simulink library "outp"  (R2021b)
(part 7 of 8)

  VOUTP_LFWheelDebug_flg : Outport  Port=593
  VOUTP_LRWheelDebug_flg : Outport  Port=594
  VOUTP_RFWheelDebug_flg : Outport  Port=595
  VOUTP_RRWheelDebug_flg : Outport  Port=596
  VOUTP_TPMSResButtAllow_flg : Outport  Port=597
  VOUTP_TPMSCaliButtAllow_flg : Outport  Port=598
  VOUTP_LFPressIndi_enum : Outport  Port=599
  VOUTP_RFPressIndi_enum : Outport  Port=600
  VOUTP_LRPressIndi_enum : Outport  Port=601
  VOUTP_RRPressIndi_enum : Outport  Port=602
  VOUTP_TPMSWarnIndi_enum : Outport  Port=603
  VOUTP_LFWheelTmpIndi_flg : Outport  Port=604
  VOUTP_RFWheelTmpIndi_flg : Outport  Port=605
  VOUTP_LRWheelTmpIndi_flg : Outport  Port=606
  VOUTP_RRWheelTmpIndi_flg : Outport  Port=607
  VOUTP_LFWheelPSW_raw8 : Outport  Port=608
  VOUTP_LRWheelPSW_raw8 : Outport  Port=609
  VOUTP_RFWheelPSW_raw8 : Outport  Port=610
  VOUTP_RRWheelPSW_raw8 : Outport  Port=611
  VOUTP_CWheelTips_enum : Outport  Port=612
  VOUTP_AutoLTips_enum : Outport  Port=613
  VOUTP_LFSensorMode_flg : Outport  Port=614
  VOUTP_RFSensorMode_flg : Outport  Port=615
  VOUTP_LRSensorMode_flg : Outport  Port=616
  VOUTP_RRSensorMode_flg : Outport  Port=617
  VOUTP_S1ID_raw32 : Outport  Port=618
  VOUTP_S2ID_raw32 : Outport  Port=619
  VOUTP_S3ID_raw32 : Outport  Port=620
  VOUTP_S4ID_raw32 : Outport  Port=621
  VOUTP_S1L_enum : Outport  Port=622
  VOUTP_S2L_enum : Outport  Port=623
  VOUTP_S3L_enum : Outport  Port=624
  VOUTP_S4L_enum : Outport  Port=625
  VOUTP_ALFin_flg : Outport  Port=626
  VOUTP_LFP20_raw8 : Outport  Port=627
  VOUTP_RFP20_raw8 : Outport  Port=628
  VOUTP_LRP20_raw8 : Outport  Port=629
  VOUTP_RRP20_raw8 : Outport  Port=630
  VOUTP_FAT_flg : Outport  Port=631
  VOUTP_IDin_raw32 : Outport  Port=632
  VOUTP_S1WheelDebugALTU_pct : Outport  Port=633
  VOUTP_S2WheelDebugALTU_pct : Outport  Port=634
  VOUTP_S3WheelDebugALTU_pct : Outport  Port=635
  VOUTP_S4WheelDebugALTU_pct : Outport  Port=636
  VOUTP_ID1messageALTU_raw8 : Outport  Port=637
  VOUTP_ID2messageALTU_raw8 : Outport  Port=638
  VOUTP_ID3messageALTU_raw8 : Outport  Port=639
  VOUTP_ID4messageALTU_raw8 : Outport  Port=640
  VOUTP_Chkfin_flg : Outport  Port=641
  VOUTP_SetIDLoc_flg : Outport  Port=642
  VOUTP_TPMSStorge_flg : Outport  Port=643
  VOUTP_ChkStorge_flg : Outport  Port=644
  VOUTP_TPMSResButt_flg : Outport  Port=645
  VOUTP_LFPindi_enum : Outport  Port=646
  VOUTP_RFPind_enum : Outport  Port=647
  VOUTP_LRPindi_enum : Outport  Port=648
  VOUTP_RRPindi_enum : Outport  Port=649
  VOUTP_WriteChkLFID_raw : Outport  Port=650
  VOUTP_WriteChkRFID_raw : Outport  Port=651
  VOUTP_WriteChkLRID_raw : Outport  Port=652
  VOUTP_WriteChkRRID_raw : Outport  Port=653
  VOUTP_WriteChkfinLFID_raw : Outport  Port=654
  VOUTP_WriteChkfinRFID_raw : Outport  Port=655
  VOUTP_WriteChkfinLRID_raw : Outport  Port=656
  VOUTP_WriteChkfinRRID_raw : Outport  Port=657
  VOUTP_Flashchkdatavalid_enum : Outport  Port=658
  VOUTP_Flashdatavalid_enum : Outport  Port=659
  VOUTP_unlearnSfali_flg : Outport  Port=660
  VOUTP_unlearnSfailvalid_enum : Outport  Port=661
  VOUTP_Prepresstempvalid_enum : Outport  Port=662
  VOUTP_FlashS1ID_raw : Outport  Port=663
  VOUTP_FlashS2ID_raw : Outport  Port=664
  VOUTP_FlashS3ID_raw : Outport  Port=665
  VOUTP_FlashS4ID_raw : Outport  Port=666
  VOUTP_FlashIDvalid_enum : Outport  Port=667
  VOUTP_WritingCnt_enum : Outport  Port=668
  VOUTP_TPMSTLCmd_flg : Outport  Port=669
  VOUTP_LProgress_enum : Outport  Port=670
  VOUTP_TPMSSensorIDRegStart_flg : Outport  Port=671
  VOUTP_ModelVersion_raw : Outport  Port=672
  VOUTP_ModelVersionChksum_raw : Outport  Port=673
  VOUTP_ParkRequest_flg : Outport  Port=674
  VOUTP_TqSourceFr_enum : Outport  Port=675
  VOUTP_TqSourceRr_enum : Outport  Port=676
  VOUTP_FrEDUAvailBrkRgnTq_Nm : Outport  Port=677
  VOUTP_RrEDUAvailBrkRgnTq_Nm : Outport  Port=678
  VOUTP_EVDriveMode_enum : Outport  Port=679
  VOUTP_ShiftGearPosn_enum : Outport  Port=680
  VOUTP_PButtonSta_enum : Outport  Port=681
  VOUTP_FrActvDmpDisabReq_flg : Outport  Port=682
  VOUTP_RrActvDmpDisabReq_flg : Outport  Port=683
  VOUTP_FrRgnDecrSta_flg : Outport  Port=684
  VOUTP_RrRgnDecrSta_flg : Outport  Port=685
  VOUTP_DriverWhlTqDemFr_Nm : Outport  Port=686
  VOUTP_DriverWhlTqDemRr_Nm : Outport  Port=687
  VOUTP_FrEDUActTq_Nm : Outport  Port=688
  VOUTP_RrEDUActTq_Nm : Outport  Port=689
  VOUTP_FrEDURolRgnTq_Nm : Outport  Port=690
  VOUTP_RrEDURolRgnTq_Nm : Outport  Port=691
  VOUTP_FrEDUSpd_rpm : Outport  Port=692
  VOUTP_RrEDUSpd_rpm : Outport  Port=693
  VOUTP_FrEDUSpdValid_flg : Outport  Port=694
  VOUTP_FrEDUAvailBrkRgnTqV_flg : Outport  Port=695
  VOUTP_RrEDUSpdValid_flg : Outport  Port=696
  VOUTP_RrEDUAvailBrkRgnTqV_flg : Outport  Port=697
  VOUTP_RgnAbnorSta_flg : Outport  Port=698
  VOUTP_PTCSPermSta_flg : Outport  Port=699
  VOUTP_FrRgnPermSta_flg : Outport  Port=700
  VOUTP_RrRgnPermSta_flg : Outport  Port=701
  VOUTP_FrIdcMin_A : Outport  Port=702
  VOUTP_FrIdcMax_A : Outport  Port=703
  VOUTP_FrUdcMin_V : Outport  Port=704
  VOUTP_FrUdcMax_V : Outport  Port=705
  VOUTP_RrIdcMin_A : Outport  Port=706
  VOUTP_RrIdcMax_A : Outport  Port=707
  VOUTP_RrUdcMin_V : Outport  Port=708
  VOUTP_RrUdcMax_V : Outport  Port=709
  VOUTP_ReBrakeLPReq_flg : Outport  Port=710
  VOUTP_CreepON_flg : Outport  Port=711
  VOUTP_EquivAccPedalSWSta_flg : Outport  Port=712
  VOUTP_DriveProtEn_flg : Outport  Port=713
  VOUTP_ActParkRequest_flg : Outport  Port=714
  VOUTP_IVIPwrLockSta_enum : Outport  Port=715
  VOUTP_OPDHoldLamp_flg : Outport  Port=716
  VOUTP_VehActSpd_kph : Outport  Port=717
  VOUTP_FrTMTqReq_Nm : Outport  Port=718
  VOUTP_RrTMTqReq_Nm : Outport  Port=719
  VOUTP_ReqOBCV2LEna_enum : Outport  Port=720
  VOUTP_ReqV2LIVIPopup_enum : Outport  Port=721
  VOUTP_ACCCtrlAvail_flg : Outport  Port=722
  VOUTP_ACCPedalOvrd_flg : Outport  Port=723
  VOUTP_CCCtrlSta_enum : Outport  Port=724
  VOUTP_CCMSASpdWar_flg : Outport  Port=725
  VOUTP_MSACtrlSta_enum : Outport  Port=726
  VOUTP_APSCtrlAvail_flg : Outport  Port=727
  VOUTP_APSActive_flg : Outport  Port=728
  VOUTP_APSStaSys_enum : Outport  Port=729
  VOUTP_APSDecReqA_flg : Outport  Port=730
  VOUTP_APSDecReq_mps2 : Outport  Port=731
  VOUTP_APSReq_enum : Outport  Port=732
  VOUTP_IMUEnaCmd_flg : Outport  Port=733
  VOUTP_CAASCtrlAvail_flg : Outport  Port=734
  VOUTP_CAASActive_flg : Outport  Port=735
  VOUTP_ExtraMSACtrlSta_enum : Outport  Port=736
  wires:
  VACC_HVTHCMSysAvail_enum/1 -> VACC_HVTHCMSysAvail_enum_Inproc/1  "VACC_HVTHCMSysAvail_enum"
  VACC_HVTHCMSysAvail_enum_Inproc/1 -> UnitConverter1/1
  UnitConverter1/1 -> VOUTP_HVTHCMSysAvail_enum/1  "VOUTP_HVTHCMSysAvail_enum"
  VACC_LVBattVoltSta_enum/1 -> VACC_LVBattVoltSta_enum_Inproc/1  "VACC_LVBattVoltSta_enum"
  VACC_LVBattVoltSta_enum_Inproc/1 -> UnitConverter2/1
  UnitConverter2/1 -> VOUTP_LVBattVoltSta_enum/1  "VOUTP_LVBattVoltSta_enum"
  VACC_VehHVPwrAvail4THCM_W/1 -> VACC_VehHVPwrAvail4THCM_W_Inproc/1  "VACC_VehHVPwrAvail4THCM_W"
  VACC_VehHVPwrAvail4THCM_W_Inproc/1 -> UnitConverter3/1
  UnitConverter3/1 -> VOUTP_VehHVPwrAvail4THCM_W/1  "VOUTP_VehHVPwrAvail4THCM_W"
  VAPM_VehSpeed_kph/1 -> VAPM_VehSpeed_kph_Inproc/1  "VAPM_VehSpeed_kph"
  VAPM_VehSpeed_kph_Inproc/1 -> UnitConverter4/1
  UnitConverter4/1 -> VOUTP_VehSpeed_kph/1  "VOUTP_VehSpeed_kph"
  VAPM_VehSpeedTimeOut_flg/1 -> VAPM_VehSpeedTimeOut_flg_Inproc/1  "VAPM_VehSpeedTimeOut_flg"
  VAPM_VehSpeedTimeOut_flg_Inproc/1 -> UnitConverter5/1
  UnitConverter5/1 -> VOUTP_VehSpeedTimeOut_flg/1  "VOUTP_VehSpeedTimeOut_flg"
  VAPM_FSOffSw_enum/1 -> VAPM_FSOffSw_enum_Inproc/1  "VAPM_FSOffSw_enum"
  VAPM_FSOffSw_enum_Inproc/1 -> UnitConverter6/1
  UnitConverter6/1 -> VOUTP_FSOffSw_enum/1  "VOUTP_FSOffSw_enum"
  VAPM_FSOffSwTimeOut_flg/1 -> VAPM_FSOffSwTimeOut_flg_Inproc/1  "VAPM_FSOffSwTimeOut_flg"
  VAPM_FSOffSwTimeOut_flg_Inproc/1 -> UnitConverter7/1
  UnitConverter7/1 -> VOUTP_FSOffSwTimeOut_flg/1  "VOUTP_FSOffSwTimeOut_flg"
  VAPM_ChrgPlugSta_enum/1 -> VAPM_ChrgPlugSta_enum_Inproc/1  "VAPM_ChrgPlugSta_enum"
  VAPM_ChrgPlugSta_enum_Inproc/1 -> UnitConverter8/1
  UnitConverter8/1 -> VOUTP_ChrgPlugSta_enum/1  "VOUTP_ChrgPlugSta_enum"
  VAPM_PASDRMR_cm/1 -> VAPM_PASDRMR_cm_Inproc/1  "VAPM_PASDRMR_cm"
  VAPM_PASDRMR_cm_Inproc/1 -> UnitConverter9/1
  UnitConverter9/1 -> VOUTP_PASDRMR_cm/1  "VOUTP_PASDRMR_cm"
  VAPM_PASDRML_cm/1 -> VAPM_PASDRML_cm_Inproc/1  "VAPM_PASDRML_cm"
  VAPM_PASDRML_cm_Inproc/1 -> UnitConverter10/1
  UnitConverter10/1 -> VOUTP_PASDRML_cm/1  "VOUTP_PASDRML_cm"
  VAPM_PASDRCR_cm/1 -> VAPM_PASDRCR_cm_Inproc/1  "VAPM_PASDRCR_cm"
  VAPM_PASDRCR_cm_Inproc/1 -> UnitConverter11/1
  UnitConverter11/1 -> VOUTP_PASDRCR_cm/1  "VOUTP_PASDRCR_cm"
  VAPM_PASDRCL_cm/1 -> VAPM_PASDRCL_cm_Inproc/1  "VAPM_PASDRCL_cm"
  VAPM_PASDRCL_cm_Inproc/1 -> UnitConverter12/1
  UnitConverter12/1 -> VOUTP_PASDRCL_cm/1  "VOUTP_PASDRCL_cm"
  VAPM_PASDFMR_cm/1 -> VAPM_PASDFMR_cm_Inproc/1  "VAPM_PASDFMR_cm"
  VAPM_PASDFMR_cm_Inproc/1 -> UnitConverter13/1
  UnitConverter13/1 -> VOUTP_PASDFMR_cm/1  "VOUTP_PASDFMR_cm"
  VAPM_PASDFML_cm/1 -> VAPM_PASDFML_cm_Inproc/1  "VAPM_PASDFML_cm"
  VAPM_PASDFML_cm_Inproc/1 -> UnitConverter14/1
  UnitConverter14/1 -> VOUTP_PASDFML_cm/1  "VOUTP_PASDFML_cm"
  VAPM_PASDFCR_cm/1 -> VAPM_PASDFCR_cm_Inproc/1  "VAPM_PASDFCR_cm"
  VAPM_PASDFCR_cm_Inproc/1 -> UnitConverter15/1
  UnitConverter15/1 -> VOUTP_PASDFCR_cm/1  "VOUTP_PASDFCR_cm"
  VAPM_PASDFCL_cm/1 -> VAPM_PASDFCL_cm_Inproc/1  "VAPM_PASDFCL_cm"
  VAPM_PASDFCL_cm_Inproc/1 -> UnitConverter16/1
  UnitConverter16/1 -> VOUTP_PASDFCL_cm/1  "VOUTP_PASDFCL_cm"
  VAPM_APSDRLR_cm/1 -> VAPM_APSDRLR_cm_Inproc/1  "VAPM_APSDRLR_cm"
  VAPM_APSDRLR_cm_Inproc/1 -> UnitConverter17/1
  UnitConverter17/1 -> VOUTP_APSDRLR_cm/1  "VOUTP_APSDRLR_cm"
  VAPM_APSDRLL_cm/1 -> VAPM_APSDRLL_cm_Inproc/1  "VAPM_APSDRLL_cm"
  VAPM_APSDRLL_cm_Inproc/1 -> UnitConverter18/1
  UnitConverter18/1 -> VOUTP_APSDRLL_cm/1  "VOUTP_APSDRLL_cm"
  VAPM_APSDFLR_cm/1 -> VAPM_APSDFLR_cm_Inproc/1  "VAPM_APSDFLR_cm"
  VAPM_APSDFLR_cm_Inproc/1 -> UnitConverter19/1
  UnitConverter19/1 -> VOUTP_APSDFLR_cm/1  "VOUTP_APSDFLR_cm"
  VAPM_APSDFLL_cm/1 -> VAPM_APSDFLL_cm_Inproc/1  "VAPM_APSDFLL_cm"
  VAPM_APSDFLL_cm_Inproc/1 -> UnitConverter20/1
  UnitConverter20/1 -> VOUTP_APSDFLL_cm/1  "VOUTP_APSDFLL_cm"
  VAPM_PASAFCL_enum/1 -> VAPM_PASAFCL_enum_Inproc/1  "VAPM_PASAFCL_enum"
  VAPM_PASAFCL_enum_Inproc/1 -> UnitConverter21/1
  UnitConverter21/1 -> VOUTP_PASAFCL_enum/1  "VOUTP_PASAFCL_enum"
  VAPM_PASARMR_enum/1 -> VAPM_PASARMR_enum_Inproc/1  "VAPM_PASARMR_enum"
  VAPM_PASARMR_enum_Inproc/1 -> UnitConverter22/1
  UnitConverter22/1 -> VOUTP_PASARMR_enum/1  "VOUTP_PASARMR_enum"
  VAPM_PASARML_enum/1 -> VAPM_PASARML_enum_Inproc/1  "VAPM_PASARML_enum"
  VAPM_PASARML_enum_Inproc/1 -> UnitConverter23/1
  UnitConverter23/1 -> VOUTP_PASARML_enum/1  "VOUTP_PASARML_enum"
  VAPM_PASARCR_enum/1 -> VAPM_PASARCR_enum_Inproc/1  "VAPM_PASARCR_enum"
  VAPM_PASARCR_enum_Inproc/1 -> UnitConverter24/1
  UnitConverter24/1 -> VOUTP_PASARCR_enum/1  "VOUTP_PASARCR_enum"
  VAPM_PASARCL_enum/1 -> VAPM_PASARCL_enum_Inproc/1  "VAPM_PASARCL_enum"
  VAPM_PASARCL_enum_Inproc/1 -> UnitConverter25/1
  UnitConverter25/1 -> VOUTP_PASARCL_enum/1  "VOUTP_PASARCL_enum"
  VAPM_PASAFMR_enum/1 -> VAPM_PASAFMR_enum_Inproc/1  "VAPM_PASAFMR_enum"
  VAPM_PASAFMR_enum_Inproc/1 -> UnitConverter26/1
  UnitConverter26/1 -> VOUTP_PASAFMR_enum/1  "VOUTP_PASAFMR_enum"
  VAPM_PASAFML_enum/1 -> VAPM_PASAFML_enum_Inproc/1  "VAPM_PASAFML_enum"
  VAPM_PASAFML_enum_Inproc/1 -> UnitConverter27/1
  UnitConverter27/1 -> VOUTP_PASAFML_enum/1  "VOUTP_PASAFML_enum"
  VAPM_PASAFCR_enum/1 -> VAPM_PASAFCR_enum_Inproc/1  "VAPM_PASAFCR_enum"
  VAPM_PASAFCR_enum_Inproc/1 -> UnitConverter28/1
  UnitConverter28/1 -> VOUTP_PASAFCR_enum/1  "VOUTP_PASAFCR_enum"
  VAPM_USSStaRMR_flg/1 -> VAPM_USSStaRMR_flg_Inproc/1  "VAPM_USSStaRMR_flg"
  VAPM_USSStaRMR_flg_Inproc/1 -> UnitConverter29/1
  UnitConverter29/1 -> VOUTP_USSStaRMR_flg/1  "VOUTP_USSStaRMR_flg"
  VAPM_USSStaRML_flg/1 -> VAPM_USSStaRML_flg_Inproc/1  "VAPM_USSStaRML_flg"
  VAPM_USSStaRML_flg_Inproc/1 -> UnitConverter30/1
  UnitConverter30/1 -> VOUTP_USSStaRML_flg/1  "VOUTP_USSStaRML_flg"
  VAPM_USSStaRLR_flg/1 -> VAPM_USSStaRLR_flg_Inproc/1  "VAPM_USSStaRLR_flg"
  VAPM_USSStaRLR_flg_Inproc/1 -> UnitConverter31/1
  UnitConverter31/1 -> VOUTP_USSStaRLR_flg/1  "VOUTP_USSStaRLR_flg"
  VAPM_USSStaRLL_flg/1 -> VAPM_USSStaRLL_flg_Inproc/1  "VAPM_USSStaRLL_flg"
  VAPM_USSStaRLL_flg_Inproc/1 -> UnitConverter32/1
  UnitConverter32/1 -> VOUTP_USSStaRLL_flg/1  "VOUTP_USSStaRLL_flg"
  VAPM_USSStaRCR_flg/1 -> VAPM_USSStaRCR_flg_Inproc/1  "VAPM_USSStaRCR_flg"
  VAPM_USSStaRCR_flg_Inproc/1 -> UnitConverter33/1
  UnitConverter33/1 -> VOUTP_USSStaRCR_flg/1  "VOUTP_USSStaRCR_flg"
  VAPM_USSStaRCL_flg/1 -> VAPM_USSStaRCL_flg_Inproc/1  "VAPM_USSStaRCL_flg"
  VAPM_USSStaRCL_flg_Inproc/1 -> UnitConverter34/1
  UnitConverter34/1 -> VOUTP_USSStaRCL_flg/1  "VOUTP_USSStaRCL_flg"
  VAPM_USSStaFMR_flg/1 -> VAPM_USSStaFMR_flg_Inproc/1  "VAPM_USSStaFMR_flg"
  VAPM_USSStaFMR_flg_Inproc/1 -> UnitConverter35/1
  UnitConverter35/1 -> VOUTP_USSStaFMR_flg/1  "VOUTP_USSStaFMR_flg"
  VAPM_USSStaFML_flg/1 -> VAPM_USSStaFML_flg_Inproc/1  "VAPM_USSStaFML_flg"
  VAPM_USSStaFML_flg_Inproc/1 -> UnitConverter36/1
  UnitConverter36/1 -> VOUTP_USSStaFML_flg/1  "VOUTP_USSStaFML_flg"
  VAPM_USSStaFLR_flg/1 -> VAPM_USSStaFLR_flg_Inproc/1  "VAPM_USSStaFLR_flg"
  VAPM_USSStaFLR_flg_Inproc/1 -> UnitConverter37/1
  UnitConverter37/1 -> VOUTP_USSStaFLR_flg/1  "VOUTP_USSStaFLR_flg"
  VAPM_USSStaFLL_flg/1 -> VAPM_USSStaFLL_flg_Inproc/1  "VAPM_USSStaFLL_flg"
  VAPM_USSStaFLL_flg_Inproc/1 -> UnitConverter38/1
  UnitConverter38/1 -> VOUTP_USSStaFLL_flg/1  "VOUTP_USSStaFLL_flg"
  VAPM_USSStaFCR_flg/1 -> VAPM_USSStaFCR_flg_Inproc/1  "VAPM_USSStaFCR_flg"
  VAPM_USSStaFCR_flg_Inproc/1 -> UnitConverter39/1
  UnitConverter39/1 -> VOUTP_USSStaFCR_flg/1  "VOUTP_USSStaFCR_flg"
  VAPM_USSStaFCL_flg/1 -> VAPM_USSStaFCL_flg_Inproc/1  "VAPM_USSStaFCL_flg"
  VAPM_USSStaFCL_flg_Inproc/1 -> UnitConverter40/1
  UnitConverter40/1 -> VOUTP_USSStaFCL_flg/1  "VOUTP_USSStaFCL_flg"
  VAPM_Chime_enum/1 -> VAPM_Chime_enum_Inproc/1  "VAPM_Chime_enum"
  VAPM_Chime_enum_Inproc/1 -> UnitConverter41/1
  UnitConverter41/1 -> VOUTP_Chime_enum/1  "VOUTP_Chime_enum"
  VAPM_SNSRLayout_enum/1 -> VAPM_SNSRLayout_enum_Inproc/1  "VAPM_SNSRLayout_enum"
  VAPM_SNSRLayout_enum_Inproc/1 -> UnitConverter42/1
  UnitConverter42/1 -> VOUTP_SNSRLayout_enum/1  "VOUTP_SNSRLayout_enum"
  VAPM_StaFSya_flg/1 -> VAPM_StaFSya_flg_Inproc/1  "VAPM_StaFSya_flg"
  VAPM_StaFSya_flg_Inproc/1 -> UnitConverter43/1
  UnitConverter43/1 -> VOUTP_StaFSya_flg/1  "VOUTP_StaFSya_flg"
  VAPM_ModOperation_enum/1 -> VAPM_ModOperation_enum_Inproc/1  "VAPM_ModOperation_enum"
  VAPM_ModOperation_enum_Inproc/1 -> UnitConverter44/1
  UnitConverter44/1 -> VOUTP_ModOperation_enum/1  "VOUTP_ModOperation_enum"
  VAPM_BrkPedalPos_pct/1 -> VAPM_BrkPedalPos_pct_Inproc/1  "VAPM_BrkPedalPos_pct"
  VAPM_BrkPedalPos_pct_Inproc/1 -> UnitConverter45/1
  UnitConverter45/1 -> VOUTP_BrkPedalPos_pct/1  "VOUTP_BrkPedalPos_pct"
  VAPM_BrkPedalPosTimeOut_flg/1 -> VAPM_BrkPedalPosTimeOut_flg_Inproc/1  "VAPM_BrkPedalPosTimeOut_flg"
  VAPM_BrkPedalPosTimeOut_flg_Inproc/1 -> UnitConverter46/1
  UnitConverter46/1 -> VOUTP_BrkPedalPosTimeOut_flg/1  "VOUTP_BrkPedalPosTimeOut_flg"
  VAPM_LFRawWhlSpeed_kph/1 -> VAPM_LFRawWhlSpeed_kph_Inproc/1  "VAPM_LFRawWhlSpeed_kph"
  VAPM_LFRawWhlSpeed_kph_Inproc/1 -> UnitConverter47/1
  UnitConverter47/1 -> VOUTP_LFRawWhlSpeed_kph/1  "VOUTP_LFRawWhlSpeed_kph"
  VAPM_LFRawWhlSpeedTimeOut_flg/1 -> VAPM_LFRawWhlSpeedTimeOut_flg_Inproc/1  "VAPM_LFRawWhlSpeedTimeOut_flg"
  VAPM_LFRawWhlSpeedTimeOut_flg_Inproc/1 -> UnitConverter48/1
  UnitConverter48/1 -> VOUTP_LFRawWhlSpeedTimeOut_flg/1  "VOUTP_LFRawWhlSpeedTimeOut_flg"
  VAPM_RFRawWhlSpeed_kph/1 -> VAPM_RFRawWhlSpeed_kph_Inproc/1  "VAPM_RFRawWhlSpeed_kph"
  VAPM_RFRawWhlSpeed_kph_Inproc/1 -> UnitConverter49/1
  UnitConverter49/1 -> VOUTP_RFRawWhlSpeed_kph/1  "VOUTP_RFRawWhlSpeed_kph"
  VAPM_RFRawWhlSpeedTimeOut_flg/1 -> VAPM_RFRawWhlSpeedTimeOut_flg_Inproc/1  "VAPM_RFRawWhlSpeedTimeOut_flg"
  VAPM_RFRawWhlSpeedTimeOut_flg_Inproc/1 -> UnitConverter50/1
  UnitConverter50/1 -> VOUTP_RFRawWhlSpeedTimeOut_flg/1  "VOUTP_RFRawWhlSpeedTimeOut_flg"
  VAPM_LRRawWhlSpeed_kph/1 -> VAPM_LRRawWhlSpeed_kph_Inproc/1  "VAPM_LRRawWhlSpeed_kph"
  VAPM_LRRawWhlSpeed_kph_Inproc/1 -> UnitConverter51/1
  UnitConverter51/1 -> VOUTP_LRRawWhlSpeed_kph/1  "VOUTP_LRRawWhlSpeed_kph"
  VAPM_LRRawWhlSpeedTimeOut_flg/1 -> VAPM_LRRawWhlSpeedTimeOut_flg_Inproc/1  "VAPM_LRRawWhlSpeedTimeOut_flg"
  VAPM_LRRawWhlSpeedTimeOut_flg_Inproc/1 -> UnitConverter52/1
  UnitConverter52/1 -> VOUTP_LRRawWhlSpeedTimeOut_flg/1  "VOUTP_LRRawWhlSpeedTimeOut_flg"
  VAPM_RRRawWhlSpeed_kph/1 -> VAPM_RRRawWhlSpeed_kph_Inproc/1  "VAPM_RRRawWhlSpeed_kph"
  VAPM_RRRawWhlSpeed_kph_Inproc/1 -> UnitConverter53/1
  UnitConverter53/1 -> VOUTP_RRRawWhlSpeed_kph/1  "VOUTP_RRRawWhlSpeed_kph"
  VAPM_RRRawWhlSpeedTimeOut_flg/1 -> VAPM_RRRawWhlSpeedTimeOut_flg_Inproc/1  "VAPM_RRRawWhlSpeedTimeOut_flg"
  VAPM_RRRawWhlSpeedTimeOut_flg_Inproc/1 -> UnitConverter54/1
  UnitConverter54/1 -> VOUTP_RRRawWhlSpeedTimeOut_flg/1  "VOUTP_RRRawWhlSpeedTimeOut_flg"
  VAPM_LFRawWhlSpeedV_flg/1 -> VAPM_LFRawWhlSpeedV_flg_Inproc/1  "VAPM_LFRawWhlSpeedV_flg"
  VAPM_LFRawWhlSpeedV_flg_Inproc/1 -> UnitConverter55/1
  UnitConverter55/1 -> VOUTP_LFRawWhlSpeedV_flg/1  "VOUTP_LFRawWhlSpeedV_flg"
  VAPM_LFRawWhlSpeedVTimeOut_flg/1 -> VAPM_LFRawWhlSpeedVTimeOut_flg_Inproc/1  "VAPM_LFRawWhlSpeedVTimeOut_flg"
  VAPM_LFRawWhlSpeedVTimeOut_flg_Inproc/1 -> UnitConverter56/1
  UnitConverter56/1 -> VOUTP_LFRawWhlSpeedVTimeOut_flg/1  "VOUTP_LFRawWhlSpeedVTimeOut_flg"
  VAPM_RFRawWhlSpeedV_flg/1 -> VAPM_RFRawWhlSpeedV_flg_Inproc/1  "VAPM_RFRawWhlSpeedV_flg"
  VAPM_RFRawWhlSpeedV_flg_Inproc/1 -> UnitConverter57/1
  UnitConverter57/1 -> VOUTP_RFRawWhlSpeedV_flg/1  "VOUTP_RFRawWhlSpeedV_flg"
  VAPM_RFRawWhlSpeedVTimeOut_flg/1 -> VAPM_RFRawWhlSpeedVTimeOut_flg_Inproc/1  "VAPM_RFRawWhlSpeedVTimeOut_flg"
  VAPM_RFRawWhlSpeedVTimeOut_flg_Inproc/1 -> UnitConverter58/1
  UnitConverter58/1 -> VOUTP_RFRawWhlSpeedVTimeOut_flg/1  "VOUTP_RFRawWhlSpeedVTimeOut_flg"
  VAPM_LRRawWhlSpeedV_flg/1 -> VAPM_LRRawWhlSpeedV_flg_Inproc/1  "VAPM_LRRawWhlSpeedV_flg"
  VAPM_LRRawWhlSpeedV_flg_Inproc/1 -> UnitConverter59/1
  UnitConverter59/1 -> VOUTP_LRRawWhlSpeedV_flg/1  "VOUTP_LRRawWhlSpeedV_flg"
  VAPM_LRRawWhlSpeedVTimeOut_flg/1 -> VAPM_LRRawWhlSpeedVTimeOut_flg_Inproc/1  "VAPM_LRRawWhlSpeedVTimeOut_flg"
  VAPM_LRRawWhlSpeedVTimeOut_flg_Inproc/1 -> UnitConverter60/1
  UnitConverter60/1 -> VOUTP_LRRawWhlSpeedVTimeOut_flg/1  "VOUTP_LRRawWhlSpeedVTimeOut_flg"
  VAPM_RRRawWhlSpeedV_flg/1 -> VAPM_RRRawWhlSpeedV_flg_Inproc/1  "VAPM_RRRawWhlSpeedV_flg"
  VAPM_RRRawWhlSpeedV_flg_Inproc/1 -> UnitConverter61/1
  UnitConverter61/1 -> VOUTP_RRRawWhlSpeedV_flg/1  "VOUTP_RRRawWhlSpeedV_flg"
  VAPM_RRRawWhlSpeedVTimeOut_flg/1 -> VAPM_RRRawWhlSpeedVTimeOut_flg_Inproc/1  "VAPM_RRRawWhlSpeedVTimeOut_flg"
  VAPM_RRRawWhlSpeedVTimeOut_flg_Inproc/1 -> UnitConverter62/1
  UnitConverter62/1 -> VOUTP_RRRawWhlSpeedVTimeOut_flg/1  "VOUTP_RRRawWhlSpeedVTimeOut_flg"
  VAPM_LFWhlRotDir_enum/1 -> VAPM_LFWhlRotDir_enum_Inproc/1  "VAPM_LFWhlRotDir_enum"
  VAPM_LFWhlRotDir_enum_Inproc/1 -> UnitConverter63/1
  UnitConverter63/1 -> VOUTP_LFWhlRotDir_enum/1  "VOUTP_LFWhlRotDir_enum"
  VAPM_LFWhlRotDirTimeOut_flg/1 -> VAPM_LFWhlRotDirTimeOut_flg_Inproc/1  "VAPM_LFWhlRotDirTimeOut_flg"
  VAPM_LFWhlRotDirTimeOut_flg_Inproc/1 -> UnitConverter64/1
  UnitConverter64/1 -> VOUTP_LFWhlRotDirTimeOut_flg/1  "VOUTP_LFWhlRotDirTimeOut_flg"
  VAPM_RFWhlRotDir_enum/1 -> VAPM_RFWhlRotDir_enum_Inproc/1  "VAPM_RFWhlRotDir_enum"
  VAPM_RFWhlRotDir_enum_Inproc/1 -> UnitConverter65/1
  UnitConverter65/1 -> VOUTP_RFWhlRotDir_enum/1  "VOUTP_RFWhlRotDir_enum"
  VAPM_RFWhlRotDirTimeOut_flg/1 -> VAPM_RFWhlRotDirTimeOut_flg_Inproc/1  "VAPM_RFWhlRotDirTimeOut_flg"
  VAPM_RFWhlRotDirTimeOut_flg_Inproc/1 -> UnitConverter66/1
  UnitConverter66/1 -> VOUTP_RFWhlRotDirTimeOut_flg/1  "VOUTP_RFWhlRotDirTimeOut_flg"
  VAPM_LRWhlRotDir_enum/1 -> VAPM_LRWhlRotDir_enum_Inproc/1  "VAPM_LRWhlRotDir_enum"
  VAPM_LRWhlRotDir_enum_Inproc/1 -> UnitConverter67/1
  UnitConverter67/1 -> VOUTP_LRWhlRotDir_enum/1  "VOUTP_LRWhlRotDir_enum"
  VAPM_LRWhlRotDirTimeOut_flg/1 -> VAPM_LRWhlRotDirTimeOut_flg_Inproc/1  "VAPM_LRWhlRotDirTimeOut_flg"
  VAPM_LRWhlRotDirTimeOut_flg_Inproc/1 -> UnitConverter68/1
  UnitConverter68/1 -> VOUTP_LRWhlRotDirTimeOut_flg/1  "VOUTP_LRWhlRotDirTimeOut_flg"
  VAPM_RRWhlRotDir_enum/1 -> VAPM_RRWhlRotDir_enum_Inproc/1  "VAPM_RRWhlRotDir_enum"
  VAPM_RRWhlRotDir_enum_Inproc/1 -> UnitConverter69/1
  UnitConverter69/1 -> VOUTP_RRWhlRotDir_enum/1  "VOUTP_RRWhlRotDir_enum"
  VAPM_RRWhlRotDirTimeOut_flg/1 -> VAPM_RRWhlRotDirTimeOut_flg_Inproc/1  "VAPM_RRWhlRotDirTimeOut_flg"
  VAPM_RRWhlRotDirTimeOut_flg_Inproc/1 -> UnitConverter70/1
  UnitConverter70/1 -> VOUTP_RRWhlRotDirTimeOut_flg/1  "VOUTP_RRWhlRotDirTimeOut_flg"
  VAPM_LFPulseCountV_flg/1 -> VAPM_LFPulseCountV_flg_Inproc/1  "VAPM_LFPulseCountV_flg"
  VAPM_LFPulseCountV_flg_Inproc/1 -> UnitConverter71/1
  UnitConverter71/1 -> VOUTP_LFPulseCountV_flg/1  "VOUTP_LFPulseCountV_flg"
  VAPM_LFPulseCountVTimeOut_flg/1 -> VAPM_LFPulseCountVTimeOut_flg_Inproc/1  "VAPM_LFPulseCountVTimeOut_flg"
  VAPM_LFPulseCountVTimeOut_flg_Inproc/1 -> UnitConverter72/1
  UnitConverter72/1 -> VOUTP_LFPulseCountVTimeOut_flg/1  "VOUTP_LFPulseCountVTimeOut_flg"
  VAPM_RFPulseCountV_flg/1 -> VAPM_RFPulseCountV_flg_Inproc/1  "VAPM_RFPulseCountV_flg"
  VAPM_RFPulseCountV_flg_Inproc/1 -> UnitConverter73/1
  UnitConverter73/1 -> VOUTP_RFPulseCountV_flg/1  "VOUTP_RFPulseCountV_flg"
  VAPM_RFPulseCountVTimeOut_flg/1 -> VAPM_RFPulseCountVTimeOut_flg_Inproc/1  "VAPM_RFPulseCountVTimeOut_flg"
  VAPM_RFPulseCountVTimeOut_flg_Inproc/1 -> UnitConverter74/1
  UnitConverter74/1 -> VOUTP_RFPulseCountVTimeOut_flg/1  "VOUTP_RFPulseCountVTimeOut_flg"
  VAPM_LRPulseCountV_flg/1 -> VAPM_LRPulseCountV_flg_Inproc/1  "VAPM_LRPulseCountV_flg"
  VAPM_LRPulseCountV_flg_Inproc/1 -> UnitConverter75/1
  UnitConverter75/1 -> VOUTP_LRPulseCountV_flg/1  "VOUTP_LRPulseCountV_flg"
  VAPM_LRPulseCountVTimeOut_flg/1 -> VAPM_LRPulseCountVTimeOut_flg_Inproc/1  "VAPM_LRPulseCountVTimeOut_flg"
  VAPM_LRPulseCountVTimeOut_flg_Inproc/1 -> UnitConverter76/1
  UnitConverter76/1 -> VOUTP_LRPulseCountVTimeOut_flg/1  "VOUTP_LRPulseCountVTimeOut_flg"
  VAPM_RRPulseCountV_flg/1 -> VAPM_RRPulseCountV_flg_Inproc/1  "VAPM_RRPulseCountV_flg"
  VAPM_RRPulseCountV_flg_Inproc/1 -> UnitConverter77/1
  UnitConverter77/1 -> VOUTP_RRPulseCountV_flg/1  "VOUTP_RRPulseCountV_flg"
  VAPM_RRPulseCountVTimeOut_flg/1 -> VAPM_RRPulseCountVTimeOut_flg_Inproc/1  "VAPM_RRPulseCountVTimeOut_flg"
  VAPM_RRPulseCountVTimeOut_flg_Inproc/1 -> UnitConverter78/1
  UnitConverter78/1 -> VOUTP_RRPulseCountVTimeOut_flg/1  "VOUTP_RRPulseCountVTimeOut_flg"
  VAPM_LFPulseCount_enum/1 -> VAPM_LFPulseCount_enum_Inproc/1  "VAPM_LFPulseCount_enum"
  VAPM_LFPulseCount_enum_Inproc/1 -> UnitConverter79/1
  UnitConverter79/1 -> VOUTP_LFPulseCount_enum/1  "VOUTP_LFPulseCount_enum"
  VAPM_LFPulseCountTimeOut_flg/1 -> VAPM_LFPulseCountTimeOut_flg_Inproc/1  "VAPM_LFPulseCountTimeOut_flg"
  VAPM_LFPulseCountTimeOut_flg_Inproc/1 -> UnitConverter80/1
  UnitConverter80/1 -> VOUTP_LFPulseCountTimeOut_flg/1  "VOUTP_LFPulseCountTimeOut_flg"
  VAPM_RFPulseCount_enum/1 -> VAPM_RFPulseCount_enum_Inproc/1  "VAPM_RFPulseCount_enum"
  VAPM_RFPulseCount_enum_Inproc/1 -> UnitConverter81/1
  UnitConverter81/1 -> VOUTP_RFPulseCount_enum/1  "VOUTP_RFPulseCount_enum"
  VAPM_RFPulseCountTimeOut_flg/1 -> VAPM_RFPulseCountTimeOut_flg_Inproc/1  "VAPM_RFPulseCountTimeOut_flg"
  VAPM_RFPulseCountTimeOut_flg_Inproc/1 -> UnitConverter82/1
  UnitConverter82/1 -> VOUTP_RFPulseCountTimeOut_flg/1  "VOUTP_RFPulseCountTimeOut_flg"
  VAPM_LRPulseCount_enum/1 -> VAPM_LRPulseCount_enum_Inproc/1  "VAPM_LRPulseCount_enum"
  VAPM_LRPulseCount_enum_Inproc/1 -> UnitConverter83/1
  UnitConverter83/1 -> VOUTP_LRPulseCount_enum/1  "VOUTP_LRPulseCount_enum"
  VAPM_LRPulseCountTimeOut_flg/1 -> VAPM_LRPulseCountTimeOut_flg_Inproc/1  "VAPM_LRPulseCountTimeOut_flg"
  VAPM_LRPulseCountTimeOut_flg_Inproc/1 -> UnitConverter84/1
  UnitConverter84/1 -> VOUTP_LRPulseCountTimeOut_flg/1  "VOUTP_LRPulseCountTimeOut_flg"
  VAPM_RRPulseCount_enum/1 -> VAPM_RRPulseCount_enum_Inproc/1  "VAPM_RRPulseCount_enum"
  VAPM_RRPulseCount_enum_Inproc/1 -> UnitConverter85/1
  UnitConverter85/1 -> VOUTP_RRPulseCount_enum/1  "VOUTP_RRPulseCount_enum"
  VAPM_RRPulseCountTimeOut_flg/1 -> VAPM_RRPulseCountTimeOut_flg_Inproc/1  "VAPM_RRPulseCountTimeOut_flg"
  VAPM_RRPulseCountTimeOut_flg_Inproc/1 -> UnitConverter86/1
  UnitConverter86/1 -> VOUTP_RRPulseCountTimeOut_flg/1  "VOUTP_RRPulseCountTimeOut_flg"
  VAPM_ShifterHandleCmd_enum/1 -> VAPM_ShifterHandleCmd_enum_Inproc/1  "VAPM_ShifterHandleCmd_enum"
  VAPM_ShifterHandleCmd_enum_Inproc/1 -> UnitConverter87/1
  UnitConverter87/1 -> VOUTP_ShifterHandleCmd_enum/1  "VOUTP_ShifterHandleCmd_enum"
  VAPM_ShifterHandleCmdTimeOut_flg/1 -> VAPM_ShifterHandleCmdTimeOut_flg_Inproc/1  "VAPM_ShifterHandleCmdTimeOut_flg"
  VAPM_ShifterHandleCmdTimeOut_flg_Inproc/1 -> UnitConverter88/1
  UnitConverter88/1 -> VOUTP_ShifterHandleCmdTimeOut_flg/1  "VOUTP_ShifterHandleCmdTimeOut_flg"
  VAPM_DriIntend_enum/1 -> VAPM_DriIntend_enum_Inproc/1  "VAPM_DriIntend_enum"
  VAPM_DriIntend_enum_Inproc/1 -> UnitConverter89/1
  UnitConverter89/1 -> VOUTP_DriIntend_enum/1  "VOUTP_DriIntend_enum"
  VAPM_DriIntendTimeOut_flg/1 -> VAPM_DriIntendTimeOut_flg_Inproc/1  "VAPM_DriIntendTimeOut_flg"
  VAPM_DriIntendTimeOut_flg_Inproc/1 -> UnitConverter90/1
  UnitConverter90/1 -> VOUTP_DriIntendTimeOut_flg/1  "VOUTP_DriIntendTimeOut_flg"
  VAPM_EPSAOIControl_enum/1 -> VAPM_EPSAOIControl_enum_Inproc/1  "VAPM_EPSAOIControl_enum"
  VAPM_EPSAOIControl_enum_Inproc/1 -> UnitConverter91/1
  UnitConverter91/1 -> VOUTP_EPSAOIControl_enum/1  "VOUTP_EPSAOIControl_enum"
  VAPM_EPSAOIControlTimeOut_flg/1 -> VAPM_EPSAOIControlTimeOut_flg_Inproc/1  "VAPM_EPSAOIControlTimeOut_flg"
  VAPM_EPSAOIControlTimeOut_flg_Inproc/1 -> UnitConverter92/1
  UnitConverter92/1 -> VOUTP_EPSAOIControlTimeOut_flg/1  "VOUTP_EPSAOIControlTimeOut_flg"
  VAPM_SASAngle_Deg/1 -> VAPM_SASAngle_Deg_Inproc/1  "VAPM_SASAngle_Deg"
  VAPM_SASAngle_Deg_Inproc/1 -> UnitConverter93/1
  UnitConverter93/1 -> VOUTP_SASAngle_Deg/1  "VOUTP_SASAngle_Deg"
  VAPM_SASAngleTimeOut_flg/1 -> VAPM_SASAngleTimeOut_flg_Inproc/1  "VAPM_SASAngleTimeOut_flg"
  VAPM_SASAngleTimeOut_flg_Inproc/1 -> UnitConverter94/1
  UnitConverter94/1 -> VOUTP_SASAngleTimeOut_flg/1  "VOUTP_SASAngleTimeOut_flg"
  VAPM_SASSpeed_degps/1 -> VAPM_SASSpeed_degps_Inproc/1  "VAPM_SASSpeed_degps"
  VAPM_SASSpeed_degps_Inproc/1 -> UnitConverter95/1
  UnitConverter95/1 -> VOUTP_SASSpeed_degps/1  "VOUTP_SASSpeed_degps"
  VAPM_SASSpeedTimeOut_flg/1 -> VAPM_SASSpeedTimeOut_flg_Inproc/1  "VAPM_SASSpeedTimeOut_flg"
  VAPM_SASSpeedTimeOut_flg_Inproc/1 -> UnitConverter96/1
  UnitConverter96/1 -> VOUTP_SASSpeedTimeOut_flg/1  "VOUTP_SASSpeedTimeOut_flg"
  VAPM_SASSpeedValid_flg/1 -> VAPM_SASSpeedValid_flg_Inproc/1  "VAPM_SASSpeedValid_flg"
  VAPM_SASSpeedValid_flg_Inproc/1 -> UnitConverter97/1
  UnitConverter97/1 -> VOUTP_SASSpeedValid_flg/1  "VOUTP_SASSpeedValid_flg"
  VAPM_SASSpeedValidTimeOut_flg/1 -> VAPM_SASSpeedValidTimeOut_flg_Inproc/1  "VAPM_SASSpeedValidTimeOut_flg"
  VAPM_SASSpeedValidTimeOut_flg_Inproc/1 -> UnitConverter98/1
  UnitConverter98/1 -> VOUTP_SASSpeedValidTimeOut_flg/1  "VOUTP_SASSpeedValidTimeOut_flg"
  VAPM_SASCAL_flg/1 -> VAPM_SASCAL_flg_Inproc/1  "VAPM_SASCAL_flg"
  VAPM_SASCAL_flg_Inproc/1 -> UnitConverter99/1
  UnitConverter99/1 -> VOUTP_SASCAL_flg/1  "VOUTP_SASCAL_flg"
  VAPM_SASCALTimeOut_flg/1 -> VAPM_SASCALTimeOut_flg_Inproc/1  "VAPM_SASCALTimeOut_flg"
  VAPM_SASCALTimeOut_flg_Inproc/1 -> UnitConverter100/1
  UnitConverter100/1 -> VOUTP_SASCALTimeOut_flg/1  "VOUTP_SASCALTimeOut_flg"
  VAPM_SASV_flg/1 -> VAPM_SASV_flg_Inproc/1  "VAPM_SASV_flg"
  VAPM_SASV_flg_Inproc/1 -> UnitConverter101/1
  UnitConverter101/1 -> VOUTP_SASV_flg/1  "VOUTP_SASV_flg"
  VAPM_SASVTimeOut_flg/1 -> VAPM_SASVTimeOut_flg_Inproc/1  "VAPM_SASVTimeOut_flg"
  VAPM_SASVTimeOut_flg_Inproc/1 -> UnitConverter102/1
  UnitConverter102/1 -> VOUTP_SASVTimeOut_flg/1  "VOUTP_SASVTimeOut_flg"
  VAPM_GRADE_Deg/1 -> VAPM_GRADE_Deg_Inproc/1  "VAPM_GRADE_Deg"
  VAPM_GRADE_Deg_Inproc/1 -> UnitConverter103/1
  UnitConverter103/1 -> VOUTP_GRADE_Deg/1  "VOUTP_GRADE_Deg"
  VAPM_GRADETimeOut_flg/1 -> VAPM_GRADETimeOut_flg_Inproc/1  "VAPM_GRADETimeOut_flg"
  VAPM_GRADETimeOut_flg_Inproc/1 -> UnitConverter104/1
  UnitConverter104/1 -> VOUTP_GRADETimeOut_flg/1  "VOUTP_GRADETimeOut_flg"
  VAPM_YawRate_degps/1 -> VAPM_YawRate_degps_Inproc/1  "VAPM_YawRate_degps"
  VAPM_YawRate_degps_Inproc/1 -> UnitConverter105/1
  UnitConverter105/1 -> VOUTP_YawRate_degps/1  "VOUTP_YawRate_degps"
  VAPM_YawRateTimeOut_flg/1 -> VAPM_YawRateTimeOut_flg_Inproc/1  "VAPM_YawRateTimeOut_flg"
  VAPM_YawRateTimeOut_flg_Inproc/1 -> UnitConverter106/1
  UnitConverter106/1 -> VOUTP_YawRateTimeOut_flg/1  "VOUTP_YawRateTimeOut_flg"
  VAPM_LatAccel_Gps/1 -> VAPM_LatAccel_Gps_Inproc/1  "VAPM_LatAccel_Gps"
  VAPM_LatAccel_Gps_Inproc/1 -> UnitConverter107/1
  UnitConverter107/1 -> VOUTP_LatAccel_Gps/1  "VOUTP_LatAccel_Gps"
  VAPM_LatAccelTimeOut_flg/1 -> VAPM_LatAccelTimeOut_flg_Inproc/1  "VAPM_LatAccelTimeOut_flg"
  VAPM_LatAccelTimeOut_flg_Inproc/1 -> UnitConverter108/1
  UnitConverter108/1 -> VOUTP_LatAccelTimeOut_flg/1  "VOUTP_LatAccelTimeOut_flg"
  VAPM_LongAccel_Gps/1 -> VAPM_LongAccel_Gps_Inproc/1  "VAPM_LongAccel_Gps"
  VAPM_LongAccel_Gps_Inproc/1 -> UnitConverter109/1
  UnitConverter109/1 -> VOUTP_LongAccel_Gps/1  "VOUTP_LongAccel_Gps"
  VAPM_LongAccelTimeOut_flg/1 -> VAPM_LongAccelTimeOut_flg_Inproc/1  "VAPM_LongAccelTimeOut_flg"
  VAPM_LongAccelTimeOut_flg_Inproc/1 -> UnitConverter110/1
  UnitConverter110/1 -> VOUTP_LongAccelTimeOut_flg/1  "VOUTP_LongAccelTimeOut_flg"
  VAPM_MCPressure_bar/1 -> VAPM_MCPressure_bar_Inproc/1  "VAPM_MCPressure_bar"
  VAPM_MCPressure_bar_Inproc/1 -> UnitConverter111/1
  UnitConverter111/1 -> VOUTP_MCPressure_bar/1  "VOUTP_MCPressure_bar"
  VAPM_MCPressureTimeOut_flg/1 -> VAPM_MCPressureTimeOut_flg_Inproc/1  "VAPM_MCPressureTimeOut_flg"
  VAPM_MCPressureTimeOut_flg_Inproc/1 -> UnitConverter112/1
  UnitConverter112/1 -> VOUTP_MCPressureTimeOut_flg/1  "VOUTP_MCPressureTimeOut_flg"
  VAPM_YawRateV_flg/1 -> VAPM_YawRateV_flg_Inproc/1  "VAPM_YawRateV_flg"
  VAPM_YawRateV_flg_Inproc/1 -> UnitConverter113/1
  UnitConverter113/1 -> VOUTP_YawRateV_flg/1  "VOUTP_YawRateV_flg"
  VAPM_YawRateVTimeOut_flg/1 -> VAPM_YawRateVTimeOut_flg_Inproc/1  "VAPM_YawRateVTimeOut_flg"
  VAPM_YawRateVTimeOut_flg_Inproc/1 -> UnitConverter114/1
  UnitConverter114/1 -> VOUTP_YawRateVTimeOut_flg/1  "VOUTP_YawRateVTimeOut_flg"
  VAPM_LatAccelV_flg/1 -> VAPM_LatAccelV_flg_Inproc/1  "VAPM_LatAccelV_flg"
  VAPM_LatAccelV_flg_Inproc/1 -> UnitConverter115/1
  UnitConverter115/1 -> VOUTP_LatAccelV_flg/1  "VOUTP_LatAccelV_flg"
  VAPM_LatAccelVTimeOut_flg/1 -> VAPM_LatAccelVTimeOut_flg_Inproc/1  "VAPM_LatAccelVTimeOut_flg"
  VAPM_LatAccelVTimeOut_flg_Inproc/1 -> UnitConverter116/1
  UnitConverter116/1 -> VOUTP_LatAccelVTimeOut_flg/1  "VOUTP_LatAccelVTimeOut_flg"
  VAPM_LongAccelV_flg/1 -> VAPM_LongAccelV_flg_Inproc/1  "VAPM_LongAccelV_flg"
  VAPM_LongAccelV_flg_Inproc/1 -> UnitConverter117/1
  UnitConverter117/1 -> VOUTP_LongAccelV_flg/1  "VOUTP_LongAccelV_flg"
  VAPM_LongAccelVTimeOut_flg/1 -> VAPM_LongAccelVTimeOut_flg_Inproc/1  "VAPM_LongAccelVTimeOut_flg"
  VAPM_LongAccelVTimeOut_flg_Inproc/1 -> UnitConverter118/1
  UnitConverter118/1 -> VOUTP_LongAccelVTimeOut_flg/1  "VOUTP_LongAccelVTimeOut_flg"
  VAPM_MCPressureV_bar/1 -> VAPM_MCPressureV_bar_Inproc/1  "VAPM_MCPressureV_bar"
  VAPM_MCPressureV_bar_Inproc/1 -> UnitConverter119/1
  UnitConverter119/1 -> VOUTP_MCPressureV_bar/1  "VOUTP_MCPressureV_bar"
  VAPM_MCPressureVTimeOut_flg/1 -> VAPM_MCPressureVTimeOut_flg_Inproc/1  "VAPM_MCPressureVTimeOut_flg"
  VAPM_MCPressureVTimeOut_flg_Inproc/1 -> UnitConverter120/1
  UnitConverter120/1 -> VOUTP_MCPressureVTimeOut_flg/1  "VOUTP_MCPressureVTimeOut_flg"
  VAPM_BrkSwSta_flg/1 -> VAPM_BrkSwSta_flg_Inproc/1  "VAPM_BrkSwSta_flg"
  VAPM_BrkSwSta_flg_Inproc/1 -> UnitConverter121/1
  UnitConverter121/1 -> VOUTP_BrkSwSta_flg/1  "VOUTP_BrkSwSta_flg"
  VAPM_BrkSwStaTimeOut_flg/1 -> VAPM_BrkSwStaTimeOut_flg_Inproc/1  "VAPM_BrkSwStaTimeOut_flg"
  VAPM_BrkSwStaTimeOut_flg_Inproc/1 -> UnitConverter122/1
  UnitConverter122/1 -> VOUTP_BrkSwStaTimeOut_flg/1  "VOUTP_BrkSwStaTimeOut_flg"
  VAPM_BrkSwV_flg/1 -> VAPM_BrkSwV_flg_Inproc/1  "VAPM_BrkSwV_flg"
  VAPM_BrkSwV_flg_Inproc/1 -> UnitConverter123/1
  UnitConverter123/1 -> VOUTP_BrkSwV_flg/1  "VOUTP_BrkSwV_flg"
  VAPM_BrkSwVTimeOut_flg/1 -> VAPM_BrkSwVTimeOut_flg_Inproc/1  "VAPM_BrkSwVTimeOut_flg"
  VAPM_BrkSwVTimeOut_flg_Inproc/1 -> UnitConverter124/1
  UnitConverter124/1 -> VOUTP_BrkSwVTimeOut_flg/1  "VOUTP_BrkSwVTimeOut_flg"
  VAPM_ESCStandstill_flg/1 -> VAPM_ESCStandstill_flg_Inproc/1  "VAPM_ESCStandstill_flg"
  VAPM_ESCStandstill_flg_Inproc/1 -> UnitConverter125/1
  UnitConverter125/1 -> VOUTP_ESCStandstill_flg/1  "VOUTP_ESCStandstill_flg"
  VAPM_ESCStandstillTimeOut_flg/1 -> VAPM_ESCStandstillTimeOut_flg_Inproc/1  "VAPM_ESCStandstillTimeOut_flg"
  VAPM_ESCStandstillTimeOut_flg_Inproc/1 -> UnitConverter126/1
  UnitConverter126/1 -> VOUTP_ESCStandstillTimeOut_flg/1  "VOUTP_ESCStandstillTimeOut_flg"
  VAPM_ESCAPSSta_enum/1 -> VAPM_ESCAPSSta_enum_Inproc/1  "VAPM_ESCAPSSta_enum"
  VAPM_ESCAPSSta_enum_Inproc/1 -> UnitConverter127/1
  UnitConverter127/1 -> VOUTP_ESCAPSSta_enum/1  "VOUTP_ESCAPSSta_enum"
  VAPM_ESCAPSStaTimeOut_flg/1 -> VAPM_ESCAPSStaTimeOut_flg_Inproc/1  "VAPM_ESCAPSStaTimeOut_flg"
  VAPM_ESCAPSStaTimeOut_flg_Inproc/1 -> UnitConverter128/1
  UnitConverter128/1 -> VOUTP_ESCAPSStaTimeOut_flg/1  "VOUTP_ESCAPSStaTimeOut_flg"
  VAPM_EPBExtReleaseAvail_flg/1 -> VAPM_EPBExtReleaseAvail_flg_Inproc/1  "VAPM_EPBExtReleaseAvail_flg"
  VAPM_EPBExtReleaseAvail_flg_Inproc/1 -> UnitConverter129/1
  UnitConverter129/1 -> VOUTP_EPBExtReleaseAvail_flg/1  "VOUTP_EPBExtReleaseAvail_flg"
  VAPM_EPBExtReleaseAvailTimeOut_flg/1 -> VAPM_EPBExtReleaseAvailTimeOut_flg_Inproc/1  "VAPM_EPBExtReleaseAvailTimeOut_flg"
  VAPM_EPBExtReleaseAvailTimeOut_flg_Inproc/1 -> UnitConverter130/1
  UnitConverter130/1 -> VOUTP_EPBExtReleaseAvailTimeOut_flg/1  "VOUTP_EPBExtReleaseAvailTimeOut_flg"
  VAPM_EPBExtApplyAvail_flg/1 -> VAPM_EPBExtApplyAvail_flg_Inproc/1  "VAPM_EPBExtApplyAvail_flg"
  VAPM_EPBExtApplyAvail_flg_Inproc/1 -> UnitConverter131/1
  UnitConverter131/1 -> VOUTP_EPBExtApplyAvail_flg/1  "VOUTP_EPBExtApplyAvail_flg"
  VAPM_EPBExtApplyAvailTimeOut_flg/1 -> VAPM_EPBExtApplyAvailTimeOut_flg_Inproc/1  "VAPM_EPBExtApplyAvailTimeOut_flg"
  VAPM_EPBExtApplyAvailTimeOut_flg_Inproc/1 -> UnitConverter132/1
  UnitConverter132/1 -> VOUTP_EPBExtApplyAvailTimeOut_flg/1  "VOUTP_EPBExtApplyAvailTimeOut_flg"
  VAPM_EPBErrSta_enum/1 -> VAPM_EPBErrSta_enum_Inproc/1  "VAPM_EPBErrSta_enum"
  VAPM_EPBErrSta_enum_Inproc/1 -> UnitConverter133/1
  UnitConverter133/1 -> VOUTP_EPBErrSta_enum/1  "VOUTP_EPBErrSta_enum"
  VAPM_EPBErrStaTimeOut_flg/1 -> VAPM_EPBErrStaTimeOut_flg_Inproc/1  "VAPM_EPBErrStaTimeOut_flg"
  VAPM_EPBErrStaTimeOut_flg_Inproc/1 -> UnitConverter134/1
  UnitConverter134/1 -> VOUTP_EPBErrStaTimeOut_flg/1  "VOUTP_EPBErrStaTimeOut_flg"
  VAPM_EPBSta_enum/1 -> VAPM_EPBSta_enum_Inproc/1  "VAPM_EPBSta_enum"
  VAPM_EPBSta_enum_Inproc/1 -> UnitConverter135/1
  UnitConverter135/1 -> VOUTP_EPBSta_enum/1  "VOUTP_EPBSta_enum"
  VAPM_EPBStaTimeOut_flg/1 -> VAPM_EPBStaTimeOut_flg_Inproc/1  "VAPM_EPBStaTimeOut_flg"
  VAPM_EPBStaTimeOut_flg_Inproc/1 -> UnitConverter136/1
  UnitConverter136/1 -> VOUTP_EPBStaTimeOut_flg/1  "VOUTP_EPBStaTimeOut_flg"
  VAPM_AVMparkingcancel_enum/1 -> VAPM_AVMparkingcancel_enum_Inproc/1  "VAPM_AVMparkingcancel_enum"
  VAPM_AVMparkingcancel_enum_Inproc/1 -> UnitConverter137/1
  UnitConverter137/1 -> VOUTP_AVMparkingcancel_enum/1  "VOUTP_AVMparkingcancel_enum"
  VAPM_AVMparkingcancelTimeOut_flg/1 -> VAPM_AVMparkingcancelTimeOut_flg_Inproc/1  "VAPM_AVMparkingcancelTimeOut_flg"
  VAPM_AVMparkingcancelTimeOut_flg_Inproc/1 -> UnitConverter138/1
  UnitConverter138/1 -> VOUTP_AVMparkingcancelTimeOut_flg/1  "VOUTP_AVMparkingcancelTimeOut_flg"
  VAPM_AVMparkingexcute_enum/1 -> VAPM_AVMparkingexcute_enum_Inproc/1  "VAPM_AVMparkingexcute_enum"
  VAPM_AVMparkingexcute_enum_Inproc/1 -> UnitConverter139/1
  UnitConverter139/1 -> VOUTP_AVMparkingexcute_enum/1  "VOUTP_AVMparkingexcute_enum"
  VAPM_AVMparkingexcuteTimeOut_flg/1 -> VAPM_AVMparkingexcuteTimeOut_flg_Inproc/1  "VAPM_AVMparkingexcuteTimeOut_flg"
  VAPM_AVMparkingexcuteTimeOut_flg_Inproc/1 -> UnitConverter140/1
  UnitConverter140/1 -> VOUTP_AVMparkingexcuteTimeOut_flg/1  "VOUTP_AVMparkingexcuteTimeOut_flg"
  VAPM_AVMParkingmode_enum/1 -> VAPM_AVMParkingmode_enum_Inproc/1  "VAPM_AVMParkingmode_enum"
  VAPM_AVMParkingmode_enum_Inproc/1 -> UnitConverter141/1
  UnitConverter141/1 -> VOUTP_AVMParkingmode_enum/1  "VOUTP_AVMParkingmode_enum"
  VAPM_AVMParkingmodeTimeOut_flg/1 -> VAPM_AVMParkingmodeTimeOut_flg_Inproc/1  "VAPM_AVMParkingmodeTimeOut_flg"
  VAPM_AVMParkingmodeTimeOut_flg_Inproc/1 -> UnitConverter142/1
  UnitConverter142/1 -> VOUTP_AVMParkingmodeTimeOut_flg/1  "VOUTP_AVMParkingmodeTimeOut_flg"
  VAPM_AVMErrSTA_flg/1 -> VAPM_AVMErrSTA_flg_Inproc/1  "VAPM_AVMErrSTA_flg"
  VAPM_AVMErrSTA_flg_Inproc/1 -> UnitConverter143/1
  UnitConverter143/1 -> VOUTP_AVMErrSTA_flg/1  "VOUTP_AVMErrSTA_flg"
  VAPM_AVMErrSTATimeOut_flg/1 -> VAPM_AVMErrSTATimeOut_flg_Inproc/1  "VAPM_AVMErrSTATimeOut_flg"
  VAPM_AVMErrSTATimeOut_flg_Inproc/1 -> UnitConverter144/1
  UnitConverter144/1 -> VOUTP_AVMErrSTATimeOut_flg/1  "VOUTP_AVMErrSTATimeOut_flg"
  VAPM_IVIStatus_flg/1 -> VAPM_IVIStatus_flg_Inproc/1  "VAPM_IVIStatus_flg"
  VAPM_IVIStatus_flg_Inproc/1 -> UnitConverter145/1
  UnitConverter145/1 -> VOUTP_IVIStatus_flg/1  "VOUTP_IVIStatus_flg"
  VAPM_IVIStatusTimeOut_flg/1 -> VAPM_IVIStatusTimeOut_flg_Inproc/1  "VAPM_IVIStatusTimeOut_flg"
  VAPM_IVIStatusTimeOut_flg_Inproc/1 -> UnitConverter146/1
  UnitConverter146/1 -> VOUTP_IVIStatusTimeOut_flg/1  "VOUTP_IVIStatusTimeOut_flg"
  VAPM_CAASSw_enum/1 -> VAPM_CAASSw_enum_Inproc/1  "VAPM_CAASSw_enum"
  VAPM_CAASSw_enum_Inproc/1 -> UnitConverter147/1
  UnitConverter147/1 -> VOUTP_CAASSw_enum/1  "VOUTP_CAASSw_enum"
  VAPM_CAASSwTimeOut_flg/1 -> VAPM_CAASSwTimeOut_flg_Inproc/1  "VAPM_CAASSwTimeOut_flg"
  VAPM_CAASSwTimeOut_flg_Inproc/1 -> UnitConverter148/1
  UnitConverter148/1 -> VOUTP_CAASSwTimeOut_flg/1  "VOUTP_CAASSwTimeOut_flg"
  VAPM_IVIScreen_enum/1 -> VAPM_IVIScreen_enum_Inproc/1  "VAPM_IVIScreen_enum"
  VAPM_IVIScreen_enum_Inproc/1 -> UnitConverter149/1
  UnitConverter149/1 -> VOUTP_IVIScreen_enum/1  "VOUTP_IVIScreen_enum"
  VAPM_IVIScreenTimeOut_flg/1 -> VAPM_IVIScreenTimeOut_flg_Inproc/1  "VAPM_IVIScreenTimeOut_flg"
  VAPM_IVIScreenTimeOut_flg_Inproc/1 -> UnitConverter150/1
  UnitConverter150/1 -> VOUTP_IVIScreenTimeOut_flg/1  "VOUTP_IVIScreenTimeOut_flg"
  VAPM_ABSActive_flg/1 -> VAPM_ABSActive_flg_Inproc/1  "VAPM_ABSActive_flg"
  VAPM_ABSActive_flg_Inproc/1 -> UnitConverter151/1
  UnitConverter151/1 -> VOUTP_ABSActive_flg/1  "VOUTP_ABSActive_flg"
  VAPM_ABSActiveTimeOut_flg/1 -> VAPM_ABSActiveTimeOut_flg_Inproc/1  "VAPM_ABSActiveTimeOut_flg"
  VAPM_ABSActiveTimeOut_flg_Inproc/1 -> UnitConverter152/1
  UnitConverter152/1 -> VOUTP_ABSActiveTimeOut_flg/1  "VOUTP_ABSActiveTimeOut_flg"
  VAPM_TCSActive_flg/1 -> VAPM_TCSActive_flg_Inproc/1  "VAPM_TCSActive_flg"
  VAPM_TCSActive_flg_Inproc/1 -> UnitConverter153/1
  UnitConverter153/1 -> VOUTP_TCSActive_flg/1  "VOUTP_TCSActive_flg"
  VAPM_TCSActiveTimeOut_flg/1 -> VAPM_TCSActiveTimeOut_flg_Inproc/1  "VAPM_TCSActiveTimeOut_flg"
  VAPM_TCSActiveTimeOut_flg_Inproc/1 -> UnitConverter154/1
  UnitConverter154/1 -> VOUTP_TCSActiveTimeOut_flg/1  "VOUTP_TCSActiveTimeOut_flg"
  VAPM_DriverSeatBeltCmd_flg/1 -> VAPM_DriverSeatBeltCmd_flg_Inproc/1  "VAPM_DriverSeatBeltCmd_flg"
  VAPM_DriverSeatBeltCmd_flg_Inproc/1 -> UnitConverter155/1
  UnitConverter155/1 -> VOUTP_DriverSeatBeltCmd_flg/1  "VOUTP_DriverSeatBeltCmd_flg"
  VAPM_DriverSeatBeltCmdTimeOut_flg/1 -> VAPM_DriverSeatBeltCmdTimeOut_flg_Inproc/1  "VAPM_DriverSeatBeltCmdTimeOut_flg"
  VAPM_DriverSeatBeltCmdTimeOut_flg_Inproc/1 -> UnitConverter156/1
  UnitConverter156/1 -> VOUTP_DriverSeatBeltCmdTimeOut_flg/1  "VOUTP_DriverSeatBeltCmdTimeOut_flg"
  VAPM_APSProgressPCT_pct/1 -> VAPM_APSProgressPCT_pct_Inproc/1  "VAPM_APSProgressPCT_pct"
  VAPM_APSProgressPCT_pct_Inproc/1 -> UnitConverter157/1
  UnitConverter157/1 -> VOUTP_APSProgressPCT_pct/1  "VOUTP_APSProgressPCT_pct"
  VAPM_APSRQDisplay_enum/1 -> VAPM_APSRQDisplay_enum_Inproc/1  "VAPM_APSRQDisplay_enum"
  VAPM_APSRQDisplay_enum_Inproc/1 -> UnitConverter158/1
  UnitConverter158/1 -> VOUTP_APSRQDisplay_enum/1  "VOUTP_APSRQDisplay_enum"
  VAPM_APSSWVer_enum/1 -> VAPM_APSSWVer_enum_Inproc/1  "VAPM_APSSWVer_enum"
  VAPM_APSSWVer_enum_Inproc/1 -> UnitConverter159/1
  UnitConverter159/1 -> VOUTP_APSSWVer_enum/1  "VOUTP_APSSWVer_enum"
  VAPM_APSHWVer_enum/1 -> VAPM_APSHWVer_enum_Inproc/1  "VAPM_APSHWVer_enum"
  VAPM_APSHWVer_enum_Inproc/1 -> UnitConverter160/1
  UnitConverter160/1 -> VOUTP_APSHWVer_enum/1  "VOUTP_APSHWVer_enum"
  VAPM_APSExitCondition_enum/1 -> VAPM_APSExitCondition_enum_Inproc/1  "VAPM_APSExitCondition_enum"
  VAPM_APSExitCondition_enum_Inproc/1 -> UnitConverter161/1
  UnitConverter161/1 -> VOUTP_APSExitCondition_enum/1  "VOUTP_APSExitCondition_enum"
  VAPM_APSAngleTarget_Deg/1 -> VAPM_APSAngleTarget_Deg_Inproc/1  "VAPM_APSAngleTarget_Deg"
  VAPM_APSAngleTarget_Deg_Inproc/1 -> UnitConverter162/1
  UnitConverter162/1 -> VOUTP_APSAngleTarget_Deg/1  "VOUTP_APSAngleTarget_Deg"
  VAPM_APSVRqEPASCtrl_flg/1 -> VAPM_APSVRqEPASCtrl_flg_Inproc/1  "VAPM_APSVRqEPASCtrl_flg"
  VAPM_APSVRqEPASCtrl_flg_Inproc/1 -> UnitConverter163/1
  UnitConverter163/1 -> VOUTP_APSVRqEPASCtrl_flg/1  "VOUTP_APSVRqEPASCtrl_flg"
  VAPM_APSRqEPASCtrl_flg/1 -> VAPM_APSRqEPASCtrl_flg_Inproc/1  "VAPM_APSRqEPASCtrl_flg"
  VAPM_APSRqEPASCtrl_flg_Inproc/1 -> UnitConverter164/1
  UnitConverter164/1 -> VOUTP_APSRqEPASCtrl_flg/1  "VOUTP_APSRqEPASCtrl_flg"
  VAPM_CAASSta_enum/1 -> VAPM_CAASSta_enum_Inproc/1  "VAPM_CAASSta_enum"
  VAPM_CAASSta_enum_Inproc/1 -> UnitConverter165/1
  UnitConverter165/1 -> VOUTP_CAASSta_enum/1  "VOUTP_CAASSta_enum"
  VBCM_AntitheftSta_enum/1 -> VBCM_AntitheftSta_enum_Inproc/1  "VBCM_AntitheftSta_enum"
  VBCM_AntitheftSta_enum_Inproc/1 -> UnitConverter166/1
  UnitConverter166/1 -> VOUTP_AntitheftSta_enum/1  "VOUTP_AntitheftSta_enum"
  VBCM_TailgateRemote_enum/1 -> VBCM_TailgateRemote_enum_Inproc/1  "VBCM_TailgateRemote_enum"
  VBCM_TailgateRemote_enum_Inproc/1 -> UnitConverter167/1
  UnitConverter167/1 -> VOUTP_TailgateRemote_enum/1  "VOUTP_TailgateRemote_enum"
  VBCM_HornCtrl_flg/1 -> VBCM_HornCtrl_flg_Inproc/1  "VBCM_HornCtrl_flg"
  VBCM_HornCtrl_flg_Inproc/1 -> UnitConverter168/1
  UnitConverter168/1 -> VOUTP_HornCtrl_flg/1  "VOUTP_HornCtrl_flg"
  VBCM_AllDoorSW_flg/1 -> VBCM_AllDoorSW_flg_Inproc/1  "VBCM_AllDoorSW_flg"
  VBCM_AllDoorSW_flg_Inproc/1 -> UnitConverter169/1
  UnitConverter169/1 -> VOUTP_AllDoorSW_flg/1  "VOUTP_AllDoorSW_flg"
  VBCM_BCMDoorLockSta_flg/1 -> VBCM_BCMDoorLockSta_flg_Inproc/1  "VBCM_BCMDoorLockSta_flg"
  VBCM_BCMDoorLockSta_flg_Inproc/1 -> UnitConverter170/1
  UnitConverter170/1 -> VOUTP_BCMDoorLockSta_flg/1  "VOUTP_BCMDoorLockSta_flg"
  VBCM_AntitheftSeatFlod_flg/1 -> VBCM_AntitheftSeatFlod_flg_Inproc/1  "VBCM_AntitheftSeatFlod_flg"
  VBCM_AntitheftSeatFlod_flg_Inproc/1 -> UnitConverter171/1
  UnitConverter171/1 -> VOUTP_AntitheftSeatFlod_flg/1  "VOUTP_AntitheftSeatFlod_flg"
  VBCM_HoodSW_flg/1 -> VBCM_HoodSW_flg_Inproc/1  "VBCM_HoodSW_flg"
  VBCM_HoodSW_flg_Inproc/1 -> UnitConverter172/1
  UnitConverter172/1 -> VOUTP_HoodSW_flg/1  "VOUTP_HoodSW_flg"
  VBCM_TailgateSW_flg/1 -> VBCM_TailgateSW_flg_Inproc/1  "VBCM_TailgateSW_flg"
  VBCM_TailgateSW_flg_Inproc/1 -> UnitConverter173/1
  UnitConverter173/1 -> VOUTP_TailgateSW_flg/1  "VOUTP_TailgateSW_flg"
  VBCM_DrDoorSW_flg/1 -> VBCM_DrDoorSW_flg_Inproc/1  "VBCM_DrDoorSW_flg"
  VBCM_DrDoorSW_flg_Inproc/1 -> UnitConverter174/1
  UnitConverter174/1 -> VOUTP_DrDoorSW_flg/1  "VOUTP_DrDoorSW_flg"
  VBCM_PsDoorSW_flg/1 -> VBCM_PsDoorSW_flg_Inproc/1  "VBCM_PsDoorSW_flg"
  VBCM_PsDoorSW_flg_Inproc/1 -> UnitConverter175/1
  UnitConverter175/1 -> VOUTP_PsDoorSW_flg/1  "VOUTP_PsDoorSW_flg"
  VBCM_RLDoorSW_flg/1 -> VBCM_RLDoorSW_flg_Inproc/1  "VBCM_RLDoorSW_flg"
  VBCM_RLDoorSW_flg_Inproc/1 -> UnitConverter176/1
  UnitConverter176/1 -> VOUTP_RLDoorSW_flg/1  "VOUTP_RLDoorSW_flg"
  VBCM_RRDoorSW_flg/1 -> VBCM_RRDoorSW_flg_Inproc/1  "VBCM_RRDoorSW_flg"
  VBCM_RRDoorSW_flg_Inproc/1 -> UnitConverter177/1
  UnitConverter177/1 -> VOUTP_RRDoorSW_flg/1  "VOUTP_RRDoorSW_flg"
  VBCM_LockSetting_flg/1 -> VBCM_LockSetting_flg_Inproc/1  "VBCM_LockSetting_flg"
  VBCM_LockSetting_flg_Inproc/1 -> UnitConverter178/1
  UnitConverter178/1 -> VOUTP_LockSetting_flg/1  "VOUTP_LockSetting_flg"
  VBCM_FrChargingDoorCtrl_enum/1 -> VBCM_FrChargingDoorCtrl_enum_Inproc/1  "VBCM_FrChargingDoorCtrl_enum"
  VBCM_FrChargingDoorCtrl_enum_Inproc/1 -> UnitConverter179/1
  UnitConverter179/1 -> VOUTP_FrChargingDoorCtrl_enum/1  "VOUTP_FrChargingDoorCtrl_enum"
  VBCM_RrChargingDoorCtrl_enum/1 -> VBCM_RrChargingDoorCtrl_enum_Inproc/1  "VBCM_RrChargingDoorCtrl_enum"
  VBCM_RrChargingDoorCtrl_enum_Inproc/1 -> UnitConverter180/1
  UnitConverter180/1 -> VOUTP_RrChargingDoorCtrl_enum/1  "VOUTP_RrChargingDoorCtrl_enum"
  VBCM_CrashDetd_flg/1 -> VBCM_CrashDetd_flg_Inproc/1  "VBCM_CrashDetd_flg"
  VBCM_CrashDetd_flg_Inproc/1 -> UnitConverter181/1
  UnitConverter181/1 -> VOUTP_CrashDetd_flg/1  "VOUTP_CrashDetd_flg"
  VBCM_CTDCtrl_enum/1 -> VBCM_CTDCtrl_enum_Inproc/1  "VBCM_CTDCtrl_enum"
  VBCM_CTDCtrl_enum_Inproc/1 -> UnitConverter182/1
  UnitConverter182/1 -> VOUTP_CTDCtrl_enum/1  "VOUTP_CTDCtrl_enum"
  VBCM_DoorLockIND_flg/1 -> VBCM_DoorLockIND_flg_Inproc/1  "VBCM_DoorLockIND_flg"
  VBCM_DoorLockIND_flg_Inproc/1 -> UnitConverter183/1
  UnitConverter183/1 -> VOUTP_DoorLockIND_flg/1  "VOUTP_DoorLockIND_flg"
  VBCM_CTDLockSW_flg/1 -> VBCM_CTDLockSW_flg_Inproc/1  "VBCM_CTDLockSW_flg"
  VBCM_CTDLockSW_flg_Inproc/1 -> UnitConverter184/1
  UnitConverter184/1 -> VOUTP_CTDLockSW_flg/1  "VOUTP_CTDLockSW_flg"
  VBCM_Dimmer_pct/1 -> VBCM_Dimmer_pct_Inproc/1  "VBCM_Dimmer_pct"
  VBCM_Dimmer_pct_Inproc/1 -> UnitConverter185/1
  UnitConverter185/1 -> VOUTP_Dimmer_pct/1  "VOUTP_Dimmer_pct"
  VBCM_DimmerEN_flg/1 -> VBCM_DimmerEN_flg_Inproc/1  "VBCM_DimmerEN_flg"
  VBCM_DimmerEN_flg_Inproc/1 -> UnitConverter186/1
  UnitConverter186/1 -> VOUTP_DimmerEN_flg/1  "VOUTP_DimmerEN_flg"
  VBCM_PosLamp_flg/1 -> VBCM_PosLamp_flg_Inproc/1  "VBCM_PosLamp_flg"
  VBCM_PosLamp_flg_Inproc/1 -> UnitConverter187/1
  UnitConverter187/1 -> VOUTP_PosLamp_flg/1  "VOUTP_PosLamp_flg"
  VBCM_LBeam_flg/1 -> VBCM_LBeam_flg_Inproc/1  "VBCM_LBeam_flg"
  VBCM_LBeam_flg_Inproc/1 -> UnitConverter188/1
  UnitConverter188/1 -> VOUTP_LBeam_flg/1  "VOUTP_LBeam_flg"
  VBCM_HBeam_flg/1 -> VBCM_HBeam_flg_Inproc/1  "VBCM_HBeam_flg"
  VBCM_HBeam_flg_Inproc/1 -> UnitConverter189/1
  UnitConverter189/1 -> VOUTP_HBeam_flg/1  "VOUTP_HBeam_flg"
  VBCM_RrFogLamp_flg/1 -> VBCM_RrFogLamp_flg_Inproc/1  "VBCM_RrFogLamp_flg"
  VBCM_RrFogLamp_flg_Inproc/1 -> UnitConverter190/1
  UnitConverter190/1 -> VOUTP_RrFogLamp_flg/1  "VOUTP_RrFogLamp_flg"
  VBCM_BrakeLamp_flg/1 -> VBCM_BrakeLamp_flg_Inproc/1  "VBCM_BrakeLamp_flg"
  VBCM_BrakeLamp_flg_Inproc/1 -> UnitConverter191/1
  UnitConverter191/1 -> VOUTP_BrakeLamp_flg/1  "VOUTP_BrakeLamp_flg"
  VBCM_ReverseLamp_flg/1 -> VBCM_ReverseLamp_flg_Inproc/1  "VBCM_ReverseLamp_flg"
  VBCM_ReverseLamp_flg_Inproc/1 -> UnitConverter192/1
  UnitConverter192/1 -> VOUTP_ReverseLamp_flg/1  "VOUTP_ReverseLamp_flg"
  VBCM_LDRL_flg/1 -> VBCM_LDRL_flg_Inproc/1  "VBCM_LDRL_flg"
  VBCM_LDRL_flg_Inproc/1 -> UnitConverter193/1
  UnitConverter193/1 -> VOUTP_LDRL_flg/1  "VOUTP_LDRL_flg"
  VBCM_RDRL_flg/1 -> VBCM_RDRL_flg_Inproc/1  "VBCM_RDRL_flg"
  VBCM_RDRL_flg_Inproc/1 -> UnitConverter194/1
  UnitConverter194/1 -> VOUTP_RDRL_flg/1  "VOUTP_RDRL_flg"
  VBCM_LBSD_flg/1 -> VBCM_LBSD_flg_Inproc/1  "VBCM_LBSD_flg"
  VBCM_LBSD_flg_Inproc/1 -> UnitConverter195/1
  UnitConverter195/1 -> VOUTP_LBSD_flg/1  "VOUTP_LBSD_flg"
  VBCM_RBSD_flg/1 -> VBCM_RBSD_flg_Inproc/1  "VBCM_RBSD_flg"
  VBCM_RBSD_flg_Inproc/1 -> UnitConverter196/1
  UnitConverter196/1 -> VOUTP_RBSD_flg/1  "VOUTP_RBSD_flg"
  VBCM_HazardSW_flg/1 -> VBCM_HazardSW_flg_Inproc/1  "VBCM_HazardSW_flg"
  VBCM_HazardSW_flg_Inproc/1 -> UnitConverter197/1
  UnitConverter197/1 -> VOUTP_HazardSW_flg/1  "VOUTP_HazardSW_flg"
  VBCM_LTurnLP_flg/1 -> VBCM_LTurnLP_flg_Inproc/1  "VBCM_LTurnLP_flg"
  VBCM_LTurnLP_flg_Inproc/1 -> UnitConverter198/1
  UnitConverter198/1 -> VOUTP_LTurnLP_flg/1  "VOUTP_LTurnLP_flg"
  VBCM_RTurnLP_flg/1 -> VBCM_RTurnLP_flg_Inproc/1  "VBCM_RTurnLP_flg"
  VBCM_RTurnLP_flg_Inproc/1 -> UnitConverter199/1
  UnitConverter199/1 -> VOUTP_RTurnLP_flg/1  "VOUTP_RTurnLP_flg"
  VBCM_BCMBuzzerReq_flg/1 -> VBCM_BCMBuzzerReq_flg_Inproc/1  "VBCM_BCMBuzzerReq_flg"
  VBCM_BCMBuzzerReq_flg_Inproc/1 -> UnitConverter200/1
  UnitConverter200/1 -> VOUTP_BCMBuzzerReq_flg/1  "VOUTP_BCMBuzzerReq_flg"
  VBCM_MirrorCtrl_enum/1 -> VBCM_MirrorCtrl_enum_Inproc/1  "VBCM_MirrorCtrl_enum"
  VBCM_MirrorCtrl_enum_Inproc/1 -> UnitConverter201/1
  UnitConverter201/1 -> VOUTP_MirrorCtrl_enum/1  "VOUTP_MirrorCtrl_enum"
  VBCM_MirrorDefog_flg/1 -> VBCM_MirrorDefog_flg_Inproc/1  "VBCM_MirrorDefog_flg"
  VBCM_MirrorDefog_flg_Inproc/1 -> UnitConverter202/1
  UnitConverter202/1 -> VOUTP_MirrorDefog_flg/1  "VOUTP_MirrorDefog_flg"
  VBCM_RrDefog_flg/1 -> VBCM_RrDefog_flg_Inproc/1  "VBCM_RrDefog_flg"
  VBCM_RrDefog_flg_Inproc/1 -> UnitConverter203/1
  UnitConverter203/1 -> VOUTP_RrDefog_flg/1  "VOUTP_RrDefog_flg"
  VBCM_RoomLampH_flg/1 -> VBCM_RoomLampH_flg_Inproc/1  "VBCM_RoomLampH_flg"
  VBCM_RoomLampH_flg_Inproc/1 -> UnitConverter204/1
  UnitConverter204/1 -> VOUTP_RoomLampH_flg/1  "VOUTP_RoomLampH_flg"
  VBCM_RoomLampL_flg/1 -> VBCM_RoomLampL_flg_Inproc/1  "VBCM_RoomLampL_flg"
  VBCM_RoomLampL_flg_Inproc/1 -> UnitConverter205/1
  UnitConverter205/1 -> VOUTP_RoomLampL_flg/1  "VOUTP_RoomLampL_flg"
  VBCM_TrunkRel_flg/1 -> VBCM_TrunkRel_flg_Inproc/1  "VBCM_TrunkRel_flg"
  VBCM_TrunkRel_flg_Inproc/1 -> UnitConverter206/1
  UnitConverter206/1 -> VOUTP_TrunkRel_flg/1  "VOUTP_TrunkRel_flg"
  VBCM_TailgateHDSW_flg/1 -> VBCM_TailgateHDSW_flg_Inproc/1  "VBCM_TailgateHDSW_flg"
  VBCM_TailgateHDSW_flg_Inproc/1 -> UnitConverter207/1
  UnitConverter207/1 -> VOUTP_TailgateHDSW_flg/1  "VOUTP_TailgateHDSW_flg"
  VBCM_FrWiperL_flg/1 -> VBCM_FrWiperL_flg_Inproc/1  "VBCM_FrWiperL_flg"
  VBCM_FrWiperL_flg_Inproc/1 -> UnitConverter208/1
  UnitConverter208/1 -> VOUTP_FrWiperL_flg/1  "VOUTP_FrWiperL_flg"
  VBCM_FrWiperH_flg/1 -> VBCM_FrWiperH_flg_Inproc/1  "VBCM_FrWiperH_flg"
  VBCM_FrWiperH_flg_Inproc/1 -> UnitConverter209/1
  UnitConverter209/1 -> VOUTP_FrWiperH_flg/1  "VOUTP_FrWiperH_flg"
  VBCM_RrWiper_flg/1 -> VBCM_RrWiper_flg_Inproc/1  "VBCM_RrWiper_flg"
  VBCM_RrWiper_flg_Inproc/1 -> UnitConverter210/1
  UnitConverter210/1 -> VOUTP_RrWiper_flg/1  "VOUTP_RrWiper_flg"
  VBCM_WasherCtrl_enum/1 -> VBCM_WasherCtrl_enum_Inproc/1  "VBCM_WasherCtrl_enum"
  VBCM_WasherCtrl_enum_Inproc/1 -> UnitConverter211/1
  UnitConverter211/1 -> VOUTP_WasherCtrl_enum/1  "VOUTP_WasherCtrl_enum"
  VBCM_WiperFixMode_flg/1 -> VBCM_WiperFixMode_flg_Inproc/1  "VBCM_WiperFixMode_flg"
  VBCM_WiperFixMode_flg_Inproc/1 -> UnitConverter212/1
  UnitConverter212/1 -> VOUTP_WiperFixMode_flg/1  "VOUTP_WiperFixMode_flg"
  VBCM_User1DrAmbLightBrightness_enum/1 -> VBCM_User1DrAmbLightBrightness_enum_Inproc/1  "VBCM_User1DrAmbLightBrightness_enum"
  VBCM_User1DrAmbLightBrightness_enum_Inproc/1 -> UnitConverter213/1
  UnitConverter213/1 -> VOUTP_User1DrAmbLightBrightness_enum/1  "VOUTP_User1DrAmbLightBrightness_enum"
  VBCM_User1IPAmbLightBrightness_enum/1 -> VBCM_User1IPAmbLightBrightness_enum_Inproc/1  "VBCM_User1IPAmbLightBrightness_enum"
  VBCM_User1IPAmbLightBrightness_enum_Inproc/1 -> UnitConverter214/1
  UnitConverter214/1 -> VOUTP_User1IPAmbLightBrightness_enum/1  "VOUTP_User1IPAmbLightBrightness_enum"
  VBCM_User2DrAmbLightBrightness_enum/1 -> VBCM_User2DrAmbLightBrightness_enum_Inproc/1  "VBCM_User2DrAmbLightBrightness_enum"
  VBCM_User2DrAmbLightBrightness_enum_Inproc/1 -> UnitConverter215/1
  UnitConverter215/1 -> VOUTP_User2DrAmbLightBrightness_enum/1  "VOUTP_User2DrAmbLightBrightness_enum"
  VBCM_User2IPAmbLightBrightness_enum/1 -> VBCM_User2IPAmbLightBrightness_enum_Inproc/1  "VBCM_User2IPAmbLightBrightness_enum"
  VBCM_User2IPAmbLightBrightness_enum_Inproc/1 -> UnitConverter216/1
  UnitConverter216/1 -> VOUTP_User2IPAmbLightBrightness_enum/1  "VOUTP_User2IPAmbLightBrightness_enum"
  VBCM_User3DrAmbLightBrightness_enum/1 -> VBCM_User3DrAmbLightBrightness_enum_Inproc/1  "VBCM_User3DrAmbLightBrightness_enum"
  VBCM_User3DrAmbLightBrightness_enum_Inproc/1 -> UnitConverter217/1
  UnitConverter217/1 -> VOUTP_User3DrAmbLightBrightness_enum/1  "VOUTP_User3DrAmbLightBrightness_enum"
  VBCM_User3IPAmbLightBrightness_enum/1 -> VBCM_User3IPAmbLightBrightness_enum_Inproc/1  "VBCM_User3IPAmbLightBrightness_enum"
  VBCM_User3IPAmbLightBrightness_enum_Inproc/1 -> UnitConverter218/1
  UnitConverter218/1 -> VOUTP_User3IPAmbLightBrightness_enum/1  "VOUTP_User3IPAmbLightBrightness_enum"
  VBCM_User4DrAmbLightBrightness_enum/1 -> VBCM_User4DrAmbLightBrightness_enum_Inproc/1  "VBCM_User4DrAmbLightBrightness_enum"
  VBCM_User4DrAmbLightBrightness_enum_Inproc/1 -> UnitConverter219/1
  UnitConverter219/1 -> VOUTP_User4DrAmbLightBrightness_enum/1  "VOUTP_User4DrAmbLightBrightness_enum"
  VBCM_User4IPAmbLightBrightness_enum/1 -> VBCM_User4IPAmbLightBrightness_enum_Inproc/1  "VBCM_User4IPAmbLightBrightness_enum"
  VBCM_User4IPAmbLightBrightness_enum_Inproc/1 -> UnitConverter220/1
  UnitConverter220/1 -> VOUTP_User4IPAmbLightBrightness_enum/1  "VOUTP_User4IPAmbLightBrightness_enum"
  VBCM_User5DrAmbLightBrightness_enum/1 -> VBCM_User5DrAmbLightBrightness_enum_Inproc/1  "VBCM_User5DrAmbLightBrightness_enum"
  VBCM_User5DrAmbLightBrightness_enum_Inproc/1 -> UnitConverter221/1
  UnitConverter221/1 -> VOUTP_User5DrAmbLightBrightness_enum/1  "VOUTP_User5DrAmbLightBrightness_enum"
  VBCM_User5IPAmbLightBrightness_enum/1 -> VBCM_User5IPAmbLightBrightness_enum_Inproc/1  "VBCM_User5IPAmbLightBrightness_enum"
  VBCM_User5IPAmbLightBrightness_enum_Inproc/1 -> UnitConverter222/1
  UnitConverter222/1 -> VOUTP_User5IPAmbLightBrightness_enum/1  "VOUTP_User5IPAmbLightBrightness_enum"
  VBCM_User6DrAmbLightBrightness_enum/1 -> VBCM_User6DrAmbLightBrightness_enum_Inproc/1  "VBCM_User6DrAmbLightBrightness_enum"
  VBCM_User6DrAmbLightBrightness_enum_Inproc/1 -> UnitConverter223/1
  UnitConverter223/1 -> VOUTP_User6DrAmbLightBrightness_enum/1  "VOUTP_User6DrAmbLightBrightness_enum"
  VBCM_User6IPAmbLightBrightness_enum/1 -> VBCM_User6IPAmbLightBrightness_enum_Inproc/1  "VBCM_User6IPAmbLightBrightness_enum"
  VBCM_User6IPAmbLightBrightness_enum_Inproc/1 -> UnitConverter224/1
  UnitConverter224/1 -> VOUTP_User6IPAmbLightBrightness_enum/1  "VOUTP_User6IPAmbLightBrightness_enum"
  VBCM_User1AmbLightColor_enum/1 -> VBCM_User1AmbLightColor_enum_Inproc/1  "VBCM_User1AmbLightColor_enum"
  VBCM_User1AmbLightColor_enum_Inproc/1 -> UnitConverter225/1
  UnitConverter225/1 -> VOUTP_User1AmbLightColor_enum/1  "VOUTP_User1AmbLightColor_enum"
  VBCM_User2AmbLightColor_enum/1 -> VBCM_User2AmbLightColor_enum_Inproc/1  "VBCM_User2AmbLightColor_enum"
  VBCM_User2AmbLightColor_enum_Inproc/1 -> UnitConverter226/1
  UnitConverter226/1 -> VOUTP_User2AmbLightColor_enum/1  "VOUTP_User2AmbLightColor_enum"
  VBCM_User3AmbLightColor_enum/1 -> VBCM_User3AmbLightColor_enum_Inproc/1  "VBCM_User3AmbLightColor_enum"
  VBCM_User3AmbLightColor_enum_Inproc/1 -> UnitConverter227/1
  UnitConverter227/1 -> VOUTP_User3AmbLightColor_enum/1  "VOUTP_User3AmbLightColor_enum"
  VBCM_User4AmbLightColor_enum/1 -> VBCM_User4AmbLightColor_enum_Inproc/1  "VBCM_User4AmbLightColor_enum"
  VBCM_User4AmbLightColor_enum_Inproc/1 -> UnitConverter228/1
  UnitConverter228/1 -> VOUTP_User4AmbLightColor_enum/1  "VOUTP_User4AmbLightColor_enum"
  VBCM_User5AmbLightColor_enum/1 -> VBCM_User5AmbLightColor_enum_Inproc/1  "VBCM_User5AmbLightColor_enum"
  VBCM_User5AmbLightColor_enum_Inproc/1 -> UnitConverter229/1
  UnitConverter229/1 -> VOUTP_User5AmbLightColor_enum/1  "VOUTP_User5AmbLightColor_enum"
  VBCM_User6AmbLightColor_enum/1 -> VBCM_User6AmbLightColor_enum_Inproc/1  "VBCM_User6AmbLightColor_enum"
  VBCM_User6AmbLightColor_enum_Inproc/1 -> UnitConverter230/1
  UnitConverter230/1 -> VOUTP_User6AmbLightColor_enum/1  "VOUTP_User6AmbLightColor_enum"
  VBCM_AmbLightBreath1_flg/1 -> VBCM_AmbLightBreath1_flg_Inproc/1  "VBCM_AmbLightBreath1_flg"
  VBCM_AmbLightBreath1_flg_Inproc/1 -> UnitConverter231/1
  UnitConverter231/1 -> VOUTP_AmbLightBreath1_flg/1  "VOUTP_AmbLightBreath1_flg"
  VBCM_AmbLightBreath2_flg/1 -> VBCM_AmbLightBreath2_flg_Inproc/1  "VBCM_AmbLightBreath2_flg"
  VBCM_AmbLightBreath2_flg_Inproc/1 -> UnitConverter232/1
  UnitConverter232/1 -> VOUTP_AmbLightBreath2_flg/1  "VOUTP_AmbLightBreath2_flg"
  VBCM_AmbLightBreath3_flg/1 -> VBCM_AmbLightBreath3_flg_Inproc/1  "VBCM_AmbLightBreath3_flg"
  VBCM_AmbLightBreath3_flg_Inproc/1 -> UnitConverter233/1
  UnitConverter233/1 -> VOUTP_AmbLightBreath3_flg/1  "VOUTP_AmbLightBreath3_flg"
  VBCM_AmbLightBrightness1_enum/1 -> VBCM_AmbLightBrightness1_enum_Inproc/1  "VBCM_AmbLightBrightness1_enum"
  VBCM_AmbLightBrightness1_enum_Inproc/1 -> UnitConverter234/1
  UnitConverter234/1 -> VOUTP_AmbLightBrightness1_enum/1  "VOUTP_AmbLightBrightness1_enum"
  VBCM_AmbLightBrightness2_enum/1 -> VBCM_AmbLightBrightness2_enum_Inproc/1  "VBCM_AmbLightBrightness2_enum"
  VBCM_AmbLightBrightness2_enum_Inproc/1 -> UnitConverter235/1
  UnitConverter235/1 -> VOUTP_AmbLightBrightness2_enum/1  "VOUTP_AmbLightBrightness2_enum"
  VBCM_AmbLightBrightness3_enum/1 -> VBCM_AmbLightBrightness3_enum_Inproc/1  "VBCM_AmbLightBrightness3_enum"
  VBCM_AmbLightBrightness3_enum_Inproc/1 -> UnitConverter236/1
  UnitConverter236/1 -> VOUTP_AmbLightBrightness3_enum/1  "VOUTP_AmbLightBrightness3_enum"
  VBCM_AmbLightColor1_enum/1 -> VBCM_AmbLightColor1_enum_Inproc/1  "VBCM_AmbLightColor1_enum"
  VBCM_AmbLightColor1_enum_Inproc/1 -> UnitConverter237/1
  UnitConverter237/1 -> VOUTP_AmbLightColor1_enum/1  "VOUTP_AmbLightColor1_enum"
  VBCM_AmbLightColor2_enum/1 -> VBCM_AmbLightColor2_enum_Inproc/1  "VBCM_AmbLightColor2_enum"
  VBCM_AmbLightColor2_enum_Inproc/1 -> UnitConverter238/1
  UnitConverter238/1 -> VOUTP_AmbLightColor2_enum/1  "VOUTP_AmbLightColor2_enum"
  VBCM_AmbLightColor3_enum/1 -> VBCM_AmbLightColor3_enum_Inproc/1  "VBCM_AmbLightColor3_enum"
  VBCM_AmbLightColor3_enum_Inproc/1 -> UnitConverter239/1
  UnitConverter239/1 -> VOUTP_AmbLightColor3_enum/1  "VOUTP_AmbLightColor3_enum"
  VBCM_LampPwr_flg/1 -> VBCM_LampPwr_flg_Inproc/1  "VBCM_LampPwr_flg"
  VBCM_LampPwr_flg_Inproc/1 -> UnitConverter240/1
  UnitConverter240/1 -> VOUTP_LampPwr_flg/1  "VOUTP_LampPwr_flg"
  VBCM_SPTGDet_flg/1 -> VBCM_SPTGDet_flg_Inproc/1  "VBCM_SPTGDet_flg"
  VBCM_SPTGDet_flg_Inproc/1 -> UnitConverter241/1
  UnitConverter241/1 -> VOUTP_SPTGDet_flg/1  "VOUTP_SPTGDet_flg"
  VBCM_APSOpenPTG_flg/1 -> VBCM_APSOpenPTG_flg_Inproc/1  "VBCM_APSOpenPTG_flg"
  VBCM_APSOpenPTG_flg_Inproc/1 -> UnitConverter242/1
  UnitConverter242/1 -> VOUTP_APSOpenPTG_flg/1  "VOUTP_APSOpenPTG_flg"
  VBCM_FollowMe_flg/1 -> VBCM_FollowMe_flg_Inproc/1  "VBCM_FollowMe_flg"
  VBCM_FollowMe_flg_Inproc/1 -> UnitConverter243/1
  UnitConverter243/1 -> VOUTP_FollowMe_flg/1  "VOUTP_FollowMe_flg"
  VBCM_IVIRST_flg/1 -> VBCM_IVIRST_flg_Inproc/1  "VBCM_IVIRST_flg"
  VBCM_IVIRST_flg_Inproc/1 -> UnitConverter244/1
  UnitConverter244/1 -> VOUTP_IVIRST_flg/1  "VOUTP_IVIRST_flg"
  VBCM_CountAlarm_enum/1 -> VBCM_CountAlarm_enum_Inproc/1  "VBCM_CountAlarm_enum"
  VBCM_CountAlarm_enum_Inproc/1 -> UnitConverter245/1
  UnitConverter245/1 -> VOUTP_CountAlarm_enum/1  "VOUTP_CountAlarm_enum"
  VBCM_MFSWTri_flg/1 -> VBCM_MFSWTri_flg_Inproc/1  "VBCM_MFSWTri_flg"
  VBCM_MFSWTri_flg_Inproc/1 -> UnitConverter246/1
  UnitConverter246/1 -> VOUTP_MFSWTri_flg/1  "VOUTP_MFSWTri_flg"
  VBCM_MirrorFlodPos_flg/1 -> VBCM_MirrorFlodPos_flg_Inproc/1  "VBCM_MirrorFlodPos_flg"
  VBCM_MirrorFlodPos_flg_Inproc/1 -> UnitConverter247/1
  UnitConverter247/1 -> VOUTP_MirrorFlodPos_flg/1  "VOUTP_MirrorFlodPos_flg"
  VBCM_FuelDoorPos_flg/1 -> VBCM_FuelDoorPos_flg_Inproc/1  "VBCM_FuelDoorPos_flg"
  VBCM_FuelDoorPos_flg_Inproc/1 -> UnitConverter248/1
  UnitConverter248/1 -> VOUTP_FuelDoorPos_flg/1  "VOUTP_FuelDoorPos_flg"
  VBCM_MFRDNBrightReq_pct/1 -> VBCM_MFRDNBrightReq_pct_Inproc/1  "VBCM_MFRDNBrightReq_pct"
  VBCM_MFRDNBrightReq_pct_Inproc/1 -> UnitConverter249/1
  UnitConverter249/1 -> VOUTP_MFRDNBrightReq_pct/1  "VOUTP_MFRDNBrightReq_pct"
  VBCM_RoomLampMode_flg/1 -> VBCM_RoomLampMode_flg_Inproc/1  "VBCM_RoomLampMode_flg"
  VBCM_RoomLampMode_flg_Inproc/1 -> UnitConverter250/1
  UnitConverter250/1 -> VOUTP_RoomLampMode_flg/1  "VOUTP_RoomLampMode_flg"
  VBCM_IVIPTGUSStaSW_flg/1 -> VBCM_IVIPTGUSStaSW_flg_Inproc/1  "VBCM_IVIPTGUSStaSW_flg"
  VBCM_IVIPTGUSStaSW_flg_Inproc/1 -> UnitConverter251/1
  UnitConverter251/1 -> VOUTP_IVIPTGUSStaSW_flg/1  "VOUTP_IVIPTGUSStaSW_flg"
  VBCM_PTGInnerSW2_enum/1 -> VBCM_PTGInnerSW2_enum_Inproc/1  "VBCM_PTGInnerSW2_enum"
  VBCM_PTGInnerSW2_enum_Inproc/1 -> UnitConverter252/1
  UnitConverter252/1 -> VOUTP_PTGInnerSW2_enum/1  "VOUTP_PTGInnerSW2_enum"
  VBCM_LDrvCtrlCmd_pct/1 -> VBCM_LDrvCtrlCmd_pct_Inproc/1  "VBCM_LDrvCtrlCmd_pct"
  VBCM_LDrvCtrlCmd_pct_Inproc/1 -> UnitConverter253/1
  UnitConverter253/1 -> VOUTP_LDrvCtrlCmd_pct/1  "VOUTP_LDrvCtrlCmd_pct"
  VBCM_LPasCtrlCmd_pct/1 -> VBCM_LPasCtrlCmd_pct_Inproc/1  "VBCM_LPasCtrlCmd_pct"
  VBCM_LPasCtrlCmd_pct_Inproc/1 -> UnitConverter254/1
  UnitConverter254/1 -> VOUTP_LPasCtrlCmd_pct/1  "VOUTP_LPasCtrlCmd_pct"
  VBCM_LRLDCtrlCmd_pct/1 -> VBCM_LRLDCtrlCmd_pct_Inproc/1  "VBCM_LRLDCtrlCmd_pct"
  VBCM_LRLDCtrlCmd_pct_Inproc/1 -> UnitConverter255/1
  UnitConverter255/1 -> VOUTP_LRLDCtrlCmd_pct/1  "VOUTP_LRLDCtrlCmd_pct"
  VBCM_LRRDCtrlCmd_pct/1 -> VBCM_LRRDCtrlCmd_pct_Inproc/1  "VBCM_LRRDCtrlCmd_pct"
  VBCM_LRRDCtrlCmd_pct_Inproc/1 -> UnitConverter256/1
  UnitConverter256/1 -> VOUTP_LRRDCtrlCmd_pct/1  "VOUTP_LRRDCtrlCmd_pct"
  VBCM_APMDoorControlSta_flg/1 -> VBCM_APMDoorControlSta_flg_Inproc/1  "VBCM_APMDoorControlSta_flg"
  VBCM_APMDoorControlSta_flg_Inproc/1 -> UnitConverter257/1
  UnitConverter257/1 -> VOUTP_APMDoorControlSta_flg/1  "VOUTP_APMDoorControlSta_flg"
  VBCM_LockAlarm_enum/1 -> VBCM_LockAlarm_enum_Inproc/1  "VBCM_LockAlarm_enum"
  VBCM_LockAlarm_enum_Inproc/1 -> UnitConverter258/1
  UnitConverter258/1 -> VOUTP_LockAlarm_enum/1  "VOUTP_LockAlarm_enum"
  VBCM_ATCtrl_enum/1 -> VBCM_ATCtrl_enum_Inproc/1  "VBCM_ATCtrl_enum"
  VBCM_ATCtrl_enum_Inproc/1 -> UnitConverter259/1
  UnitConverter259/1 -> VOUTP_ATCtrl_enum/1  "VOUTP_ATCtrl_enum"
  VBCM_fUnlockSingle_flg/1 -> VBCM_fUnlockSingle_flg_Inproc/1  "VBCM_fUnlockSingle_flg"
  VBCM_fUnlockSingle_flg_Inproc/1 -> UnitConverter260/1
  UnitConverter260/1 -> VOUTP_fUnlockSingle_flg/1  "VOUTP_fUnlockSingle_flg"
  VBCM_OutMode_enum/1 -> VBCM_OutMode_enum_Inproc/1  "VBCM_OutMode_enum"
  VBCM_OutMode_enum_Inproc/1 -> UnitConverter261/1
  UnitConverter261/1 -> VOUTP_OutMode_enum/1  "VOUTP_OutMode_enum"
  VDDM_C3BMS6RCDTC_raw32/1 -> VDDM_C3BMS6RCDTC_raw32_Inproc/1  "VDDM_C3BMS6RCDTC_raw32"
  VDDM_C3BMS6RCDTC_raw32_Inproc/1 -> UnitConverter262/1
  UnitConverter262/1 -> VOUTP_C3BMS6RCDTC_raw32/1  "VOUTP_C3BMS6RCDTC_raw32"
  VDDM_C3BMS6CSDTC_raw32/1 -> VDDM_C3BMS6CSDTC_raw32_Inproc/1  "VDDM_C3BMS6CSDTC_raw32"
  VDDM_C3BMS6CSDTC_raw32_Inproc/1 -> UnitConverter263/1
  UnitConverter263/1 -> VOUTP_C3BMS6CSDTC_raw32/1  "VOUTP_C3BMS6CSDTC_raw32"
  VDDM_C3BMS6LCDTC_raw32/1 -> VDDM_C3BMS6LCDTC_raw32_Inproc/1  "VDDM_C3BMS6LCDTC_raw32"
  VDDM_C3BMS6LCDTC_raw32_Inproc/1 -> UnitConverter264/1
  UnitConverter264/1 -> VOUTP_C3BMS6LCDTC_raw32/1  "VOUTP_C3BMS6LCDTC_raw32"
  VDDM_C3BMS1RCDTC_raw32/1 -> VDDM_C3BMS1RCDTC_raw32_Inproc/1  "VDDM_C3BMS1RCDTC_raw32"
  VDDM_C3BMS1RCDTC_raw32_Inproc/1 -> UnitConverter265/1
  UnitConverter265/1 -> VOUTP_C3BMS1RCDTC_raw32/1  "VOUTP_C3BMS1RCDTC_raw32"
  VDDM_C3BMS1CSDTC_raw32/1 -> VDDM_C3BMS1CSDTC_raw32_Inproc/1  "VDDM_C3BMS1CSDTC_raw32"
  VDDM_C3BMS1CSDTC_raw32_Inproc/1 -> UnitConverter266/1
  UnitConverter266/1 -> VOUTP_C3BMS1CSDTC_raw32/1  "VOUTP_C3BMS1CSDTC_raw32"
  VDDM_C3BMS1LCDTC_raw32/1 -> VDDM_C3BMS1LCDTC_raw32_Inproc/1  "VDDM_C3BMS1LCDTC_raw32"
  VDDM_C3BMS1LCDTC_raw32_Inproc/1 -> UnitConverter267/1
  UnitConverter267/1 -> VOUTP_C3BMS1LCDTC_raw32/1  "VOUTP_C3BMS1LCDTC_raw32"
  VDDM_C3CCU1RCDTC_raw32/1 -> VDDM_C3CCU1RCDTC_raw32_Inproc/1  "VDDM_C3CCU1RCDTC_raw32"
  VDDM_C3CCU1RCDTC_raw32_Inproc/1 -> UnitConverter268/1
  UnitConverter268/1 -> VOUTP_C3CCU1RCDTC_raw32/1  "VOUTP_C3CCU1RCDTC_raw32"
  VDDM_C3CCU1CSDTC_raw32/1 -> VDDM_C3CCU1CSDTC_raw32_Inproc/1  "VDDM_C3CCU1CSDTC_raw32"
  VDDM_C3CCU1CSDTC_raw32_Inproc/1 -> UnitConverter269/1
  UnitConverter269/1 -> VOUTP_C3CCU1CSDTC_raw32/1  "VOUTP_C3CCU1CSDTC_raw32"
  VDDM_C3CCU1LCDTC_raw32/1 -> VDDM_C3CCU1LCDTC_raw32_Inproc/1  "VDDM_C3CCU1LCDTC_raw32"
  VDDM_C3CCU1LCDTC_raw32_Inproc/1 -> UnitConverter270/1
  UnitConverter270/1 -> VOUTP_C3CCU1LCDTC_raw32/1  "VOUTP_C3CCU1LCDTC_raw32"
  VDDM_C3CCU2RCDTC_raw32/1 -> VDDM_C3CCU2RCDTC_raw32_Inproc/1  "VDDM_C3CCU2RCDTC_raw32"
  VDDM_C3CCU2RCDTC_raw32_Inproc/1 -> UnitConverter271/1
  UnitConverter271/1 -> VOUTP_C3CCU2RCDTC_raw32/1  "VOUTP_C3CCU2RCDTC_raw32"
  VDDM_C3CCU2CSDTC_raw32/1 -> VDDM_C3CCU2CSDTC_raw32_Inproc/1  "VDDM_C3CCU2CSDTC_raw32"
  VDDM_C3CCU2CSDTC_raw32_Inproc/1 -> UnitConverter272/1
  UnitConverter272/1 -> VOUTP_C3CCU2CSDTC_raw32/1  "VOUTP_C3CCU2CSDTC_raw32"
  VDDM_C3CCU2LCDTC_raw32/1 -> VDDM_C3CCU2LCDTC_raw32_Inproc/1  "VDDM_C3CCU2LCDTC_raw32"
  VDDM_C3CCU2LCDTC_raw32_Inproc/1 -> UnitConverter273/1
  UnitConverter273/1 -> VOUTP_C3CCU2LCDTC_raw32/1  "VOUTP_C3CCU2LCDTC_raw32"
  VDDM_C1ABM1RCDTC_raw32/1 -> VDDM_C1ABM1RCDTC_raw32_Inproc/1  "VDDM_C1ABM1RCDTC_raw32"
  VDDM_C1ABM1RCDTC_raw32_Inproc/1 -> UnitConverter274/1
  UnitConverter274/1 -> VOUTP_C1ABM1RCDTC_raw32/1  "VOUTP_C1ABM1RCDTC_raw32"
  VDDM_C1ABM1CSDTC_raw32/1 -> VDDM_C1ABM1CSDTC_raw32_Inproc/1  "VDDM_C1ABM1CSDTC_raw32"
  VDDM_C1ABM1CSDTC_raw32_Inproc/1 -> UnitConverter275/1
  UnitConverter275/1 -> VOUTP_C1ABM1CSDTC_raw32/1  "VOUTP_C1ABM1CSDTC_raw32"
  VDDM_C1ABM1LCDTC_raw32/1 -> VDDM_C1ABM1LCDTC_raw32_Inproc/1  "VDDM_C1ABM1LCDTC_raw32"
  VDDM_C1ABM1LCDTC_raw32_Inproc/1 -> UnitConverter276/1
  UnitConverter276/1 -> VOUTP_C1ABM1LCDTC_raw32/1  "VOUTP_C1ABM1LCDTC_raw32"
  VDDM_Lv1ErrDTC_raw32/1 -> VDDM_Lv1ErrDTC_raw32_Inproc/1  "VDDM_Lv1ErrDTC_raw32"
  VDDM_Lv1ErrDTC_raw32_Inproc/1 -> UnitConverter277/1
  UnitConverter277/1 -> VOUTP_Lv1ErrDTC_raw32/1  "VOUTP_Lv1ErrDTC_raw32"
  VDDM_Lv2ErrDTC_raw32/1 -> VDDM_Lv2ErrDTC_raw32_Inproc/1  "VDDM_Lv2ErrDTC_raw32"
  VDDM_Lv2ErrDTC_raw32_Inproc/1 -> UnitConverter278/1
  UnitConverter278/1 -> VOUTP_Lv2ErrDTC_raw32/1  "VOUTP_Lv2ErrDTC_raw32"
  VDDM_Lv3ErrDTC_raw32/1 -> VDDM_Lv3ErrDTC_raw32_Inproc/1  "VDDM_Lv3ErrDTC_raw32"
  VDDM_Lv3ErrDTC_raw32_Inproc/1 -> UnitConverter279/1
  UnitConverter279/1 -> VOUTP_Lv3ErrDTC_raw32/1  "VOUTP_Lv3ErrDTC_raw32"
  VDDM_Lv4ErrDTC_raw32/1 -> VDDM_Lv4ErrDTC_raw32_Inproc/1  "VDDM_Lv4ErrDTC_raw32"
  VDDM_Lv4ErrDTC_raw32_Inproc/1 -> UnitConverter280/1
  UnitConverter280/1 -> VOUTP_Lv4ErrDTC_raw32/1  "VOUTP_Lv4ErrDTC_raw32"
  VDDM_BrkSWErrDTC_raw32/1 -> VDDM_BrkSWErrDTC_raw32_Inproc/1  "VDDM_BrkSWErrDTC_raw32"
  VDDM_BrkSWErrDTC_raw32_Inproc/1 -> UnitConverter281/1
  UnitConverter281/1 -> VOUTP_BrkSWErrDTC_raw32/1  "VOUTP_BrkSWErrDTC_raw32"
  VDDM_BrkSWNoBacDTC_raw32/1 -> VDDM_BrkSWNoBacDTC_raw32_Inproc/1  "VDDM_BrkSWNoBacDTC_raw32"
  VDDM_BrkSWNoBacDTC_raw32_Inproc/1 -> UnitConverter282/1
  UnitConverter282/1 -> VOUTP_BrkSWNoBacDTC_raw32/1  "VOUTP_BrkSWNoBacDTC_raw32"
  VDDM_KeyAuthDTC_raw32/1 -> VDDM_KeyAuthDTC_raw32_Inproc/1  "VDDM_KeyAuthDTC_raw32"
  VDDM_KeyAuthDTC_raw32_Inproc/1 -> UnitConverter283/1
  UnitConverter283/1 -> VOUTP_KeyAuthDTC_raw32/1  "VOUTP_KeyAuthDTC_raw32"
  VDDM_ONtoRdyDTC_raw32/1 -> VDDM_ONtoRdyDTC_raw32_Inproc/1  "VDDM_ONtoRdyDTC_raw32"
  VDDM_ONtoRdyDTC_raw32_Inproc/1 -> UnitConverter284/1
  UnitConverter284/1 -> VOUTP_ONtoRdyDTC_raw32/1  "VOUTP_ONtoRdyDTC_raw32"
  VDDM_HVB4PreDTC_raw32/1 -> VDDM_HVB4PreDTC_raw32_Inproc/1  "VDDM_HVB4PreDTC_raw32"
  VDDM_HVB4PreDTC_raw32_Inproc/1 -> UnitConverter285/1
  UnitConverter285/1 -> VOUTP_HVB4PreDTC_raw32/1  "VOUTP_HVB4PreDTC_raw32"
  VDDM_MCU4PreDTC_raw32/1 -> VDDM_MCU4PreDTC_raw32_Inproc/1  "VDDM_MCU4PreDTC_raw32"
  VDDM_MCU4PreDTC_raw32_Inproc/1 -> UnitConverter286/1
  UnitConverter286/1 -> VOUTP_MCU4PreDTC_raw32/1  "VOUTP_MCU4PreDTC_raw32"
  VDDM_DCDC4PreDTC_raw32/1 -> VDDM_DCDC4PreDTC_raw32_Inproc/1  "VDDM_DCDC4PreDTC_raw32"
  VDDM_DCDC4PreDTC_raw32_Inproc/1 -> UnitConverter287/1
  UnitConverter287/1 -> VOUTP_DCDC4PreDTC_raw32/1  "VOUTP_DCDC4PreDTC_raw32"
  VDDM_HVRlyCloDTC_raw32/1 -> VDDM_HVRlyCloDTC_raw32_Inproc/1  "VDDM_HVRlyCloDTC_raw32"
  VDDM_HVRlyCloDTC_raw32_Inproc/1 -> UnitConverter288/1
  UnitConverter288/1 -> VOUTP_HVRlyCloDTC_raw32/1  "VOUTP_HVRlyCloDTC_raw32"
  VDDM_BMSRdyDTC_raw32/1 -> VDDM_BMSRdyDTC_raw32_Inproc/1  "VDDM_BMSRdyDTC_raw32"
  VDDM_BMSRdyDTC_raw32_Inproc/1 -> UnitConverter289/1
  UnitConverter289/1 -> VOUTP_BMSRdyDTC_raw32/1  "VOUTP_BMSRdyDTC_raw32"
  VDDM_DCDCEnaDTC_raw32/1 -> VDDM_DCDCEnaDTC_raw32_Inproc/1  "VDDM_DCDCEnaDTC_raw32"
  VDDM_DCDCEnaDTC_raw32_Inproc/1 -> UnitConverter290/1
  UnitConverter290/1 -> VOUTP_DCDCEnaDTC_raw32/1  "VOUTP_DCDCEnaDTC_raw32"
  VDDM_HiLvSaChkDTC_raw32/1 -> VDDM_HiLvSaChkDTC_raw32_Inproc/1  "VDDM_HiLvSaChkDTC_raw32"
  VDDM_HiLvSaChkDTC_raw32_Inproc/1 -> UnitConverter291/1
  UnitConverter291/1 -> VOUTP_HiLvSaChkDTC_raw32/1  "VOUTP_HiLvSaChkDTC_raw32"
  VDDM_MidLvSaChkDTC_raw32/1 -> VDDM_MidLvSaChkDTC_raw32_Inproc/1  "VDDM_MidLvSaChkDTC_raw32"
  VDDM_MidLvSaChkDTC_raw32_Inproc/1 -> UnitConverter292/1
  UnitConverter292/1 -> VOUTP_MidLvSaChkDTC_raw32/1  "VOUTP_MidLvSaChkDTC_raw32"
  VDDM_MCUDisDTC_raw32/1 -> VDDM_MCUDisDTC_raw32_Inproc/1  "VDDM_MCUDisDTC_raw32"
  VDDM_MCUDisDTC_raw32_Inproc/1 -> UnitConverter293/1
  UnitConverter293/1 -> VOUTP_MCUDisDTC_raw32/1  "VOUTP_MCUDisDTC_raw32"
  VDDM_DCDCDisDTC_raw32/1 -> VDDM_DCDCDisDTC_raw32_Inproc/1  "VDDM_DCDCDisDTC_raw32"
  VDDM_DCDCDisDTC_raw32_Inproc/1 -> UnitConverter294/1
  UnitConverter294/1 -> VOUTP_DCDCDisDTC_raw32/1  "VOUTP_DCDCDisDTC_raw32"
  VDDM_HVRlyOpDTC_raw32/1 -> VDDM_HVRlyOpDTC_raw32_Inproc/1  "VDDM_HVRlyOpDTC_raw32"
  VDDM_HVRlyOpDTC_raw32_Inproc/1 -> UnitConverter295/1
  UnitConverter295/1 -> VOUTP_HVRlyOpDTC_raw32/1  "VOUTP_HVRlyOpDTC_raw32"
  VDDM_MCUActDTC_raw32/1 -> VDDM_MCUActDTC_raw32_Inproc/1  "VDDM_MCUActDTC_raw32"
  VDDM_MCUActDTC_raw32_Inproc/1 -> UnitConverter296/1
  UnitConverter296/1 -> VOUTP_MCUActDTC_raw32/1  "VOUTP_MCUActDTC_raw32"
  VDDM_OBC4PreDTC_raw32/1 -> VDDM_OBC4PreDTC_raw32_Inproc/1  "VDDM_OBC4PreDTC_raw32"
  VDDM_OBC4PreDTC_raw32_Inproc/1 -> UnitConverter297/1
  UnitConverter297/1 -> VOUTP_OBC4PreDTC_raw32/1  "VOUTP_OBC4PreDTC_raw32"
  VDDM_IniLVLoDTC_raw32/1 -> VDDM_IniLVLoDTC_raw32_Inproc/1  "VDDM_IniLVLoDTC_raw32"
  VDDM_IniLVLoDTC_raw32_Inproc/1 -> UnitConverter298/1
  UnitConverter298/1 -> VOUTP_IniLVLoDTC_raw32/1  "VOUTP_IniLVLoDTC_raw32"
  VDDM_LVSupLoDTC_raw32/1 -> VDDM_LVSupLoDTC_raw32_Inproc/1  "VDDM_LVSupLoDTC_raw32"
  VDDM_LVSupLoDTC_raw32_Inproc/1 -> UnitConverter299/1
  UnitConverter299/1 -> VOUTP_LVSupLoDTC_raw32/1  "VOUTP_LVSupLoDTC_raw32"
  VDDM_LVSupHiDTC_raw32/1 -> VDDM_LVSupHiDTC_raw32_Inproc/1  "VDDM_LVSupHiDTC_raw32"
  VDDM_LVSupHiDTC_raw32_Inproc/1 -> UnitConverter300/1
  UnitConverter300/1 -> VOUTP_LVSupHiDTC_raw32/1  "VOUTP_LVSupHiDTC_raw32"
  VDDM_DrStSWDTC_raw32/1 -> VDDM_DrStSWDTC_raw32_Inproc/1  "VDDM_DrStSWDTC_raw32"
  VDDM_DrStSWDTC_raw32_Inproc/1 -> UnitConverter301/1
  UnitConverter301/1 -> VOUTP_DrStSWDTC_raw32/1  "VOUTP_DrStSWDTC_raw32"
  VDDM_FLDoorSWDTC_raw32/1 -> VDDM_FLDoorSWDTC_raw32_Inproc/1  "VDDM_FLDoorSWDTC_raw32"
  VDDM_FLDoorSWDTC_raw32_Inproc/1 -> UnitConverter302/1
  UnitConverter302/1 -> VOUTP_FLDoorSWDTC_raw32/1  "VOUTP_FLDoorSWDTC_raw32"
  VDDM_RLDoorSWDTC_raw32/1 -> VDDM_RLDoorSWDTC_raw32_Inproc/1  "VDDM_RLDoorSWDTC_raw32"
  VDDM_RLDoorSWDTC_raw32_Inproc/1 -> UnitConverter303/1
  UnitConverter303/1 -> VOUTP_RLDoorSWDTC_raw32/1  "VOUTP_RLDoorSWDTC_raw32"
  VDDM_FRDoorSWDTC_raw32/1 -> VDDM_FRDoorSWDTC_raw32_Inproc/1  "VDDM_FRDoorSWDTC_raw32"
  VDDM_FRDoorSWDTC_raw32_Inproc/1 -> UnitConverter304/1
  UnitConverter304/1 -> VOUTP_FRDoorSWDTC_raw32/1  "VOUTP_FRDoorSWDTC_raw32"
  VDDM_RRDoorSWDTC_raw32/1 -> VDDM_RRDoorSWDTC_raw32_Inproc/1  "VDDM_RRDoorSWDTC_raw32"
  VDDM_RRDoorSWDTC_raw32_Inproc/1 -> UnitConverter305/1
  UnitConverter305/1 -> VOUTP_RRDoorSWDTC_raw32/1  "VOUTP_RRDoorSWDTC_raw32"
  VDDM_HoodSWDTC_raw32/1 -> VDDM_HoodSWDTC_raw32_Inproc/1  "VDDM_HoodSWDTC_raw32"
  VDDM_HoodSWDTC_raw32_Inproc/1 -> UnitConverter306/1
  UnitConverter306/1 -> VOUTP_HoodSWDTC_raw32/1  "VOUTP_HoodSWDTC_raw32"
  VDDM_TailgaSWDTC_raw32/1 -> VDDM_TailgaSWDTC_raw32_Inproc/1  "VDDM_TailgaSWDTC_raw32"
  VDDM_TailgaSWDTC_raw32_Inproc/1 -> UnitConverter307/1
  UnitConverter307/1 -> VOUTP_TailgaSWDTC_raw32/1  "VOUTP_TailgaSWDTC_raw32"
  VDDM_VehMalfunLevel_enum/1 -> VDDM_VehMalfunLevel_enum_Inproc/1  "VDDM_VehMalfunLevel_enum"
  VDDM_VehMalfunLevel_enum_Inproc/1 -> UnitConverter308/1
  UnitConverter308/1 -> VOUTP_VehMalfunLevel_enum/1  "VOUTP_VehMalfunLevel_enum"
  VDDM_APS1SigOoRDTC_raw32/1 -> VDDM_APS1SigOoRDTC_raw32_Inproc/1  "VDDM_APS1SigOoRDTC_raw32"
  VDDM_APS1SigOoRDTC_raw32_Inproc/1 -> UnitConverter309/1
  UnitConverter309/1 -> VOUTP_APS1SigOoRDTC_raw32/1  "VOUTP_APS1SigOoRDTC_raw32"
  VDDM_APS2SigOoRDTC_raw32/1 -> VDDM_APS2SigOoRDTC_raw32_Inproc/1  "VDDM_APS2SigOoRDTC_raw32"
  VDDM_APS2SigOoRDTC_raw32_Inproc/1 -> UnitConverter310/1
  UnitConverter310/1 -> VOUTP_APS2SigOoRDTC_raw32/1  "VOUTP_APS2SigOoRDTC_raw32"
  VDDM_APSCorrErrDTC_raw32/1 -> VDDM_APSCorrErrDTC_raw32_Inproc/1  "VDDM_APSCorrErrDTC_raw32"
  VDDM_APSCorrErrDTC_raw32_Inproc/1 -> UnitConverter311/1
  UnitConverter311/1 -> VOUTP_APSCorrErrDTC_raw32/1  "VOUTP_APSCorrErrDTC_raw32"
  VDDM_MCUF1NoComDTC_raw32/1 -> VDDM_MCUF1NoComDTC_raw32_Inproc/1  "VDDM_MCUF1NoComDTC_raw32"
  VDDM_MCUF1NoComDTC_raw32_Inproc/1 -> UnitConverter312/1
  UnitConverter312/1 -> VOUTP_MCUF1NoComDTC_raw32/1  "VOUTP_MCUF1NoComDTC_raw32"
  VDDM_MCUR1NoComDTC_raw32/1 -> VDDM_MCUR1NoComDTC_raw32_Inproc/1  "VDDM_MCUR1NoComDTC_raw32"
  VDDM_MCUR1NoComDTC_raw32_Inproc/1 -> UnitConverter313/1
  UnitConverter313/1 -> VOUTP_MCUR1NoComDTC_raw32/1  "VOUTP_MCUR1NoComDTC_raw32"
  VDDM_Shifter1NoComDTC_raw32/1 -> VDDM_Shifter1NoComDTC_raw32_Inproc/1  "VDDM_Shifter1NoComDTC_raw32"
  VDDM_Shifter1NoComDTC_raw32_Inproc/1 -> UnitConverter314/1
  UnitConverter314/1 -> VOUTP_Shifter1NoComDTC_raw32/1  "VOUTP_Shifter1NoComDTC_raw32"
  VDDM_ESC7NoComDTC_raw32/1 -> VDDM_ESC7NoComDTC_raw32_Inproc/1  "VDDM_ESC7NoComDTC_raw32"
  VDDM_ESC7NoComDTC_raw32_Inproc/1 -> UnitConverter315/1
  UnitConverter315/1 -> VOUTP_ESC7NoComDTC_raw32/1  "VOUTP_ESC7NoComDTC_raw32"
  VDDM_ESC1NoComDTC_raw32/1 -> VDDM_ESC1NoComDTC_raw32_Inproc/1  "VDDM_ESC1NoComDTC_raw32"
  VDDM_ESC1NoComDTC_raw32_Inproc/1 -> UnitConverter316/1
  UnitConverter316/1 -> VOUTP_ESC1NoComDTC_raw32/1  "VOUTP_ESC1NoComDTC_raw32"
  VDDM_ESC5NoComDTC_raw32/1 -> VDDM_ESC5NoComDTC_raw32_Inproc/1  "VDDM_ESC5NoComDTC_raw32"
  VDDM_ESC5NoComDTC_raw32_Inproc/1 -> UnitConverter317/1
  UnitConverter317/1 -> VOUTP_ESC5NoComDTC_raw32/1  "VOUTP_ESC5NoComDTC_raw32"
  VDDM_EnterNewOperCyc_flg/1 -> VDDM_EnterNewOperCyc_flg_Inproc/1  "VDDM_EnterNewOperCyc_flg"
  VDDM_EnterNewOperCyc_flg_Inproc/1 -> UnitConverter318/1
  UnitConverter318/1 -> VOUTP_EnterNewOperCyc_flg/1  "VOUTP_EnterNewOperCyc_flg"
  VDDM_DiagHCrashDTC_raw32/1 -> VDDM_DiagHCrashDTC_raw32_Inproc/1  "VDDM_DiagHCrashDTC_raw32"
  VDDM_DiagHCrashDTC_raw32_Inproc/1 -> UnitConverter319/1
  UnitConverter319/1 -> VOUTP_DiagHCrashDTC_raw32/1  "VOUTP_DiagHCrashDTC_raw32"
  VDDM_DiagFLTSDTC_raw32/1 -> VDDM_DiagFLTSDTC_raw32_Inproc/1  "VDDM_DiagFLTSDTC_raw32"
  VDDM_DiagFLTSDTC_raw32_Inproc/1 -> UnitConverter320/1
  UnitConverter320/1 -> VOUTP_DiagFLTSDTC_raw32/1  "VOUTP_DiagFLTSDTC_raw32"
  VDDM_DiagFRTSDTC_raw32/1 -> VDDM_DiagFRTSDTC_raw32_Inproc/1  "VDDM_DiagFRTSDTC_raw32"
  VDDM_DiagFRTSDTC_raw32_Inproc/1 -> UnitConverter321/1
  UnitConverter321/1 -> VOUTP_DiagFRTSDTC_raw32/1  "VOUTP_DiagFRTSDTC_raw32"
  VDDM_DiagRLTSDTC_raw32/1 -> VDDM_DiagRLTSDTC_raw32_Inproc/1  "VDDM_DiagRLTSDTC_raw32"
  VDDM_DiagRLTSDTC_raw32_Inproc/1 -> UnitConverter322/1
  UnitConverter322/1 -> VOUTP_DiagRLTSDTC_raw32/1  "VOUTP_DiagRLTSDTC_raw32"
  VDDM_DiagRRTSDTC_raw32/1 -> VDDM_DiagRRTSDTC_raw32_Inproc/1  "VDDM_DiagRRTSDTC_raw32"
  VDDM_DiagRRTSDTC_raw32_Inproc/1 -> UnitConverter323/1
  UnitConverter323/1 -> VOUTP_DiagRRTSDTC_raw32/1  "VOUTP_DiagRRTSDTC_raw32"
  VDDM_FCLUSSDTC_raw32/1 -> VDDM_FCLUSSDTC_raw32_Inproc/1  "VDDM_FCLUSSDTC_raw32"
  VDDM_FCLUSSDTC_raw32_Inproc/1 -> UnitConverter324/1
  UnitConverter324/1 -> VOUTP_FCLUSSDTC_raw32/1  "VOUTP_FCLUSSDTC_raw32"
  VDDM_FMLUSSDTC_raw32/1 -> VDDM_FMLUSSDTC_raw32_Inproc/1  "VDDM_FMLUSSDTC_raw32"
  VDDM_FMLUSSDTC_raw32_Inproc/1 -> UnitConverter325/1
  UnitConverter325/1 -> VOUTP_FMLUSSDTC_raw32/1  "VOUTP_FMLUSSDTC_raw32"
  VDDM_FMRUSSDTC_raw32/1 -> VDDM_FMRUSSDTC_raw32_Inproc/1  "VDDM_FMRUSSDTC_raw32"
  VDDM_FMRUSSDTC_raw32_Inproc/1 -> UnitConverter326/1
  UnitConverter326/1 -> VOUTP_FMRUSSDTC_raw32/1  "VOUTP_FMRUSSDTC_raw32"
  VDDM_FCRUSSDTC_raw32/1 -> VDDM_FCRUSSDTC_raw32_Inproc/1  "VDDM_FCRUSSDTC_raw32"
  VDDM_FCRUSSDTC_raw32_Inproc/1 -> UnitConverter327/1
  UnitConverter327/1 -> VOUTP_FCRUSSDTC_raw32/1  "VOUTP_FCRUSSDTC_raw32"
  VDDM_RCLUSSDTC_raw32/1 -> VDDM_RCLUSSDTC_raw32_Inproc/1  "VDDM_RCLUSSDTC_raw32"
  VDDM_RCLUSSDTC_raw32_Inproc/1 -> UnitConverter328/1
  UnitConverter328/1 -> VOUTP_RCLUSSDTC_raw32/1  "VOUTP_RCLUSSDTC_raw32"
  VDDM_RMLUSSDTC_raw32/1 -> VDDM_RMLUSSDTC_raw32_Inproc/1  "VDDM_RMLUSSDTC_raw32"
  VDDM_RMLUSSDTC_raw32_Inproc/1 -> UnitConverter329/1
  UnitConverter329/1 -> VOUTP_RMLUSSDTC_raw32/1  "VOUTP_RMLUSSDTC_raw32"
  VDDM_RMRUSSDTC_raw32/1 -> VDDM_RMRUSSDTC_raw32_Inproc/1  "VDDM_RMRUSSDTC_raw32"
  VDDM_RMRUSSDTC_raw32_Inproc/1 -> UnitConverter330/1
  UnitConverter330/1 -> VOUTP_RMRUSSDTC_raw32/1  "VOUTP_RMRUSSDTC_raw32"
  VDDM_RCRUSSDTC_raw32/1 -> VDDM_RCRUSSDTC_raw32_Inproc/1  "VDDM_RCRUSSDTC_raw32"
  VDDM_RCRUSSDTC_raw32_Inproc/1 -> UnitConverter331/1
  UnitConverter331/1 -> VOUTP_RCRUSSDTC_raw32/1  "VOUTP_RCRUSSDTC_raw32"
  VDDM_FLLUSSDTC_raw32/1 -> VDDM_FLLUSSDTC_raw32_Inproc/1  "VDDM_FLLUSSDTC_raw32"
  VDDM_FLLUSSDTC_raw32_Inproc/1 -> UnitConverter332/1
  UnitConverter332/1 -> VOUTP_FLLUSSDTC_raw32/1  "VOUTP_FLLUSSDTC_raw32"
  VDDM_FLRUSSDTC_raw32/1 -> VDDM_FLRUSSDTC_raw32_Inproc/1  "VDDM_FLRUSSDTC_raw32"
  VDDM_FLRUSSDTC_raw32_Inproc/1 -> UnitConverter333/1
  UnitConverter333/1 -> VOUTP_FLRUSSDTC_raw32/1  "VOUTP_FLRUSSDTC_raw32"
  VDDM_RLLUSSDTC_raw32/1 -> VDDM_RLLUSSDTC_raw32_Inproc/1  "VDDM_RLLUSSDTC_raw32"
  VDDM_RLLUSSDTC_raw32_Inproc/1 -> UnitConverter334/1
  UnitConverter334/1 -> VOUTP_RLLUSSDTC_raw32/1  "VOUTP_RLLUSSDTC_raw32"
  VDDM_RLRUSSDTC_raw32/1 -> VDDM_RLRUSSDTC_raw32_Inproc/1  "VDDM_RLRUSSDTC_raw32"
  VDDM_RLRUSSDTC_raw32_Inproc/1 -> UnitConverter335/1
  UnitConverter335/1 -> VOUTP_RLRUSSDTC_raw32/1  "VOUTP_RLRUSSDTC_raw32"
  VDDM_FCM2NoComDTC_raw32/1 -> VDDM_FCM2NoComDTC_raw32_Inproc/1  "VDDM_FCM2NoComDTC_raw32"
  VDDM_FCM2NoComDTC_raw32_Inproc/1 -> UnitConverter336/1
  UnitConverter336/1 -> VOUTP_FCM2NoComDTC_raw32/1  "VOUTP_FCM2NoComDTC_raw32"
  VDDM_FCM2RCErrDTC_raw32/1 -> VDDM_FCM2RCErrDTC_raw32_Inproc/1  "VDDM_FCM2RCErrDTC_raw32"
  VDDM_FCM2RCErrDTC_raw32_Inproc/1 -> UnitConverter337/1
  UnitConverter337/1 -> VOUTP_FCM2RCErrDTC_raw32/1  "VOUTP_FCM2RCErrDTC_raw32"
  VDDM_FCM2CSErrDTC_raw32/1 -> VDDM_FCM2CSErrDTC_raw32_Inproc/1  "VDDM_FCM2CSErrDTC_raw32"
  VDDM_FCM2CSErrDTC_raw32_Inproc/1 -> UnitConverter338/1
  UnitConverter338/1 -> VOUTP_FCM2CSErrDTC_raw32/1  "VOUTP_FCM2CSErrDTC_raw32"
  VDDM_FCM3NoComDTC_raw32/1 -> VDDM_FCM3NoComDTC_raw32_Inproc/1  "VDDM_FCM3NoComDTC_raw32"
  VDDM_FCM3NoComDTC_raw32_Inproc/1 -> UnitConverter339/1
  UnitConverter339/1 -> VOUTP_FCM3NoComDTC_raw32/1  "VOUTP_FCM3NoComDTC_raw32"
  VDDM_FCM3RCErrDTC_raw32/1 -> VDDM_FCM3RCErrDTC_raw32_Inproc/1  "VDDM_FCM3RCErrDTC_raw32"
  VDDM_FCM3RCErrDTC_raw32_Inproc/1 -> UnitConverter340/1
  UnitConverter340/1 -> VOUTP_FCM3RCErrDTC_raw32/1  "VOUTP_FCM3RCErrDTC_raw32"
  VDDM_FCM3CSErrDTC_raw32/1 -> VDDM_FCM3CSErrDTC_raw32_Inproc/1  "VDDM_FCM3CSErrDTC_raw32"
  VDDM_FCM3CSErrDTC_raw32_Inproc/1 -> UnitConverter341/1
  UnitConverter341/1 -> VOUTP_FCM3CSErrDTC_raw32/1  "VOUTP_FCM3CSErrDTC_raw32"
  VDDM_FCM4NoComDTC_raw32/1 -> VDDM_FCM4NoComDTC_raw32_Inproc/1  "VDDM_FCM4NoComDTC_raw32"
  VDDM_FCM4NoComDTC_raw32_Inproc/1 -> UnitConverter342/1
  UnitConverter342/1 -> VOUTP_FCM4NoComDTC_raw32/1  "VOUTP_FCM4NoComDTC_raw32"
  VDDM_FCM4CSErrDTC_raw32/1 -> VDDM_FCM4CSErrDTC_raw32_Inproc/1  "VDDM_FCM4CSErrDTC_raw32"
  VDDM_FCM4CSErrDTC_raw32_Inproc/1 -> UnitConverter343/1
  UnitConverter343/1 -> VOUTP_FCM4CSErrDTC_raw32/1  "VOUTP_FCM4CSErrDTC_raw32"
  VDDM_FCM5NoComDTC_raw32/1 -> VDDM_FCM5NoComDTC_raw32_Inproc/1  "VDDM_FCM5NoComDTC_raw32"
  VDDM_FCM5NoComDTC_raw32_Inproc/1 -> UnitConverter344/1
  UnitConverter344/1 -> VOUTP_FCM5NoComDTC_raw32/1  "VOUTP_FCM5NoComDTC_raw32"
  VDDM_FCM5CSErrDTC_raw32/1 -> VDDM_FCM5CSErrDTC_raw32_Inproc/1  "VDDM_FCM5CSErrDTC_raw32"
  VDDM_FCM5CSErrDTC_raw32_Inproc/1 -> UnitConverter345/1
  UnitConverter345/1 -> VOUTP_FCM5CSErrDTC_raw32/1  "VOUTP_FCM5CSErrDTC_raw32"
  VDDM_ZoneSCPNoComDTC_raw32/1 -> VDDM_ZoneSCPNoComDTC_raw32_Inproc/1  "VDDM_ZoneSCPNoComDTC_raw32"
  VDDM_ZoneSCPNoComDTC_raw32_Inproc/1 -> UnitConverter346/1
  UnitConverter346/1 -> VOUTP_ZoneSCPNoComDTC_raw32/1  "VOUTP_ZoneSCPNoComDTC_raw32"
  VDDM_BMSSigErrDetDTC_raw32/1 -> VDDM_BMSSigErrDetDTC_raw32_Inproc/1  "VDDM_BMSSigErrDetDTC_raw32"
  VDDM_BMSSigErrDetDTC_raw32_Inproc/1 -> UnitConverter347/1
  UnitConverter347/1 -> VOUTP_BMSSigErrDetDTC_raw32/1  "VOUTP_BMSSigErrDetDTC_raw32"
  VDDM_FCMACCSigErrDetDTC_raw32/1 -> VDDM_FCMACCSigErrDetDTC_raw32_Inproc/1  "VDDM_FCMACCSigErrDetDTC_raw32"
  VDDM_FCMACCSigErrDetDTC_raw32_Inproc/1 -> UnitConverter348/1
  UnitConverter348/1 -> VOUTP_FCMACCSigErrDetDTC_raw32/1  "VOUTP_FCMACCSigErrDetDTC_raw32"
  VDDM_FrMCUSigErrDetDTC_raw32/1 -> VDDM_FrMCUSigErrDetDTC_raw32_Inproc/1  "VDDM_FrMCUSigErrDetDTC_raw32"
  VDDM_FrMCUSigErrDetDTC_raw32_Inproc/1 -> UnitConverter349/1
  UnitConverter349/1 -> VOUTP_FrMCUSigErrDetDTC_raw32/1  "VOUTP_FrMCUSigErrDetDTC_raw32"
  VDDM_RrMCUSigErrDetDTC_raw32/1 -> VDDM_RrMCUSigErrDetDTC_raw32_Inproc/1  "VDDM_RrMCUSigErrDetDTC_raw32"
  VDDM_RrMCUSigErrDetDTC_raw32_Inproc/1 -> UnitConverter350/1
  UnitConverter350/1 -> VOUTP_RrMCUSigErrDetDTC_raw32/1  "VOUTP_RrMCUSigErrDetDTC_raw32"
  VDDM_CCUSigErrDetDTC_raw32/1 -> VDDM_CCUSigErrDetDTC_raw32_Inproc/1  "VDDM_CCUSigErrDetDTC_raw32"
  VDDM_CCUSigErrDetDTC_raw32_Inproc/1 -> UnitConverter351/1
  UnitConverter351/1 -> VOUTP_CCUSigErrDetDTC_raw32/1  "VOUTP_CCUSigErrDetDTC_raw32"
  VDDM_ACCAccelCmdErrDetDTC_raw32/1 -> VDDM_ACCAccelCmdErrDetDTC_raw32_Inproc/1  "VDDM_ACCAccelCmdErrDetDTC_raw32"
  VDDM_ACCAccelCmdErrDetDTC_raw32_Inproc/1 -> UnitConverter352/1
  UnitConverter352/1 -> VOUTP_ACCAccelCmdErrDetDTC_raw32/1  "VOUTP_ACCAccelCmdErrDetDTC_raw32"
  VDDM_ACCMalfuncDetDTC_raw32/1 -> VDDM_ACCMalfuncDetDTC_raw32_Inproc/1  "VDDM_ACCMalfuncDetDTC_raw32"
  VDDM_ACCMalfuncDetDTC_raw32_Inproc/1 -> UnitConverter353/1
  UnitConverter353/1 -> VOUTP_ACCMalfuncDetDTC_raw32/1  "VOUTP_ACCMalfuncDetDTC_raw32"
  VDDM_CCMalfuncDetDTC_raw32/1 -> VDDM_CCMalfuncDetDTC_raw32_Inproc/1  "VDDM_CCMalfuncDetDTC_raw32"
  VDDM_CCMalfuncDetDTC_raw32_Inproc/1 -> UnitConverter354/1
  UnitConverter354/1 -> VOUTP_CCMalfuncDetDTC_raw32/1  "VOUTP_CCMalfuncDetDTC_raw32"
  VDDM_MSAMalfuncDetDTC_raw32/1 -> VDDM_MSAMalfuncDetDTC_raw32_Inproc/1  "VDDM_MSAMalfuncDetDTC_raw32"
  VDDM_MSAMalfuncDetDTC_raw32_Inproc/1 -> UnitConverter355/1
  UnitConverter355/1 -> VOUTP_MSAMalfuncDetDTC_raw32/1  "VOUTP_MSAMalfuncDetDTC_raw32"
  VDDM_ISAMalfuncDetDTC_raw32/1 -> VDDM_ISAMalfuncDetDTC_raw32_Inproc/1  "VDDM_ISAMalfuncDetDTC_raw32"
  VDDM_ISAMalfuncDetDTC_raw32_Inproc/1 -> UnitConverter356/1
  UnitConverter356/1 -> VOUTP_ISAMalfuncDetDTC_raw32/1  "VOUTP_ISAMalfuncDetDTC_raw32"
  VDDM_MCUF1RCErrDTC_raw32/1 -> VDDM_MCUF1RCErrDTC_raw32_Inproc/1  "VDDM_MCUF1RCErrDTC_raw32"
  VDDM_MCUF1RCErrDTC_raw32_Inproc/1 -> UnitConverter357/1
  UnitConverter357/1 -> VOUTP_MCUF1RCErrDTC_raw32/1  "VOUTP_MCUF1RCErrDTC_raw32"
  VDDM_MCUR1RCErrDTC_raw32/1 -> VDDM_MCUR1RCErrDTC_raw32_Inproc/1  "VDDM_MCUR1RCErrDTC_raw32"
  VDDM_MCUR1RCErrDTC_raw32_Inproc/1 -> UnitConverter358/1
  UnitConverter358/1 -> VOUTP_MCUR1RCErrDTC_raw32/1  "VOUTP_MCUR1RCErrDTC_raw32"
  VDDM_MCUF1CSErrDTC_raw32/1 -> VDDM_MCUF1CSErrDTC_raw32_Inproc/1  "VDDM_MCUF1CSErrDTC_raw32"
  VDDM_MCUF1CSErrDTC_raw32_Inproc/1 -> UnitConverter359/1
  UnitConverter359/1 -> VOUTP_MCUF1CSErrDTC_raw32/1  "VOUTP_MCUF1CSErrDTC_raw32"
  VDDM_MCUR1CSErrDTC_raw32/1 -> VDDM_MCUR1CSErrDTC_raw32_Inproc/1  "VDDM_MCUR1CSErrDTC_raw32"
  VDDM_MCUR1CSErrDTC_raw32_Inproc/1 -> UnitConverter360/1
  UnitConverter360/1 -> VOUTP_MCUR1CSErrDTC_raw32/1  "VOUTP_MCUR1CSErrDTC_raw32"
  VDDM_Shifter1RCErrDTC_raw32/1 -> VDDM_Shifter1RCErrDTC_raw32_Inproc/1  "VDDM_Shifter1RCErrDTC_raw32"
  VDDM_Shifter1RCErrDTC_raw32_Inproc/1 -> UnitConverter361/1
  UnitConverter361/1 -> VOUTP_Shifter1RCErrDTC_raw32/1  "VOUTP_Shifter1RCErrDTC_raw32"
  VDDM_Shifter1CSErrDTC_raw32/1 -> VDDM_Shifter1CSErrDTC_raw32_Inproc/1  "VDDM_Shifter1CSErrDTC_raw32"
  VDDM_Shifter1CSErrDTC_raw32_Inproc/1 -> UnitConverter362/1
  UnitConverter362/1 -> VOUTP_Shifter1CSErrDTC_raw32/1  "VOUTP_Shifter1CSErrDTC_raw32"
  VDDM_ESC7RCErrDTC_raw32/1 -> VDDM_ESC7RCErrDTC_raw32_Inproc/1  "VDDM_ESC7RCErrDTC_raw32"
  VDDM_ESC7RCErrDTC_raw32_Inproc/1 -> UnitConverter363/1
  UnitConverter363/1 -> VOUTP_ESC7RCErrDTC_raw32/1  "VOUTP_ESC7RCErrDTC_raw32"
  VDDM_ESC7CSErrDTC_raw32/1 -> VDDM_ESC7CSErrDTC_raw32_Inproc/1  "VDDM_ESC7CSErrDTC_raw32"
  VDDM_ESC7CSErrDTC_raw32_Inproc/1 -> UnitConverter364/1
  UnitConverter364/1 -> VOUTP_ESC7CSErrDTC_raw32/1  "VOUTP_ESC7CSErrDTC_raw32"
  VDDM_ESC1RCErrDTC_raw32/1 -> VDDM_ESC1RCErrDTC_raw32_Inproc/1  "VDDM_ESC1RCErrDTC_raw32"
  VDDM_ESC1RCErrDTC_raw32_Inproc/1 -> UnitConverter365/1
  UnitConverter365/1 -> VOUTP_ESC1RCErrDTC_raw32/1  "VOUTP_ESC1RCErrDTC_raw32"
  VDDM_ESC1CSErrDTC_raw32/1 -> VDDM_ESC1CSErrDTC_raw32_Inproc/1  "VDDM_ESC1CSErrDTC_raw32"
  VDDM_ESC1CSErrDTC_raw32_Inproc/1 -> UnitConverter366/1
  UnitConverter366/1 -> VOUTP_ESC1CSErrDTC_raw32/1  "VOUTP_ESC1CSErrDTC_raw32"
  VDDM_ESC5RCErrDTC_raw32/1 -> VDDM_ESC5RCErrDTC_raw32_Inproc/1  "VDDM_ESC5RCErrDTC_raw32"
  VDDM_ESC5RCErrDTC_raw32_Inproc/1 -> UnitConverter367/1
  UnitConverter367/1 -> VOUTP_ESC5RCErrDTC_raw32/1  "VOUTP_ESC5RCErrDTC_raw32"
  VDDM_ESC5CSErrDTC_raw32/1 -> VDDM_ESC5CSErrDTC_raw32_Inproc/1  "VDDM_ESC5CSErrDTC_raw32"
  VDDM_ESC5CSErrDTC_raw32_Inproc/1 -> UnitConverter368/1
  UnitConverter368/1 -> VOUTP_ESC5CSErrDTC_raw32/1  "VOUTP_ESC5CSErrDTC_raw32"
  VDDM_FrMCUTqErrDTC_raw32/1 -> VDDM_FrMCUTqErrDTC_raw32_Inproc/1  "VDDM_FrMCUTqErrDTC_raw32"
  VDDM_FrMCUTqErrDTC_raw32_Inproc/1 -> UnitConverter369/1
  UnitConverter369/1 -> VOUTP_FrMCUTqErrDTC_raw32/1  "VOUTP_FrMCUTqErrDTC_raw32"
  VDDM_RrMCUTqErrDTC_raw32/1 -> VDDM_RrMCUTqErrDTC_raw32_Inproc/1  "VDDM_RrMCUTqErrDTC_raw32"
  VDDM_RrMCUTqErrDTC_raw32_Inproc/1 -> UnitConverter370/1
  UnitConverter370/1 -> VOUTP_RrMCUTqErrDTC_raw32/1  "VOUTP_RrMCUTqErrDTC_raw32"
  VDDM_LFBatwarnDTC_raw32/1 -> VDDM_LFBatwarnDTC_raw32_Inproc/1  "VDDM_LFBatwarnDTC_raw32"
  VDDM_LFBatwarnDTC_raw32_Inproc/1 -> UnitConverter371/1
  UnitConverter371/1 -> VOUTP_LFBatwarnDTC_raw32/1  "VOUTP_LFBatwarnDTC_raw32"
  VDDM_RFBatwarnDTC_raw32/1 -> VDDM_RFBatwarnDTC_raw32_Inproc/1  "VDDM_RFBatwarnDTC_raw32"
  VDDM_RFBatwarnDTC_raw32_Inproc/1 -> UnitConverter372/1
  UnitConverter372/1 -> VOUTP_RFBatwarnDTC_raw32/1  "VOUTP_RFBatwarnDTC_raw32"
  VDDM_LRBatwarnDTC_raw32/1 -> VDDM_LRBatwarnDTC_raw32_Inproc/1  "VDDM_LRBatwarnDTC_raw32"
  VDDM_LRBatwarnDTC_raw32_Inproc/1 -> UnitConverter373/1
  UnitConverter373/1 -> VOUTP_LRBatwarnDTC_raw32/1  "VOUTP_LRBatwarnDTC_raw32"
  VDDM_RRBatwarnDTC_raw32/1 -> VDDM_RRBatwarnDTC_raw32_Inproc/1  "VDDM_RRBatwarnDTC_raw32"
  VDDM_RRBatwarnDTC_raw32_Inproc/1 -> UnitConverter374/1
  UnitConverter374/1 -> VOUTP_RRBatwarnDTC_raw32/1  "VOUTP_RRBatwarnDTC_raw32"
  VDDM_LFPressIndiDTC_raw32/1 -> VDDM_LFPressIndiDTC_raw32_Inproc/1  "VDDM_LFPressIndiDTC_raw32"
  VDDM_LFPressIndiDTC_raw32_Inproc/1 -> UnitConverter375/1
  UnitConverter375/1 -> VOUTP_LFPressIndiDTC_raw32/1  "VOUTP_LFPressIndiDTC_raw32"
  VDDM_RFPressIndiDTC_raw32/1 -> VDDM_RFPressIndiDTC_raw32_Inproc/1  "VDDM_RFPressIndiDTC_raw32"
  VDDM_RFPressIndiDTC_raw32_Inproc/1 -> UnitConverter376/1
  UnitConverter376/1 -> VOUTP_RFPressIndiDTC_raw32/1  "VOUTP_RFPressIndiDTC_raw32"
  VDDM_LRPressIndiDTC_raw32/1 -> VDDM_LRPressIndiDTC_raw32_Inproc/1  "VDDM_LRPressIndiDTC_raw32"
  VDDM_LRPressIndiDTC_raw32_Inproc/1 -> UnitConverter377/1
  UnitConverter377/1 -> VOUTP_LRPressIndiDTC_raw32/1  "VOUTP_LRPressIndiDTC_raw32"
  VDDM_RRPressIndiDTC_raw32/1 -> VDDM_RRPressIndiDTC_raw32_Inproc/1  "VDDM_RRPressIndiDTC_raw32"
  VDDM_RRPressIndiDTC_raw32_Inproc/1 -> UnitConverter378/1
  UnitConverter378/1 -> VOUTP_RRPressIndiDTC_raw32/1  "VOUTP_RRPressIndiDTC_raw32"
  VDDM_LFWheelTmpHighDTC_raw32/1 -> VDDM_LFWheelTmpHighDTC_raw32_Inproc/1  "VDDM_LFWheelTmpHighDTC_raw32"
  VDDM_LFWheelTmpHighDTC_raw32_Inproc/1 -> UnitConverter379/1
  UnitConverter379/1 -> VOUTP_LFWheelTmpHighDTC_raw32/1  "VOUTP_LFWheelTmpHighDTC_raw32"
  VDDM_RFWheelTmpHighDTC_raw32/1 -> VDDM_RFWheelTmpHighDTC_raw32_Inproc/1  "VDDM_RFWheelTmpHighDTC_raw32"
  VDDM_RFWheelTmpHighDTC_raw32_Inproc/1 -> UnitConverter380/1
  UnitConverter380/1 -> VOUTP_RFWheelTmpHighDTC_raw32/1  "VOUTP_RFWheelTmpHighDTC_raw32"
  VDDM_LRWheelTmpHighDTC_raw32/1 -> VDDM_LRWheelTmpHighDTC_raw32_Inproc/1  "VDDM_LRWheelTmpHighDTC_raw32"
  VDDM_LRWheelTmpHighDTC_raw32_Inproc/1 -> UnitConverter381/1
  UnitConverter381/1 -> VOUTP_LRWheelTmpHighDTC_raw32/1  "VOUTP_LRWheelTmpHighDTC_raw32"
  VDDM_RRWheelTmpHighDTC_raw32/1 -> VDDM_RRWheelTmpHighDTC_raw32_Inproc/1  "VDDM_RRWheelTmpHighDTC_raw32"
  VDDM_RRWheelTmpHighDTC_raw32_Inproc/1 -> UnitConverter382/1
  UnitConverter382/1 -> VOUTP_RRWheelTmpHighDTC_raw32/1  "VOUTP_RRWheelTmpHighDTC_raw32"
  VDDM_LFSensorFailDTC_raw32/1 -> VDDM_LFSensorFailDTC_raw32_Inproc/1  "VDDM_LFSensorFailDTC_raw32"
  VDDM_LFSensorFailDTC_raw32_Inproc/1 -> UnitConverter383/1
  UnitConverter383/1 -> VOUTP_LFSensorFailDTC_raw32/1  "VOUTP_LFSensorFailDTC_raw32"
  VDDM_RFSensorFailDTC_raw32/1 -> VDDM_RFSensorFailDTC_raw32_Inproc/1  "VDDM_RFSensorFailDTC_raw32"
  VDDM_RFSensorFailDTC_raw32_Inproc/1 -> UnitConverter384/1
  UnitConverter384/1 -> VOUTP_RFSensorFailDTC_raw32/1  "VOUTP_RFSensorFailDTC_raw32"
  VDDM_LRSensorFailDTC_raw32/1 -> VDDM_LRSensorFailDTC_raw32_Inproc/1  "VDDM_LRSensorFailDTC_raw32"
  VDDM_LRSensorFailDTC_raw32_Inproc/1 -> UnitConverter385/1
  UnitConverter385/1 -> VOUTP_LRSensorFailDTC_raw32/1  "VOUTP_LRSensorFailDTC_raw32"
  VDDM_RRSensorFailDTC_raw32/1 -> VDDM_RRSensorFailDTC_raw32_Inproc/1  "VDDM_RRSensorFailDTC_raw32"
  VDDM_RRSensorFailDTC_raw32_Inproc/1 -> UnitConverter386/1
  UnitConverter386/1 -> VOUTP_RRSensorFailDTC_raw32/1  "VOUTP_RRSensorFailDTC_raw32"
  VDDM_C1EPAS2LCDTC_raw32/1 -> VDDM_C1EPAS2LCDTC_raw32_Inproc/1  "VDDM_C1EPAS2LCDTC_raw32"
  VDDM_C1EPAS2LCDTC_raw32_Inproc/1 -> UnitConverter387/1
  UnitConverter387/1 -> VOUTP_C1EPAS2LCDTC_raw32/1  "VOUTP_C1EPAS2LCDTC_raw32"
  VDDM_5vAPS1PwrErrDTC_raw32/1 -> VDDM_5vAPS1PwrErrDTC_raw32_Inproc/1  "VDDM_5vAPS1PwrErrDTC_raw32"
  VDDM_5vAPS1PwrErrDTC_raw32_Inproc/1 -> UnitConverter388/1
  UnitConverter388/1 -> VOUTP_5vAPS1PwrErrDTC_raw32/1  "VOUTP_5vAPS1PwrErrDTC_raw32"
  VDDM_5vAPS2PwrErrDTC_raw32/1 -> VDDM_5vAPS2PwrErrDTC_raw32_Inproc/1  "VDDM_5vAPS2PwrErrDTC_raw32"
  VDDM_5vAPS2PwrErrDTC_raw32_Inproc/1 -> UnitConverter389/1
  UnitConverter389/1 -> VOUTP_5vAPS2PwrErrDTC_raw32/1  "VOUTP_5vAPS2PwrErrDTC_raw32"
  VDDM_EPBLockTODTC_raw32/1 -> VDDM_EPBLockTODTC_raw32_Inproc/1  "VDDM_EPBLockTODTC_raw32"
  VDDM_EPBLockTODTC_raw32_Inproc/1 -> UnitConverter390/1
  UnitConverter390/1 -> VOUTP_EPBLockTODTC_raw32/1  "VOUTP_EPBLockTODTC_raw32"
  VDDM_EPBUnlockTODTC_raw32/1 -> VDDM_EPBUnlockTODTC_raw32_Inproc/1  "VDDM_EPBUnlockTODTC_raw32"
  VDDM_EPBUnlockTODTC_raw32_Inproc/1 -> UnitConverter391/1
  UnitConverter391/1 -> VOUTP_EPBUnlockTODTC_raw32/1  "VOUTP_EPBUnlockTODTC_raw32"
  VDDM_THCMAPTCWarning_raw32/1 -> VDDM_THCMAPTCWarning_raw32_Inproc/1  "VDDM_THCMAPTCWarning_raw32"
  VDDM_THCMAPTCWarning_raw32_Inproc/1 -> UnitConverter392/1
  UnitConverter392/1 -> VOUTP_THCMAPTCWarning_raw32/1  "VOUTP_THCMAPTCWarning_raw32"
  VDDM_LimpHomeActTmp_flg/1 -> VDDM_LimpHomeActTmp_flg_Inproc/1  "VDDM_LimpHomeActTmp_flg"
  VDDM_LimpHomeActTmp_flg_Inproc/1 -> UnitConverter393/1
  UnitConverter393/1 -> VOUTP_LimpHomeActTmp_flg/1  "VOUTP_LimpHomeActTmp_flg"
  VDDM_EDriveSysErr_VCUErrTmp_flg/1 -> VDDM_EDriveSysErr_VCUErrTmp_flg_Inproc/1  "VDDM_EDriveSysErr_VCUErrTmp_flg"
  VDDM_EDriveSysErr_VCUErrTmp_flg_Inproc/1 -> UnitConverter394/1
  UnitConverter394/1 -> VOUTP_EDriveSysErr_VCUErrTmp_flg/1  "VOUTP_EDriveSysErr_VCUErrTmp_flg"
  VDHP_ActAPSPosn_pct/1 -> VDHP_ActAPSPosn_pct_Inproc/1  "VDHP_ActAPSPosn_pct"
  VDHP_ActAPSPosn_pct_Inproc/1 -> UnitConverter395/1
  UnitConverter395/1 -> VOUTP_ActAPSPosn_pct/1  "VOUTP_ActAPSPosn_pct"
  VDHP_EAPS1MIN_pct/1 -> VDHP_EAPS1MIN_pct_Inproc/1  "VDHP_EAPS1MIN_pct"
  VDHP_EAPS1MIN_pct_Inproc/1 -> UnitConverter396/1
  UnitConverter396/1 -> VOUTP_EAPS1MIN_pct/1  "VOUTP_EAPS1MIN_pct"
  VDHP_EAPS2MIN_pct/1 -> VDHP_EAPS2MIN_pct_Inproc/1  "VDHP_EAPS2MIN_pct"
  VDHP_EAPS2MIN_pct_Inproc/1 -> UnitConverter397/1
  UnitConverter397/1 -> VOUTP_EAPS2MIN_pct/1  "VOUTP_EAPS2MIN_pct"
  VDKC_DKCTimeSN_cnt/1 -> VDKC_DKCTimeSN_cnt_Inproc/1  "VDKC_DKCTimeSN_cnt"
  VDKC_DKCTimeSN_cnt_Inproc/1 -> UnitConverter398/1
  UnitConverter398/1 -> VOUTP_DKCTimeSN_cnt/1  "VOUTP_DKCTimeSN_cnt"
  VDKC_DKCAuthSta_enum/1 -> VDKC_DKCAuthSta_enum_Inproc/1  "VDKC_DKCAuthSta_enum"
  VDKC_DKCAuthSta_enum_Inproc/1 -> UnitConverter399/1
  UnitConverter399/1 -> VOUTP_DKCAuthSta_enum/1  "VOUTP_DKCAuthSta_enum"
  VNMM_AllCANTxReq_flg/1 -> VNMM_AllCANTxReq_flg_Inproc/1  "VNMM_AllCANTxReq_flg"
  VNMM_AllCANTxReq_flg_Inproc/1 -> UnitConverter400/1
  UnitConverter400/1 -> VOUTP_AllCANTxReq_flg/1  "VOUTP_AllCANTxReq_flg"
  VNMM_NMmTxReq_flg/1 -> VNMM_NMmTxReq_flg_Inproc/1  "VNMM_NMmTxReq_flg"
  VNMM_NMmTxReq_flg_Inproc/1 -> UnitConverter401/1
  UnitConverter401/1 -> VOUTP_NMmTxReq_flg/1  "VOUTP_NMmTxReq_flg"
  VNMM_Awake_enum/1 -> VNMM_Awake_enum_Inproc/1  "VNMM_Awake_enum"
  VNMM_Awake_enum_Inproc/1 -> UnitConverter402/1
  UnitConverter402/1 -> VOUTP_Awake_enum/1  "VOUTP_Awake_enum"
  VNMM_CSB_flg/1 -> VNMM_CSB_flg_Inproc/1  "VNMM_CSB_flg"
  VNMM_CSB_flg_Inproc/1 -> UnitConverter403/1
  UnitConverter403/1 -> VOUTP_CSB_flg/1  "VOUTP_CSB_flg"
  VNMM_ErrorState_enum/1 -> VNMM_ErrorState_enum_Inproc/1  "VNMM_ErrorState_enum"
  VNMM_ErrorState_enum_Inproc/1 -> UnitConverter404/1
  UnitConverter404/1 -> VOUTP_ErrorState_enum/1  "VOUTP_ErrorState_enum"
  VNMM_NodeID_enum/1 -> VNMM_NodeID_enum_Inproc/1  "VNMM_NodeID_enum"
  VNMM_NodeID_enum_Inproc/1 -> UnitConverter405/1
  UnitConverter405/1 -> VOUTP_NodeID_enum/1  "VOUTP_NodeID_enum"
  VNMM_PNI_flg/1 -> VNMM_PNI_flg_Inproc/1  "VNMM_PNI_flg"
  VNMM_PNI_flg_Inproc/1 -> UnitConverter406/1
  UnitConverter406/1 -> VOUTP_PNI_flg/1  "VOUTP_PNI_flg"
  VNMM_RptMsgReq_flg/1 -> VNMM_RptMsgReq_flg_Inproc/1  "VNMM_RptMsgReq_flg"
  VNMM_RptMsgReq_flg_Inproc/1 -> UnitConverter407/1
  UnitConverter407/1 -> VOUTP_RptMsgReq_flg/1  "VOUTP_RptMsgReq_flg"
  VNMM_WakeUp_enum/1 -> VNMM_WakeUp_enum_Inproc/1  "VNMM_WakeUp_enum"
  VNMM_WakeUp_enum_Inproc/1 -> UnitConverter408/1
  UnitConverter408/1 -> VOUTP_WakeUp_enum/1  "VOUTP_WakeUp_enum"
  VNMM_ActiveWU_flg/1 -> VNMM_ActiveWU_flg_Inproc/1  "VNMM_ActiveWU_flg"
  VNMM_ActiveWU_flg_Inproc/1 -> UnitConverter409/1
  UnitConverter409/1 -> VOUTP_ActiveWU_flg/1  "VOUTP_ActiveWU_flg"
  VNMM_SysNMmSta_enum/1 -> VNMM_SysNMmSta_enum_Inproc/1  "VNMM_SysNMmSta_enum"
  VNMM_SysNMmSta_enum_Inproc/1 -> UnitConverter410/1
  UnitConverter410/1 -> VOUTP_SysNMmSta_enum/1  "VOUTP_SysNMmSta_enum"
  VNMM_NetworkReq_flg/1 -> VNMM_NetworkReq_flg_Inproc/1  "VNMM_NetworkReq_flg"
  VNMM_NetworkReq_flg_Inproc/1 -> UnitConverter411/1
  UnitConverter411/1 -> VOUTP_NetworkReq_flg/1  "VOUTP_NetworkReq_flg"
  VPMM_PowerUpState_enum/1 -> VPMM_PowerUpState_enum_Inproc/1  "VPMM_PowerUpState_enum"
  VPMM_PowerUpState_enum_Inproc/1 -> UnitConverter412/1
  UnitConverter412/1 -> VOUTP_PowerUpState_enum/1  "VOUTP_PowerUpState_enum"
  VPMM_PowerDownState_enum/1 -> VPMM_PowerDownState_enum_Inproc/1  "VPMM_PowerDownState_enum"
  VPMM_PowerDownState_enum_Inproc/1 -> UnitConverter413/1
  UnitConverter413/1 -> VOUTP_PowerDownState_enum/1  "VOUTP_PowerDownState_enum"
  VPMM_PowerUpFault_enum/1 -> VPMM_PowerUpFault_enum_Inproc/1  "VPMM_PowerUpFault_enum"
  VPMM_PowerUpFault_enum_Inproc/1 -> UnitConverter414/1
  UnitConverter414/1 -> VOUTP_PowerUpFault_enum/1  "VOUTP_PowerUpFault_enum"
  VPMM_PowerDownFault_enum/1 -> VPMM_PowerDownFault_enum_Inproc/1  "VPMM_PowerDownFault_enum"
  VPMM_PowerDownFault_enum_Inproc/1 -> UnitConverter415/1
  UnitConverter415/1 -> VOUTP_PowerDownFault_enum/1  "VOUTP_PowerDownFault_enum"
  VPMM_ActiveDischargeReq_flg/1 -> VPMM_ActiveDischargeReq_flg_Inproc/1  "VPMM_ActiveDischargeReq_flg"
  VPMM_ActiveDischargeReq_flg_Inproc/1 -> UnitConverter416/1
  UnitConverter416/1 -> VOUTP_ActiveDischargeReq_flg/1  "VOUTP_ActiveDischargeReq_flg"
  VPMM_DCDCEnaReq_flg/1 -> VPMM_DCDCEnaReq_flg_Inproc/1  "VPMM_DCDCEnaReq_flg"
  VPMM_DCDCEnaReq_flg_Inproc/1 -> UnitConverter417/1
  UnitConverter417/1 -> VOUTP_DCDCEnaReq_flg/1  "VOUTP_DCDCEnaReq_flg"
  VPMM_DCDCVoltSetpoint_V/1 -> VPMM_DCDCVoltSetpoint_V_Inproc/1  "VPMM_DCDCVoltSetpoint_V"
  VPMM_DCDCVoltSetpoint_V_Inproc/1 -> UnitConverter418/1
  UnitConverter418/1 -> VOUTP_DCDCVoltSetpoint_V/1  "VOUTP_DCDCVoltSetpoint_V"
  VPMM_HVBatCnctReq_flg/1 -> VPMM_HVBatCnctReq_flg_Inproc/1  "VPMM_HVBatCnctReq_flg"
  VPMM_HVBatCnctReq_flg_Inproc/1 -> UnitConverter419/1
  UnitConverter419/1 -> VOUTP_HVBatCnctReq_flg/1  "VOUTP_HVBatCnctReq_flg"
  VPMM_HVSysReadyToCharge_enum/1 -> VPMM_HVSysReadyToCharge_enum_Inproc/1  "VPMM_HVSysReadyToCharge_enum"
  VPMM_HVSysReadyToCharge_enum_Inproc/1 -> UnitConverter420/1
  UnitConverter420/1 -> VOUTP_HVSysReadyToCharge_enum/1  "VOUTP_HVSysReadyToCharge_enum"
  VPMM_PowerSta_enum/1 -> VPMM_PowerSta_enum_Inproc/1  "VPMM_PowerSta_enum"
  VPMM_PowerSta_enum_Inproc/1 -> UnitConverter421/1
  UnitConverter421/1 -> VOUTP_PowerSta_enum/1  "VOUTP_PowerSta_enum"
  VPMM_LVPwrSta_flg/1 -> VPMM_LVPwrSta_flg_Inproc/1  "VPMM_LVPwrSta_flg"
  VPMM_LVPwrSta_flg_Inproc/1 -> UnitConverter422/1
  UnitConverter422/1 -> VOUTP_LVPwrSta_flg/1  "VOUTP_LVPwrSta_flg"
  VPMM_HVPwrSta_flg/1 -> VPMM_HVPwrSta_flg_Inproc/1  "VPMM_HVPwrSta_flg"
  VPMM_HVPwrSta_flg_Inproc/1 -> UnitConverter423/1
  UnitConverter423/1 -> VOUTP_HVPwrSta_flg/1  "VOUTP_HVPwrSta_flg"
  VPMM_SysPowerMode_enum/1 -> VPMM_SysPowerMode_enum_Inproc/1  "VPMM_SysPowerMode_enum"
  VPMM_SysPowerMode_enum_Inproc/1 -> UnitConverter424/1
  UnitConverter424/1 -> VOUTP_SysPowerMode_enum/1  "VOUTP_SysPowerMode_enum"
  VPMM_FrMCUEnaReq_flg/1 -> VPMM_FrMCUEnaReq_flg_Inproc/1  "VPMM_FrMCUEnaReq_flg"
  VPMM_FrMCUEnaReq_flg_Inproc/1 -> UnitConverter425/1
  UnitConverter425/1 -> VOUTP_FrMCUEnaReq_flg/1  "VOUTP_FrMCUEnaReq_flg"
  VPMM_RrMCUEnaReq_flg/1 -> VPMM_RrMCUEnaReq_flg_Inproc/1  "VPMM_RrMCUEnaReq_flg"
  VPMM_RrMCUEnaReq_flg_Inproc/1 -> UnitConverter426/1
  UnitConverter426/1 -> VOUTP_RrMCUEnaReq_flg/1  "VOUTP_RrMCUEnaReq_flg"
  VPMM_DrivetrainSelect_enum/1 -> VPMM_DrivetrainSelect_enum_Inproc/1  "VPMM_DrivetrainSelect_enum"
  VPMM_DrivetrainSelect_enum_Inproc/1 -> UnitConverter427/1
  UnitConverter427/1 -> VOUTP_DrivetrainSelect_enum/1  "VOUTP_DrivetrainSelect_enum"
  VPMM_DrSeatSta_enum/1 -> VPMM_DrSeatSta_enum_Inproc/1  "VPMM_DrSeatSta_enum"
  VPMM_DrSeatSta_enum_Inproc/1 -> UnitConverter428/1
  UnitConverter428/1 -> VOUTP_DrSeatSta_enum/1  "VOUTP_DrSeatSta_enum"
  VPMM_PwrStaSelect_enum/1 -> VPMM_PwrStaSelect_enum_Inproc/1  "VPMM_PwrStaSelect_enum"
  VPMM_PwrStaSelect_enum_Inproc/1 -> UnitConverter429/1
  UnitConverter429/1 -> VOUTP_PwrStaSelect_enum/1  "VOUTP_PwrStaSelect_enum"
  VPMM_PwrStaConstraint_enum/1 -> VPMM_PwrStaConstraint_enum_Inproc/1  "VPMM_PwrStaConstraint_enum"
  VPMM_PwrStaConstraint_enum_Inproc/1 -> UnitConverter430/1
  UnitConverter430/1 -> VOUTP_PwrStaConstraint_enum/1  "VOUTP_PwrStaConstraint_enum"
  VPMM_TCountSta_enum/1 -> VPMM_TCountSta_enum_Inproc/1  "VPMM_TCountSta_enum"
  VPMM_TCountSta_enum_Inproc/1 -> UnitConverter431/1
  UnitConverter431/1 -> VOUTP_TCountSta_enum/1  "VOUTP_TCountSta_enum"
  VPMM_PwrUpReq_enum/1 -> VPMM_PwrUpReq_enum_Inproc/1  "VPMM_PwrUpReq_enum"
  VPMM_PwrUpReq_enum_Inproc/1 -> UnitConverter432/1
  UnitConverter432/1 -> VOUTP_PwrUpReq_enum/1  "VOUTP_PwrUpReq_enum"
  VPMM_PwrDownReq_enum/1 -> VPMM_PwrDownReq_enum_Inproc/1  "VPMM_PwrDownReq_enum"
  VPMM_PwrDownReq_enum_Inproc/1 -> UnitConverter433/1
  UnitConverter433/1 -> VOUTP_PwrDownReq_enum/1  "VOUTP_PwrDownReq_enum"
  VPMM_LowSOCWarn_enum/1 -> VPMM_LowSOCWarn_enum_Inproc/1  "VPMM_LowSOCWarn_enum"
  VPMM_LowSOCWarn_enum_Inproc/1 -> UnitConverter434/1
  UnitConverter434/1 -> VOUTP_LowSOCWarn_enum/1  "VOUTP_LowSOCWarn_enum"
  VPMM_ReVehThdChkSta_enum/1 -> VPMM_ReVehThdChkSta_enum_Inproc/1  "VPMM_ReVehThdChkSta_enum"
  VPMM_ReVehThdChkSta_enum_Inproc/1 -> UnitConverter435/1
  UnitConverter435/1 -> VOUTP_ReVehThdChkSta_enum/1  "VOUTP_ReVehThdChkSta_enum"
  VPMM_LVSysErrPwrOutErr_flg/1 -> VPMM_LVSysErrPwrOutErr_flg_Inproc/1  "VPMM_LVSysErrPwrOutErr_flg"
  VPMM_LVSysErrPwrOutErr_flg_Inproc/1 -> UnitConverter436/1
  UnitConverter436/1 -> VOUTP_LVSysErrPwrOutErr_flg/1  "VOUTP_LVSysErrPwrOutErr_flg"
  VPMM_EvccAplusPwrUpReq_flg/1 -> VPMM_EvccAplusPwrUpReq_flg_Inproc/1  "VPMM_EvccAplusPwrUpReq_flg"
  VPMM_EvccAplusPwrUpReq_flg_Inproc/1 -> UnitConverter437/1
  UnitConverter437/1 -> VOUTP_EvccAplusPwrUpReq_flg/1  "VOUTP_EvccAplusPwrUpReq_flg"
  VPMM_PwrStaONTOPopReq_flg/1 -> VPMM_PwrStaONTOPopReq_flg_Inproc/1  "VPMM_PwrStaONTOPopReq_flg"
  VPMM_PwrStaONTOPopReq_flg_Inproc/1 -> UnitConverter438/1
  UnitConverter438/1 -> VOUTP_PwrStaONTOPopReq_flg/1  "VOUTP_PwrStaONTOPopReq_flg"
  VPMM_IVIPwrStaONTOPopT_s/1 -> VPMM_IVIPwrStaONTOPopT_s_Inproc/1  "VPMM_IVIPwrStaONTOPopT_s"
  VPMM_IVIPwrStaONTOPopT_s_Inproc/1 -> UnitConverter439/1
  UnitConverter439/1 -> VOUTP_IVIPwrStaONTOPopT_s/1  "VOUTP_IVIPwrStaONTOPopT_s"
  VPMM_LVChrgHoldTtimer_s/1 -> VPMM_LVChrgHoldTtimer_s_Inproc/1  "VPMM_LVChrgHoldTtimer_s"
  VPMM_LVChrgHoldTtimer_s_Inproc/1 -> UnitConverter440/1
  UnitConverter440/1 -> VOUTP_LVChrgHoldTtimer_s/1  "VOUTP_LVChrgHoldTtimer_s"
  VPMM_LVBattChrgTimeCnt_s/1 -> VPMM_LVBattChrgTimeCnt_s_Inproc/1  "VPMM_LVBattChrgTimeCnt_s"
  VPMM_LVBattChrgTimeCnt_s_Inproc/1 -> UnitConverter441/1
  UnitConverter441/1 -> VOUTP_LVBattChrgTimeCnt_s/1  "VOUTP_LVBattChrgTimeCnt_s"
  VPMM_SilentChkAllowSleep_flg/1 -> VPMM_SilentChkAllowSleep_flg_Inproc/1  "VPMM_SilentChkAllowSleep_flg"
  VPMM_SilentChkAllowSleep_flg_Inproc/1 -> UnitConverter442/1
  UnitConverter442/1 -> VOUTP_SilentChkAllowSleep_flg/1  "VOUTP_SilentChkAllowSleep_flg"
  VPMM_TimerAllowSleep_flg/1 -> VPMM_TimerAllowSleep_flg_Inproc/1  "VPMM_TimerAllowSleep_flg"
  VPMM_TimerAllowSleep_flg_Inproc/1 -> UnitConverter443/1
  UnitConverter443/1 -> VOUTP_TimerAllowSleep_flg/1  "VOUTP_TimerAllowSleep_flg"
  VPMM_FDADC12VDetAvg_mV/1 -> VPMM_FDADC12VDetAvg_mV_Inproc/1  "VPMM_FDADC12VDetAvg_mV"
  VPMM_FDADC12VDetAvg_mV_Inproc/1 -> UnitConverter444/1
  UnitConverter444/1 -> VOUTP_FDADC12VDetAvg_mV/1  "VOUTP_FDADC12VDetAvg_mV"
  VPMM_PMMAllowECUSleep_flg/1 -> VPMM_PMMAllowECUSleep_flg_Inproc/1  "VPMM_PMMAllowECUSleep_flg"
  VPMM_PMMAllowECUSleep_flg_Inproc/1 -> UnitConverter445/1
  UnitConverter445/1 -> VOUTP_PMMAllowECUSleep_flg/1  "VOUTP_PMMAllowECUSleep_flg"
  VPMM_LVSilentChrgSta_enum/1 -> VPMM_LVSilentChrgSta_enum_Inproc/1  "VPMM_LVSilentChrgSta_enum"
  VPMM_LVSilentChrgSta_enum_Inproc/1 -> UnitConverter446/1
  UnitConverter446/1 -> VOUTP_LVSilentChrgSta_enum/1  "VOUTP_LVSilentChrgSta_enum"
  VPMM_LVSilentChrgReq_flg/1 -> VPMM_LVSilentChrgReq_flg_Inproc/1  "VPMM_LVSilentChrgReq_flg"
  VPMM_LVSilentChrgReq_flg_Inproc/1 -> UnitConverter447/1
  UnitConverter447/1 -> VOUTP_LVSilentChrgReq_flg/1  "VOUTP_LVSilentChrgReq_flg"
  VPMM_LVSilentChrgLv_enum/1 -> VPMM_LVSilentChrgLv_enum_Inproc/1  "VPMM_LVSilentChrgLv_enum"
  VPMM_LVSilentChrgLv_enum_Inproc/1 -> UnitConverter448/1
  UnitConverter448/1 -> VOUTP_LVSilentChrgLv_enum/1  "VOUTP_LVSilentChrgLv_enum"
  VPMM_CtrlFrPwrStbA1P_flg/1 -> VPMM_CtrlFrPwrStbA1P_flg_Inproc/1  "VPMM_CtrlFrPwrStbA1P_flg"
  VPMM_CtrlFrPwrStbA1P_flg_Inproc/1 -> UnitConverter449/1
  UnitConverter449/1 -> VOUTP_CtrlFrPwrStbA1P_flg/1  "VOUTP_CtrlFrPwrStbA1P_flg"
  VPMM_CtrlFrRC1_flg/1 -> VPMM_CtrlFrRC1_flg_Inproc/1  "VPMM_CtrlFrRC1_flg"
  VPMM_CtrlFrRC1_flg_Inproc/1 -> UnitConverter450/1
  UnitConverter450/1 -> VOUTP_CtrlFrRC1_flg/1  "VOUTP_CtrlFrRC1_flg"
  VPMM_CtrlFrBMSCCUCIR_flg/1 -> VPMM_CtrlFrBMSCCUCIR_flg_Inproc/1  "VPMM_CtrlFrBMSCCUCIR_flg"
  VPMM_CtrlFrBMSCCUCIR_flg_Inproc/1 -> UnitConverter451/1
  UnitConverter451/1 -> VOUTP_CtrlFrBMSCCUCIR_flg/1  "VOUTP_CtrlFrBMSCCUCIR_flg"
  VPMM_CtrlFrEDUINVERTER_flg/1 -> VPMM_CtrlFrEDUINVERTER_flg_Inproc/1  "VPMM_CtrlFrEDUINVERTER_flg"
  VPMM_CtrlFrEDUINVERTER_flg_Inproc/1 -> UnitConverter452/1
  UnitConverter452/1 -> VOUTP_CtrlFrEDUINVERTER_flg/1  "VOUTP_CtrlFrEDUINVERTER_flg"
  VPMM_HWResetSta_enum/1 -> VPMM_HWResetSta_enum_Inproc/1  "VPMM_HWResetSta_enum"
  VPMM_HWResetSta_enum_Inproc/1 -> UnitConverter453/1
  UnitConverter453/1 -> VOUTP_HWResetSta_enum/1  "VOUTP_HWResetSta_enum"
  VPMM_CtrlDrPwrStbA2_flg/1 -> VPMM_CtrlDrPwrStbA2_flg_Inproc/1  "VPMM_CtrlDrPwrStbA2_flg"
  VPMM_CtrlDrPwrStbA2_flg_Inproc/1 -> UnitConverter454/1
  UnitConverter454/1 -> VOUTP_CtrlDrPwrStbA2_flg/1  "VOUTP_CtrlDrPwrStbA2_flg"
  VPMM_PwrStaTOSta_enum/1 -> VPMM_PwrStaTOSta_enum_Inproc/1  "VPMM_PwrStaTOSta_enum"
  VPMM_PwrStaTOSta_enum_Inproc/1 -> UnitConverter455/1
  UnitConverter455/1 -> VOUTP_PwrStaTOSta_enum/1  "VOUTP_PwrStaTOSta_enum"
  VPMM_Sched_ChgTOSta_enum/1 -> VPMM_Sched_ChgTOSta_enum_Inproc/1  "VPMM_Sched_ChgTOSta_enum"
  VPMM_Sched_ChgTOSta_enum_Inproc/1 -> UnitConverter456/1
  UnitConverter456/1 -> VOUTP_Sched_ChgTOSta_enum/1  "VOUTP_Sched_ChgTOSta_enum"
  VPMM_PwrReq_OTA_enum/1 -> VPMM_PwrReq_OTA_enum_Inproc/1  "VPMM_PwrReq_OTA_enum"
  VPMM_PwrReq_OTA_enum_Inproc/1 -> UnitConverter457/1
  UnitConverter457/1 -> VOUTP_PwrReq_OTA_enum/1  "VOUTP_PwrReq_OTA_enum"
  VPMM_OTAPwrReqOFFChkSta_enum/1 -> VPMM_OTAPwrReqOFFChkSta_enum_Inproc/1  "VPMM_OTAPwrReqOFFChkSta_enum"
  VPMM_OTAPwrReqOFFChkSta_enum_Inproc/1 -> UnitConverter458/1
  UnitConverter458/1 -> VOUTP_OTAPwrReqOFFChkSta_enum/1  "VOUTP_OTAPwrReqOFFChkSta_enum"
  VPMM_OTAPwrReqStdChkSta_enum/1 -> VPMM_OTAPwrReqStdChkSta_enum_Inproc/1  "VPMM_OTAPwrReqStdChkSta_enum"
  VPMM_OTAPwrReqStdChkSta_enum_Inproc/1 -> UnitConverter459/1
  UnitConverter459/1 -> VOUTP_OTAPwrReqStdChkSta_enum/1  "VOUTP_OTAPwrReqStdChkSta_enum"
  VSYS_HWVer1_cnt/1 -> VSYS_HWVer1_cnt_Inproc/1  "VSYS_HWVer1_cnt"
  VSYS_HWVer1_cnt_Inproc/1 -> UnitConverter460/1
  UnitConverter460/1 -> VOUTP_HWVer1_cnt/1  "VOUTP_HWVer1_cnt"
  VSYS_HWVer2_cnt/1 -> VSYS_HWVer2_cnt_Inproc/1  "VSYS_HWVer2_cnt"
  VSYS_HWVer2_cnt_Inproc/1 -> UnitConverter461/1
  UnitConverter461/1 -> VOUTP_HWVer2_cnt/1  "VOUTP_HWVer2_cnt"
  VSYS_HWVer3_cnt/1 -> VSYS_HWVer3_cnt_Inproc/1  "VSYS_HWVer3_cnt"
  VSYS_HWVer3_cnt_Inproc/1 -> UnitConverter462/1
  UnitConverter462/1 -> VOUTP_HWVer3_cnt/1  "VOUTP_HWVer3_cnt"
  VSYS_CarModel1_cnt/1 -> VSYS_CarModel1_cnt_Inproc/1  "VSYS_CarModel1_cnt"
  VSYS_CarModel1_cnt_Inproc/1 -> UnitConverter463/1
  UnitConverter463/1 -> VOUTP_CarModel1_cnt/1  "VOUTP_CarModel1_cnt"
  VSYS_CarModel2_cnt/1 -> VSYS_CarModel2_cnt_Inproc/1  "VSYS_CarModel2_cnt"
  VSYS_CarModel2_cnt_Inproc/1 -> UnitConverter464/1
  UnitConverter464/1 -> VOUTP_CarModel2_cnt/1  "VOUTP_CarModel2_cnt"
  VSYS_CarModel3_cnt/1 -> VSYS_CarModel3_cnt_Inproc/1  "VSYS_CarModel3_cnt"
  VSYS_CarModel3_cnt_Inproc/1 -> UnitConverter465/1
  UnitConverter465/1 -> VOUTP_CarModel3_cnt/1  "VOUTP_CarModel3_cnt"
  VSYS_ECU1_cnt/1 -> VSYS_ECU1_cnt_Inproc/1  "VSYS_ECU1_cnt"
  VSYS_ECU1_cnt_Inproc/1 -> UnitConverter466/1
  UnitConverter466/1 -> VOUTP_ECU1_cnt/1  "VOUTP_ECU1_cnt"
  VSYS_ECU2_cnt/1 -> VSYS_ECU2_cnt_Inproc/1  "VSYS_ECU2_cnt"
  VSYS_ECU2_cnt_Inproc/1 -> UnitConverter467/1
  UnitConverter467/1 -> VOUTP_ECU2_cnt/1  "VOUTP_ECU2_cnt"
  VSYS_Major1_cnt/1 -> VSYS_Major1_cnt_Inproc/1  "VSYS_Major1_cnt"
  VSYS_Major1_cnt_Inproc/1 -> UnitConverter468/1
  UnitConverter468/1 -> VOUTP_Major1_cnt/1  "VOUTP_Major1_cnt"
  VSYS_Major2_cnt/1 -> VSYS_Major2_cnt_Inproc/1  "VSYS_Major2_cnt"
  VSYS_Major2_cnt_Inproc/1 -> UnitConverter469/1
  UnitConverter469/1 -> VOUTP_Major2_cnt/1  "VOUTP_Major2_cnt"
  VSYS_Minor1_cnt/1 -> VSYS_Minor1_cnt_Inproc/1  "VSYS_Minor1_cnt"
  VSYS_Minor1_cnt_Inproc/1 -> UnitConverter470/1
  UnitConverter470/1 -> VOUTP_Minor1_cnt/1  "VOUTP_Minor1_cnt"
  VSYS_Minor2_cnt/1 -> VSYS_Minor2_cnt_Inproc/1  "VSYS_Minor2_cnt"
  VSYS_Minor2_cnt_Inproc/1 -> UnitConverter471/1
  UnitConverter471/1 -> VOUTP_Minor2_cnt/1  "VOUTP_Minor2_cnt"
  VSYS_Patch1_cnt/1 -> VSYS_Patch1_cnt_Inproc/1  "VSYS_Patch1_cnt"
  VSYS_Patch1_cnt_Inproc/1 -> UnitConverter472/1
  UnitConverter472/1 -> VOUTP_Patch1_cnt/1  "VOUTP_Patch1_cnt"
  VSYS_Patch2_cnt/1 -> VSYS_Patch2_cnt_Inproc/1  "VSYS_Patch2_cnt"
  VSYS_Patch2_cnt_Inproc/1 -> UnitConverter473/1
  UnitConverter473/1 -> VOUTP_Patch2_cnt/1  "VOUTP_Patch2_cnt"
  VSYS_Country1_cnt/1 -> VSYS_Country1_cnt_Inproc/1  "VSYS_Country1_cnt"
  VSYS_Country1_cnt_Inproc/1 -> UnitConverter474/1
  UnitConverter474/1 -> VOUTP_Country1_cnt/1  "VOUTP_Country1_cnt"
  VSYS_Country2_cnt/1 -> VSYS_Country2_cnt_Inproc/1  "VSYS_Country2_cnt"
  VSYS_Country2_cnt_Inproc/1 -> UnitConverter475/1
  UnitConverter475/1 -> VOUTP_Country2_cnt/1  "VOUTP_Country2_cnt"
  VSYS_Variation_cnt/1 -> VSYS_Variation_cnt_Inproc/1  "VSYS_Variation_cnt"
  VSYS_Variation_cnt_Inproc/1 -> UnitConverter476/1
  UnitConverter476/1 -> VOUTP_Variation_cnt/1  "VOUTP_Variation_cnt"
  VSYS_Dash1_cnt/1 -> VSYS_Dash1_cnt_Inproc/1  "VSYS_Dash1_cnt"
  VSYS_Dash1_cnt_Inproc/1 -> UnitConverter477/1
  UnitConverter477/1 -> VOUTP_Dash1_cnt/1  "VOUTP_Dash1_cnt"
  VSYS_Change1_cnt/1 -> VSYS_Change1_cnt_Inproc/1  "VSYS_Change1_cnt"
  VSYS_Change1_cnt_Inproc/1 -> UnitConverter478/1
  UnitConverter478/1 -> VOUTP_Change1_cnt/1  "VOUTP_Change1_cnt"
  VSYS_Change2_cnt/1 -> VSYS_Change2_cnt_Inproc/1  "VSYS_Change2_cnt"
  VSYS_Change2_cnt_Inproc/1 -> UnitConverter479/1
  UnitConverter479/1 -> VOUTP_Change2_cnt/1  "VOUTP_Change2_cnt"
  VSYS_Dash2_cnt/1 -> VSYS_Dash2_cnt_Inproc/1  "VSYS_Dash2_cnt"
  VSYS_Dash2_cnt_Inproc/1 -> UnitConverter480/1
  UnitConverter480/1 -> VOUTP_Dash2_cnt/1  "VOUTP_Dash2_cnt"
  VSYS_SHA1_cnt/1 -> VSYS_SHA1_cnt_Inproc/1  "VSYS_SHA1_cnt"
  VSYS_SHA1_cnt_Inproc/1 -> UnitConverter481/1
  UnitConverter481/1 -> VOUTP_SHA1_cnt/1  "VOUTP_SHA1_cnt"
  VSYS_SHA2_cnt/1 -> VSYS_SHA2_cnt_Inproc/1  "VSYS_SHA2_cnt"
  VSYS_SHA2_cnt_Inproc/1 -> UnitConverter482/1
  UnitConverter482/1 -> VOUTP_SHA2_cnt/1  "VOUTP_SHA2_cnt"
  VSYS_SHA3_cnt/1 -> VSYS_SHA3_cnt_Inproc/1  "VSYS_SHA3_cnt"
  VSYS_SHA3_cnt_Inproc/1 -> UnitConverter483/1
  UnitConverter483/1 -> VOUTP_SHA3_cnt/1  "VOUTP_SHA3_cnt"
  VSYS_SHA4_cnt/1 -> VSYS_SHA4_cnt_Inproc/1  "VSYS_SHA4_cnt"
  VSYS_SHA4_cnt_Inproc/1 -> UnitConverter484/1
  UnitConverter484/1 -> VOUTP_SHA4_cnt/1  "VOUTP_SHA4_cnt"
  VSYS_SHA5_cnt/1 -> VSYS_SHA5_cnt_Inproc/1  "VSYS_SHA5_cnt"
  VSYS_SHA5_cnt_Inproc/1 -> UnitConverter485/1
  UnitConverter485/1 -> VOUTP_SHA5_cnt/1  "VOUTP_SHA5_cnt"
  VSYS_SHA6_cnt/1 -> VSYS_SHA6_cnt_Inproc/1  "VSYS_SHA6_cnt"
  VSYS_SHA6_cnt_Inproc/1 -> UnitConverter486/1
  UnitConverter486/1 -> VOUTP_SHA6_cnt/1  "VOUTP_SHA6_cnt"
  VSYS_SHA7_cnt/1 -> VSYS_SHA7_cnt_Inproc/1  "VSYS_SHA7_cnt"
  VSYS_SHA7_cnt_Inproc/1 -> UnitConverter487/1
  UnitConverter487/1 -> VOUTP_SHA7_cnt/1  "VOUTP_SHA7_cnt"
  VSYS_SHA8_cnt/1 -> VSYS_SHA8_cnt_Inproc/1  "VSYS_SHA8_cnt"
  VSYS_SHA8_cnt_Inproc/1 -> UnitConverter488/1
  UnitConverter488/1 -> VOUTP_SHA8_cnt/1  "VOUTP_SHA8_cnt"
  VSYS_NvWriteReqRisingEdge_flg/1 -> VSYS_NvWriteReqRisingEdge_flg_Inproc/1  "VSYS_NvWriteReqRisingEdge_flg"
  VSYS_NvWriteReqRisingEdge_flg_Inproc/1 -> UnitConverter489/1
  UnitConverter489/1 -> VOUTP_NvWriteReqRisingEdge_flg/1  "VOUTP_NvWriteReqRisingEdge_flg"
  VSYS_FdcSlpReqRisingEdge_flg/1 -> VSYS_FdcSlpReqRisingEdge_flg_Inproc/1  "VSYS_FdcSlpReqRisingEdge_flg"
  VSYS_FdcSlpReqRisingEdge_flg_Inproc/1 -> UnitConverter490/1
  UnitConverter490/1 -> VOUTP_FdcSlpReqRisingEdge_flg/1  "VOUTP_FdcSlpReqRisingEdge_flg"
  VSYS_FdcSlpTime_sec/1 -> VSYS_FdcSlpTime_sec_Inproc/1  "VSYS_FdcSlpTime_sec"
  VSYS_FdcSlpTime_sec_Inproc/1 -> UnitConverter491/1
  UnitConverter491/1 -> VOUTP_FdcSlpTime_sec/1  "VOUTP_FdcSlpTime_sec"
  VSYS_PmicBootReason_enum/1 -> VSYS_PmicBootReason_enum_Inproc/1  "VSYS_PmicBootReason_enum"
  VSYS_PmicBootReason_enum_Inproc/1 -> UnitConverter492/1
  UnitConverter492/1 -> VOUTP_PmicBootReason_enum/1  "VOUTP_PmicBootReason_enum"
  VSYS_WisrBootReason_raw32/1 -> VSYS_WisrBootReason_raw32_Inproc/1  "VSYS_WisrBootReason_raw32"
  VSYS_WisrBootReason_raw32_Inproc/1 -> UnitConverter493/1
  UnitConverter493/1 -> VOUTP_WisrBootReason_raw32/1  "VOUTP_WisrBootReason_raw32"
  VSYS_AcoreRebootCmdACK_flg/1 -> VSYS_AcoreRebootCmdACK_flg_Inproc/1  "VSYS_AcoreRebootCmdACK_flg"
  VSYS_AcoreRebootCmdACK_flg_Inproc/1 -> UnitConverter494/1
  UnitConverter494/1 -> VOUTP_AcoreRebootCmdACK_flg/1  "VOUTP_AcoreRebootCmdACK_flg"
  VSYS_CurrentNmState_enum/1 -> VSYS_CurrentNmState_enum_Inproc/1  "VSYS_CurrentNmState_enum"
  VSYS_CurrentNmState_enum_Inproc/1 -> UnitConverter495/1
  UnitConverter495/1 -> VOUTP_CurrentNmState_enum/1  "VOUTP_CurrentNmState_enum"
  VTHC_FDCompCmd_rpm/1 -> VTHC_FDCompCmd_rpm_Inproc/1  "VTHC_FDCompCmd_rpm"
  VTHC_FDCompCmd_rpm_Inproc/1 -> UnitConverter496/1
  UnitConverter496/1 -> VOUTP_FDCompCmd_rpm/1  "VOUTP_FDCompCmd_rpm"
  VTHC_FDSOV1Cmd_flg/1 -> VTHC_FDSOV1Cmd_flg_Inproc/1  "VTHC_FDSOV1Cmd_flg"
  VTHC_FDSOV1Cmd_flg_Inproc/1 -> UnitConverter497/1
  UnitConverter497/1 -> VOUTP_FDSOV1Cmd_flg/1  "VOUTP_FDSOV1Cmd_flg"
  VTHC_FDSOV2Cmd_flg/1 -> VTHC_FDSOV2Cmd_flg_Inproc/1  "VTHC_FDSOV2Cmd_flg"
  VTHC_FDSOV2Cmd_flg_Inproc/1 -> UnitConverter498/1
  UnitConverter498/1 -> VOUTP_FDSOV2Cmd_flg/1  "VOUTP_FDSOV2Cmd_flg"
  VTHC_FDSOV3Cmd_flg/1 -> VTHC_FDSOV3Cmd_flg_Inproc/1  "VTHC_FDSOV3Cmd_flg"
  VTHC_FDSOV3Cmd_flg_Inproc/1 -> UnitConverter499/1
  UnitConverter499/1 -> VOUTP_FDSOV3Cmd_flg/1  "VOUTP_FDSOV3Cmd_flg"
  VTHC_FDEXV1Cmd_step/1 -> VTHC_FDEXV1Cmd_step_Inproc/1  "VTHC_FDEXV1Cmd_step"
  VTHC_FDEXV1Cmd_step_Inproc/1 -> UnitConverter500/1
  UnitConverter500/1 -> VOUTP_FDEXV1Cmd_step/1  "VOUTP_FDEXV1Cmd_step"
  VTHC_FDEXV2Cmd_step/1 -> VTHC_FDEXV2Cmd_step_Inproc/1  "VTHC_FDEXV2Cmd_step"
  VTHC_FDEXV2Cmd_step_Inproc/1 -> UnitConverter501/1
  UnitConverter501/1 -> VOUTP_FDEXV2Cmd_step/1  "VOUTP_FDEXV2Cmd_step"
  VTHC_FDSOTXVCmd_flg/1 -> VTHC_FDSOTXVCmd_flg_Inproc/1  "VTHC_FDSOTXVCmd_flg"
  VTHC_FDSOTXVCmd_flg_Inproc/1 -> UnitConverter502/1
  UnitConverter502/1 -> VOUTP_FDSOTXVCmd_flg/1  "VOUTP_FDSOTXVCmd_flg"
  VTHC_FDFWVCmd_flg/1 -> VTHC_FDFWVCmd_flg_Inproc/1  "VTHC_FDFWVCmd_flg"
  VTHC_FDFWVCmd_flg_Inproc/1 -> UnitConverter503/1
  UnitConverter503/1 -> VOUTP_FDFWVCmd_flg/1  "VOUTP_FDFWVCmd_flg"
  VTHC_FDTWVCmd_pct/1 -> VTHC_FDTWVCmd_pct_Inproc/1  "VTHC_FDTWVCmd_pct"
  VTHC_FDTWVCmd_pct_Inproc/1 -> UnitConverter504/1
  UnitConverter504/1 -> VOUTP_FDTWVCmd_pct/1  "VOUTP_FDTWVCmd_pct"
  VTHC_FDFrWPTCHeatPwrCmd_W/1 -> VTHC_FDFrWPTCHeatPwrCmd_W_Inproc/1  "VTHC_FDFrWPTCHeatPwrCmd_W"
  VTHC_FDFrWPTCHeatPwrCmd_W_Inproc/1 -> UnitConverter505/1
  UnitConverter505/1 -> VOUTP_FDFrWPTCHeatPwrCmd_W/1  "VOUTP_FDFrWPTCHeatPwrCmd_W"
  VTHC_CoolgFanActDuty_pct/1 -> VTHC_CoolgFanActDuty_pct_Inproc/1  "VTHC_CoolgFanActDuty_pct"
  VTHC_CoolgFanActDuty_pct_Inproc/1 -> UnitConverter506/1
  UnitConverter506/1 -> VOUTP_CoolgFanActDuty_pct/1  "VOUTP_CoolgFanActDuty_pct"
  VTHC_FDAGSCmd_enum/1 -> VTHC_FDAGSCmd_enum_Inproc/1  "VTHC_FDAGSCmd_enum"
  VTHC_FDAGSCmd_enum_Inproc/1 -> UnitConverter507/1
  UnitConverter507/1 -> VOUTP_FDAGSCmd_enum/1  "VOUTP_FDAGSCmd_enum"
  VTHC_FDEWP1Cmd_enum/1 -> VTHC_FDEWP1Cmd_enum_Inproc/1  "VTHC_FDEWP1Cmd_enum"
  VTHC_FDEWP1Cmd_enum_Inproc/1 -> UnitConverter508/1
  UnitConverter508/1 -> VOUTP_FDEWP1Cmd_enum/1  "VOUTP_FDEWP1Cmd_enum"
  VTHC_FDEWP2Cmd_enum/1 -> VTHC_FDEWP2Cmd_enum_Inproc/1  "VTHC_FDEWP2Cmd_enum"
  VTHC_FDEWP2Cmd_enum_Inproc/1 -> UnitConverter509/1
  UnitConverter509/1 -> VOUTP_FDEWP2Cmd_enum/1  "VOUTP_FDEWP2Cmd_enum"
  VTHC_FDEWP3Cmd_enum/1 -> VTHC_FDEWP3Cmd_enum_Inproc/1  "VTHC_FDEWP3Cmd_enum"
  VTHC_FDEWP3Cmd_enum_Inproc/1 -> UnitConverter510/1
  UnitConverter510/1 -> VOUTP_FDEWP3Cmd_enum/1  "VOUTP_FDEWP3Cmd_enum"
  VTHC_FDFrLeAPTCHeatPwrCmd_W/1 -> VTHC_FDFrLeAPTCHeatPwrCmd_W_Inproc/1  "VTHC_FDFrLeAPTCHeatPwrCmd_W"
  VTHC_FDFrLeAPTCHeatPwrCmd_W_Inproc/1 -> UnitConverter511/1
  UnitConverter511/1 -> VOUTP_FDFrLeAPTCHeatPwrCmd_W/1  "VOUTP_FDFrLeAPTCHeatPwrCmd_W"
  VTHC_FDFrRiAPTCHeatPwrCmd_W/1 -> VTHC_FDFrRiAPTCHeatPwrCmd_W_Inproc/1  "VTHC_FDFrRiAPTCHeatPwrCmd_W"
  VTHC_FDFrRiAPTCHeatPwrCmd_W_Inproc/1 -> UnitConverter512/1
  UnitConverter512/1 -> VOUTP_FDFrRiAPTCHeatPwrCmd_W/1  "VOUTP_FDFrRiAPTCHeatPwrCmd_W"
  VTHC_FDRrAPTCHeatPwrCmd_W/1 -> VTHC_FDRrAPTCHeatPwrCmd_W_Inproc/1  "VTHC_FDRrAPTCHeatPwrCmd_W"
  VTHC_FDRrAPTCHeatPwrCmd_W_Inproc/1 -> UnitConverter513/1
  UnitConverter513/1 -> VOUTP_FDRrAPTCHeatPwrCmd_W/1  "VOUTP_FDRrAPTCHeatPwrCmd_W"
  VTHC_FDBlowerCmd_pct/1 -> VTHC_FDBlowerCmd_pct_Inproc/1  "VTHC_FDBlowerCmd_pct"
  VTHC_FDBlowerCmd_pct_Inproc/1 -> UnitConverter514/1
  UnitConverter514/1 -> VOUTP_FDBlowerCmd_pct/1  "VOUTP_FDBlowerCmd_pct"
  VTHC_BatteryMode_enum/1 -> VTHC_BatteryMode_enum_Inproc/1  "VTHC_BatteryMode_enum"
  VTHC_BatteryMode_enum_Inproc/1 -> UnitConverter515/1
  UnitConverter515/1 -> VOUTP_BatteryMode_enum/1  "VOUTP_BatteryMode_enum"
  VTHC_EDriveMode_enum/1 -> VTHC_EDriveMode_enum_Inproc/1  "VTHC_EDriveMode_enum"
  VTHC_EDriveMode_enum_Inproc/1 -> UnitConverter516/1
  UnitConverter516/1 -> VOUTP_EDriveMode_enum/1  "VOUTP_EDriveMode_enum"
  VTHC_CabinMode_enum/1 -> VTHC_CabinMode_enum_Inproc/1  "VTHC_CabinMode_enum"
  VTHC_CabinMode_enum_Inproc/1 -> UnitConverter517/1
  UnitConverter517/1 -> VOUTP_CabinMode_enum/1  "VOUTP_CabinMode_enum"
  VTHC_CCUACLampSts_flg/1 -> VTHC_CCUACLampSts_flg_Inproc/1  "VTHC_CCUACLampSts_flg"
  VTHC_CCUACLampSts_flg_Inproc/1 -> UnitConverter518/1
  UnitConverter518/1 -> VOUTP_CCUACLampSts_flg/1  "VOUTP_CCUACLampSts_flg"
  VTHC_CCUAutoLampSts_flg/1 -> VTHC_CCUAutoLampSts_flg_Inproc/1  "VTHC_CCUAutoLampSts_flg"
  VTHC_CCUAutoLampSts_flg_Inproc/1 -> UnitConverter519/1
  UnitConverter519/1 -> VOUTP_CCUAutoLampSts_flg/1  "VOUTP_CCUAutoLampSts_flg"
  VTHC_CCUACMaxLampSts_flg/1 -> VTHC_CCUACMaxLampSts_flg_Inproc/1  "VTHC_CCUACMaxLampSts_flg"
  VTHC_CCUACMaxLampSts_flg_Inproc/1 -> UnitConverter520/1
  UnitConverter520/1 -> VOUTP_CCUACMaxLampSts_flg/1  "VOUTP_CCUACMaxLampSts_flg"
  VTHC_CCUSyncLampSts_flg/1 -> VTHC_CCUSyncLampSts_flg_Inproc/1  "VTHC_CCUSyncLampSts_flg"
  VTHC_CCUSyncLampSts_flg_Inproc/1 -> UnitConverter521/1
  UnitConverter521/1 -> VOUTP_CCUSyncLampSts_flg/1  "VOUTP_CCUSyncLampSts_flg"
  VTHC_sigAirIntenZon1St_enum/1 -> VTHC_sigAirIntenZon1St_enum_Inproc/1  "VTHC_sigAirIntenZon1St_enum"
  VTHC_sigAirIntenZon1St_enum_Inproc/1 -> UnitConverter522/1
  UnitConverter522/1 -> VOUTP_sigAirIntenZon1St_enum/1  "VOUTP_sigAirIntenZon1St_enum"
  VTHC_sigWindDirZon1St_enum/1 -> VTHC_sigWindDirZon1St_enum_Inproc/1  "VTHC_sigWindDirZon1St_enum"
  VTHC_sigWindDirZon1St_enum_Inproc/1 -> UnitConverter523/1
  UnitConverter523/1 -> VOUTP_sigWindDirZon1St_enum/1  "VOUTP_sigWindDirZon1St_enum"
  VTHC_sigRecircSt_flg/1 -> VTHC_sigRecircSt_flg_Inproc/1  "VTHC_sigRecircSt_flg"
  VTHC_sigRecircSt_flg_Inproc/1 -> UnitConverter524/1
  UnitConverter524/1 -> VOUTP_sigRecircSt_flg/1  "VOUTP_sigRecircSt_flg"
  VTHC_sigSetTempZon1St_C/1 -> VTHC_sigSetTempZon1St_C_Inproc/1  "VTHC_sigSetTempZon1St_C"
  VTHC_sigSetTempZon1St_C_Inproc/1 -> UnitConverter525/1
  UnitConverter525/1 -> VOUTP_sigSetTempZon1St_C/1  "VOUTP_sigSetTempZon1St_C"
  VTHC_sigSetTempZon2St_C/1 -> VTHC_sigSetTempZon2St_C_Inproc/1  "VTHC_sigSetTempZon2St_C"
  VTHC_sigSetTempZon2St_C_Inproc/1 -> UnitConverter526/1
  UnitConverter526/1 -> VOUTP_sigSetTempZon2St_C/1  "VOUTP_sigSetTempZon2St_C"
  VTHC_sigClntTHvBattOut_C/1 -> VTHC_sigClntTHvBattOut_C_Inproc/1  "VTHC_sigClntTHvBattOut_C"
  VTHC_sigClntTHvBattOut_C_Inproc/1 -> UnitConverter527/1
  UnitConverter527/1 -> VOUTP_sigClntTHvBattOut_C/1  "VOUTP_sigClntTHvBattOut_C"
  VTHC_sigCbnSolarLeft_W/1 -> VTHC_sigCbnSolarLeft_W_Inproc/1  "VTHC_sigCbnSolarLeft_W"
  VTHC_sigCbnSolarLeft_W_Inproc/1 -> UnitConverter528/1
  UnitConverter528/1 -> VOUTP_sigCbnSolarLeft_W/1  "VOUTP_sigCbnSolarLeft_W"
  VTHC_sigClntTHvBattIn_C/1 -> VTHC_sigClntTHvBattIn_C_Inproc/1  "VTHC_sigClntTHvBattIn_C"
  VTHC_sigClntTHvBattIn_C_Inproc/1 -> UnitConverter529/1
  UnitConverter529/1 -> VOUTP_sigClntTHvBattIn_C/1  "VOUTP_sigClntTHvBattIn_C"
  VTHC_sigCbnSolarRight_W/1 -> VTHC_sigCbnSolarRight_W_Inproc/1  "VTHC_sigCbnSolarRight_W"
  VTHC_sigCbnSolarRight_W_Inproc/1 -> UnitConverter530/1
  UnitConverter530/1 -> VOUTP_sigCbnSolarRight_W/1  "VOUTP_sigCbnSolarRight_W"
  VTHC_sigAmbAirT_C/1 -> VTHC_sigAmbAirT_C_Inproc/1  "VTHC_sigAmbAirT_C"
  VTHC_sigAmbAirT_C_Inproc/1 -> UnitConverter531/1
  UnitConverter531/1 -> VOUTP_sigAmbAirT_C/1  "VOUTP_sigAmbAirT_C"
  VTHC_sigCbnAirT_C/1 -> VTHC_sigCbnAirT_C_Inproc/1  "VTHC_sigCbnAirT_C"
  VTHC_sigCbnAirT_C_Inproc/1 -> UnitConverter532/1
  UnitConverter532/1 -> VOUTP_sigCbnAirT_C/1  "VOUTP_sigCbnAirT_C"
  VTHC_ACSubMode_enum/1 -> VTHC_ACSubMode_enum_Inproc/1  "VTHC_ACSubMode_enum"
  VTHC_ACSubMode_enum_Inproc/1 -> UnitConverter533/1
  UnitConverter533/1 -> VOUTP_ACSubMode_enum/1  "VOUTP_ACSubMode_enum"
  VTHC_FDRecyAutoCmd_enum/1 -> VTHC_FDRecyAutoCmd_enum_Inproc/1  "VTHC_FDRecyAutoCmd_enum"
  VTHC_FDRecyAutoCmd_enum_Inproc/1 -> UnitConverter534/1
  UnitConverter534/1 -> VOUTP_FDRecyAutoCmd_enum/1  "VOUTP_FDRecyAutoCmd_enum"
  VTHC_ACModeMem_enum/1 -> VTHC_ACModeMem_enum_Inproc/1  "VTHC_ACModeMem_enum"
  VTHC_ACModeMem_enum_Inproc/1 -> UnitConverter535/1
  UnitConverter535/1 -> VOUTP_ACModeMem_enum/1  "VOUTP_ACModeMem_enum"
  VTHC_Face_flg/1 -> VTHC_Face_flg_Inproc/1  "VTHC_Face_flg"
  VTHC_Face_flg_Inproc/1 -> UnitConverter536/1
  UnitConverter536/1 -> VOUTP_Face_flg/1  "VOUTP_Face_flg"
  VTHC_Foot_flg/1 -> VTHC_Foot_flg_Inproc/1  "VTHC_Foot_flg"
  VTHC_Foot_flg_Inproc/1 -> UnitConverter537/1
  UnitConverter537/1 -> VOUTP_Foot_flg/1  "VOUTP_Foot_flg"
  VTHC_Frost_flg/1 -> VTHC_Frost_flg_Inproc/1  "VTHC_Frost_flg"
  VTHC_Frost_flg_Inproc/1 -> UnitConverter538/1
  UnitConverter538/1 -> VOUTP_Frost_flg/1  "VOUTP_Frost_flg"
  VTHC_FaceM_flg/1 -> VTHC_FaceM_flg_Inproc/1  "VTHC_FaceM_flg"
  VTHC_FaceM_flg_Inproc/1 -> UnitConverter539/1
  UnitConverter539/1 -> VOUTP_FaceM_flg/1  "VOUTP_FaceM_flg"
  VTHC_FootM_flg/1 -> VTHC_FootM_flg_Inproc/1  "VTHC_FootM_flg"
  VTHC_FootM_flg_Inproc/1 -> UnitConverter540/1
  UnitConverter540/1 -> VOUTP_FootM_flg/1  "VOUTP_FootM_flg"
  VTHC_CCUSyncSts_flg/1 -> VTHC_CCUSyncSts_flg_Inproc/1  "VTHC_CCUSyncSts_flg"
  VTHC_CCUSyncSts_flg_Inproc/1 -> UnitConverter541/1
  UnitConverter541/1 -> VOUTP_CCUSyncSts_flg/1  "VOUTP_CCUSyncSts_flg"
  VTHC_ACForceOFF_flg/1 -> VTHC_ACForceOFF_flg_Inproc/1  "VTHC_ACForceOFF_flg"
  VTHC_ACForceOFF_flg_Inproc/1 -> UnitConverter542/1
  UnitConverter542/1 -> VOUTP_ACForceOFF_flg/1  "VOUTP_ACForceOFF_flg"
  VTHC_RecAutoFlg_flg/1 -> VTHC_RecAutoFlg_flg_Inproc/1  "VTHC_RecAutoFlg_flg"
  VTHC_RecAutoFlg_flg_Inproc/1 -> UnitConverter543/1
  UnitConverter543/1 -> VOUTP_RecAutoFlg_flg/1  "VOUTP_RecAutoFlg_flg"
  VTHC_AirIntenZone1M_enum/1 -> VTHC_AirIntenZone1M_enum_Inproc/1  "VTHC_AirIntenZone1M_enum"
  VTHC_AirIntenZone1M_enum_Inproc/1 -> UnitConverter544/1
  UnitConverter544/1 -> VOUTP_AirIntenZone1M_enum/1  "VOUTP_AirIntenZone1M_enum"
  VTHC_fdefog_flg/1 -> VTHC_fdefog_flg_Inproc/1  "VTHC_fdefog_flg"
  VTHC_fdefog_flg_Inproc/1 -> UnitConverter545/1
  UnitConverter545/1 -> VOUTP_fdefog_flg/1  "VOUTP_fdefog_flg"
  VTHC_sigSetTempZon2StM_C/1 -> VTHC_sigSetTempZon2StM_C_Inproc/1  "VTHC_sigSetTempZon2StM_C"
  VTHC_sigSetTempZon2StM_C_Inproc/1 -> UnitConverter546/1
  UnitConverter546/1 -> VOUTP_sigSetTempZon2StM_C/1  "VOUTP_sigSetTempZon2StM_C"
  VTHC_sigDfrstSt_flg/1 -> VTHC_sigDfrstSt_flg_Inproc/1  "VTHC_sigDfrstSt_flg"
  VTHC_sigDfrstSt_flg_Inproc/1 -> UnitConverter547/1
  UnitConverter547/1 -> VOUTP_sigDfrstSt_flg/1  "VOUTP_sigDfrstSt_flg"
  VTHC_FDCTHCAirIntZ3Sta_enum/1 -> VTHC_FDCTHCAirIntZ3Sta_enum_Inproc/1  "VTHC_FDCTHCAirIntZ3Sta_enum"
  VTHC_FDCTHCAirIntZ3Sta_enum_Inproc/1 -> UnitConverter548/1
  UnitConverter548/1 -> VOUTP_FDCTHCAirIntZ3Sta_enum/1  "VOUTP_FDCTHCAirIntZ3Sta_enum"
  VTHC_FDCTHCDrEVentModeSta_enum/1 -> VTHC_FDCTHCDrEVentModeSta_enum_Inproc/1  "VTHC_FDCTHCDrEVentModeSta_enum"
  VTHC_FDCTHCDrEVentModeSta_enum_Inproc/1 -> UnitConverter549/1
  UnitConverter549/1 -> VOUTP_FDCTHCDrEVentModeSta_enum/1  "VOUTP_FDCTHCDrEVentModeSta_enum"
  VTHC_FDCTHCPsEVentModeSta_enum/1 -> VTHC_FDCTHCPsEVentModeSta_enum_Inproc/1  "VTHC_FDCTHCPsEVentModeSta_enum"
  VTHC_FDCTHCPsEVentModeSta_enum_Inproc/1 -> UnitConverter550/1
  UnitConverter550/1 -> VOUTP_FDCTHCPsEVentModeSta_enum/1  "VOUTP_FDCTHCPsEVentModeSta_enum"
  VTHC_FDCTHCDrEVentZSta_enum/1 -> VTHC_FDCTHCDrEVentZSta_enum_Inproc/1  "VTHC_FDCTHCDrEVentZSta_enum"
  VTHC_FDCTHCDrEVentZSta_enum_Inproc/1 -> UnitConverter551/1
  UnitConverter551/1 -> VOUTP_FDCTHCDrEVentZSta_enum/1  "VOUTP_FDCTHCDrEVentZSta_enum"
  VTHC_FDCTHCCLEVentZSta_enum/1 -> VTHC_FDCTHCCLEVentZSta_enum_Inproc/1  "VTHC_FDCTHCCLEVentZSta_enum"
  VTHC_FDCTHCCLEVentZSta_enum_Inproc/1 -> UnitConverter552/1
  UnitConverter552/1 -> VOUTP_FDCTHCCLEVentZSta_enum/1  "VOUTP_FDCTHCCLEVentZSta_enum"
  VTHC_FDCTHCPsEVentZSta_enum/1 -> VTHC_FDCTHCPsEVentZSta_enum_Inproc/1  "VTHC_FDCTHCPsEVentZSta_enum"
  VTHC_FDCTHCPsEVentZSta_enum_Inproc/1 -> UnitConverter553/1
  UnitConverter553/1 -> VOUTP_FDCTHCPsEVentZSta_enum/1  "VOUTP_FDCTHCPsEVentZSta_enum"
  VTHC_FDCTHCCREVentZSta_enum/1 -> VTHC_FDCTHCCREVentZSta_enum_Inproc/1  "VTHC_FDCTHCCREVentZSta_enum"
  VTHC_FDCTHCCREVentZSta_enum_Inproc/1 -> UnitConverter554/1
  UnitConverter554/1 -> VOUTP_FDCTHCCREVentZSta_enum/1  "VOUTP_FDCTHCCREVentZSta_enum"
  VTHC_FDCTHCDrEVentYSta_enum/1 -> VTHC_FDCTHCDrEVentYSta_enum_Inproc/1  "VTHC_FDCTHCDrEVentYSta_enum"
  VTHC_FDCTHCDrEVentYSta_enum_Inproc/1 -> UnitConverter555/1
  UnitConverter555/1 -> VOUTP_FDCTHCDrEVentYSta_enum/1  "VOUTP_FDCTHCDrEVentYSta_enum"
  VTHC_FDCTHCDrVentENSta_flg/1 -> VTHC_FDCTHCDrVentENSta_flg_Inproc/1  "VTHC_FDCTHCDrVentENSta_flg"
  VTHC_FDCTHCDrVentENSta_flg_Inproc/1 -> UnitConverter556/1
  UnitConverter556/1 -> VOUTP_FDCTHCDrVentENSta_flg/1  "VOUTP_FDCTHCDrVentENSta_flg"
  VTHC_FDCTHCCLEVentYSta_enum/1 -> VTHC_FDCTHCCLEVentYSta_enum_Inproc/1  "VTHC_FDCTHCCLEVentYSta_enum"
  VTHC_FDCTHCCLEVentYSta_enum_Inproc/1 -> UnitConverter557/1
  UnitConverter557/1 -> VOUTP_FDCTHCCLEVentYSta_enum/1  "VOUTP_FDCTHCCLEVentYSta_enum"
  VTHC_FDCTHCCLVentENSta_flg/1 -> VTHC_FDCTHCCLVentENSta_flg_Inproc/1  "VTHC_FDCTHCCLVentENSta_flg"
  VTHC_FDCTHCCLVentENSta_flg_Inproc/1 -> UnitConverter558/1
  UnitConverter558/1 -> VOUTP_FDCTHCCLVentENSta_flg/1  "VOUTP_FDCTHCCLVentENSta_flg"
  VTHC_FDCTHCPsEVentYSta_enum/1 -> VTHC_FDCTHCPsEVentYSta_enum_Inproc/1  "VTHC_FDCTHCPsEVentYSta_enum"
  VTHC_FDCTHCPsEVentYSta_enum_Inproc/1 -> UnitConverter559/1
  UnitConverter559/1 -> VOUTP_FDCTHCPsEVentYSta_enum/1  "VOUTP_FDCTHCPsEVentYSta_enum"
  VTHC_FDCTHCPsVentENSta_flg/1 -> VTHC_FDCTHCPsVentENSta_flg_Inproc/1  "VTHC_FDCTHCPsVentENSta_flg"
  VTHC_FDCTHCPsVentENSta_flg_Inproc/1 -> UnitConverter560/1
  UnitConverter560/1 -> VOUTP_FDCTHCPsVentENSta_flg/1  "VOUTP_FDCTHCPsVentENSta_flg"
  VTHC_FDCTHCCREVentYSta_enum/1 -> VTHC_FDCTHCCREVentYSta_enum_Inproc/1  "VTHC_FDCTHCCREVentYSta_enum"
  VTHC_FDCTHCCREVentYSta_enum_Inproc/1 -> UnitConverter561/1
  UnitConverter561/1 -> VOUTP_FDCTHCCREVentYSta_enum/1  "VOUTP_FDCTHCCREVentYSta_enum"
  VTHC_FDCTHCCRVentENSta_flg/1 -> VTHC_FDCTHCCRVentENSta_flg_Inproc/1  "VTHC_FDCTHCCRVentENSta_flg"
  VTHC_FDCTHCCRVentENSta_flg_Inproc/1 -> UnitConverter562/1
  UnitConverter562/1 -> VOUTP_FDCTHCCRVentENSta_flg/1  "VOUTP_FDCTHCCRVentENSta_flg"
  VTHC_FDCTHCMAPTCForceOFFSta_flg/1 -> VTHC_FDCTHCMAPTCForceOFFSta_flg_Inproc/1  "VTHC_FDCTHCMAPTCForceOFFSta_flg"
  VTHC_FDCTHCMAPTCForceOFFSta_flg_Inproc/1 -> UnitConverter563/1
  UnitConverter563/1 -> VOUTP_FDCTHCMAPTCForceOFFSta_flg/1  "VOUTP_FDCTHCMAPTCForceOFFSta_flg"
  VTHC_DrVentEN_flg/1 -> VTHC_DrVentEN_flg_Inproc/1  "VTHC_DrVentEN_flg"
  VTHC_DrVentEN_flg_Inproc/1 -> UnitConverter564/1
  UnitConverter564/1 -> VOUTP_DrVentEN_flg/1  "VOUTP_DrVentEN_flg"
  VTHC_CLVentEN_flg/1 -> VTHC_CLVentEN_flg_Inproc/1  "VTHC_CLVentEN_flg"
  VTHC_CLVentEN_flg_Inproc/1 -> UnitConverter565/1
  UnitConverter565/1 -> VOUTP_CLVentEN_flg/1  "VOUTP_CLVentEN_flg"
  VTHC_PsVentEN_flg/1 -> VTHC_PsVentEN_flg_Inproc/1  "VTHC_PsVentEN_flg"
  VTHC_PsVentEN_flg_Inproc/1 -> UnitConverter566/1
  UnitConverter566/1 -> VOUTP_PsVentEN_flg/1  "VOUTP_PsVentEN_flg"
  VTHC_CRVentEN_flg/1 -> VTHC_CRVentEN_flg_Inproc/1  "VTHC_CRVentEN_flg"
  VTHC_CRVentEN_flg_Inproc/1 -> UnitConverter567/1
  UnitConverter567/1 -> VOUTP_CRVentEN_flg/1  "VOUTP_CRVentEN_flg"
  VTHC_FDCFGSAirIntSta_enum/1 -> VTHC_FDCFGSAirIntSta_enum_Inproc/1  "VTHC_FDCFGSAirIntSta_enum"
  VTHC_FDCFGSAirIntSta_enum_Inproc/1 -> UnitConverter568/1
  UnitConverter568/1 -> VOUTP_FDCFGSAirIntSta_enum/1  "VOUTP_FDCFGSAirIntSta_enum"
  VTHC_FDCFGSChSta_enum/1 -> VTHC_FDCFGSChSta_enum_Inproc/1  "VTHC_FDCFGSChSta_enum"
  VTHC_FDCFGSChSta_enum_Inproc/1 -> UnitConverter569/1
  UnitConverter569/1 -> VOUTP_FDCFGSChSta_enum/1  "VOUTP_FDCFGSChSta_enum"
  VTHC_FDCFGSAirIntCmd_enum/1 -> VTHC_FDCFGSAirIntCmd_enum_Inproc/1  "VTHC_FDCFGSAirIntCmd_enum"
  VTHC_FDCFGSAirIntCmd_enum_Inproc/1 -> UnitConverter570/1
  UnitConverter570/1 -> VOUTP_FDCFGSAirIntCmd_enum/1  "VOUTP_FDCFGSAirIntCmd_enum"
  VTHC_FDCFGSFuncSta_flg/1 -> VTHC_FDCFGSFuncSta_flg_Inproc/1  "VTHC_FDCFGSFuncSta_flg"
  VTHC_FDCFGSFuncSta_flg_Inproc/1 -> UnitConverter571/1
  UnitConverter571/1 -> VOUTP_FDCFGSFuncSta_flg/1  "VOUTP_FDCFGSFuncSta_flg"
  VTHC_FDCFGSChCmd_enum/1 -> VTHC_FDCFGSChCmd_enum_Inproc/1  "VTHC_FDCFGSChCmd_enum"
  VTHC_FDCFGSChCmd_enum_Inproc/1 -> UnitConverter572/1
  UnitConverter572/1 -> VOUTP_FDCFGSChCmd_enum/1  "VOUTP_FDCFGSChCmd_enum"
  VTHC_FDCFGSIONSWSta_flg/1 -> VTHC_FDCFGSIONSWSta_flg_Inproc/1  "VTHC_FDCFGSIONSWSta_flg"
  VTHC_FDCFGSIONSWSta_flg_Inproc/1 -> UnitConverter573/1
  UnitConverter573/1 -> VOUTP_FDCFGSIONSWSta_flg/1  "VOUTP_FDCFGSIONSWSta_flg"
  VTHC_FDCFGSIONCmd_flg/1 -> VTHC_FDCFGSIONCmd_flg_Inproc/1  "VTHC_FDCFGSIONCmd_flg"
  VTHC_FDCFGSIONCmd_flg_Inproc/1 -> UnitConverter574/1
  UnitConverter574/1 -> VOUTP_FDCFGSIONCmd_flg/1  "VOUTP_FDCFGSIONCmd_flg"
  VTHC_FDCFGSLearnCmd_enum/1 -> VTHC_FDCFGSLearnCmd_enum_Inproc/1  "VTHC_FDCFGSLearnCmd_enum"
  VTHC_FDCFGSLearnCmd_enum_Inproc/1 -> UnitConverter575/1
  UnitConverter575/1 -> VOUTP_FDCFGSLearnCmd_enum/1  "VOUTP_FDCFGSLearnCmd_enum"
  VTHC_FDCTHCMPreWPTCHeatSta_enum/1 -> VTHC_FDCTHCMPreWPTCHeatSta_enum_Inproc/1  "VTHC_FDCTHCMPreWPTCHeatSta_enum"
  VTHC_FDCTHCMPreWPTCHeatSta_enum_Inproc/1 -> UnitConverter576/1
  UnitConverter576/1 -> VOUTP_FDCTHCMPreWPTCHeatSta_enum/1  "VOUTP_FDCTHCMPreWPTCHeatSta_enum"
  VTPM_LFBatWarn_flg/1 -> VTPM_LFBatWarn_flg_Inproc/1  "VTPM_LFBatWarn_flg"
  VTPM_LFBatWarn_flg_Inproc/1 -> UnitConverter577/1
  UnitConverter577/1 -> VOUTP_LFBatWarn_flg/1  "VOUTP_LFBatWarn_flg"
  VTPM_RFBatWarn_flg/1 -> VTPM_RFBatWarn_flg_Inproc/1  "VTPM_RFBatWarn_flg"
  VTPM_RFBatWarn_flg_Inproc/1 -> UnitConverter578/1
  UnitConverter578/1 -> VOUTP_RFBatWarn_flg/1  "VOUTP_RFBatWarn_flg"
  VTPM_LRBatWarn_flg/1 -> VTPM_LRBatWarn_flg_Inproc/1  "VTPM_LRBatWarn_flg"
  VTPM_LRBatWarn_flg_Inproc/1 -> UnitConverter579/1
  UnitConverter579/1 -> VOUTP_LRBatWarn_flg/1  "VOUTP_LRBatWarn_flg"
  VTPM_RRBatWarn_flg/1 -> VTPM_RRBatWarn_flg_Inproc/1  "VTPM_RRBatWarn_flg"
  VTPM_RRBatWarn_flg_Inproc/1 -> UnitConverter580/1
  UnitConverter580/1 -> VOUTP_RRBatWarn_flg/1  "VOUTP_RRBatWarn_flg"
  VTPM_LFWheelPress_raw8/1 -> VTPM_LFWheelPress_raw8_Inproc/1  "VTPM_LFWheelPress_raw8"
  VTPM_LFWheelPress_raw8_Inproc/1 -> UnitConverter581/1
  UnitConverter581/1 -> VOUTP_LFWheelPress_raw8/1  "VOUTP_LFWheelPress_raw8"
  VTPM_RFWheelPress_raw8/1 -> VTPM_RFWheelPress_raw8_Inproc/1  "VTPM_RFWheelPress_raw8"
  VTPM_RFWheelPress_raw8_Inproc/1 -> UnitConverter582/1
  UnitConverter582/1 -> VOUTP_RFWheelPress_raw8/1  "VOUTP_RFWheelPress_raw8"
  VTPM_LRWheelPress_raw8/1 -> VTPM_LRWheelPress_raw8_Inproc/1  "VTPM_LRWheelPress_raw8"
  VTPM_LRWheelPress_raw8_Inproc/1 -> UnitConverter583/1
  UnitConverter583/1 -> VOUTP_LRWheelPress_raw8/1  "VOUTP_LRWheelPress_raw8"
  VTPM_RRWheelPress_raw8/1 -> VTPM_RRWheelPress_raw8_Inproc/1  "VTPM_RRWheelPress_raw8"
  VTPM_RRWheelPress_raw8_Inproc/1 -> UnitConverter584/1
  UnitConverter584/1 -> VOUTP_RRWheelPress_raw8/1  "VOUTP_RRWheelPress_raw8"
  VTPM_LFWheelTemp_C/1 -> VTPM_LFWheelTemp_C_Inproc/1  "VTPM_LFWheelTemp_C"
  VTPM_LFWheelTemp_C_Inproc/1 -> UnitConverter585/1
  UnitConverter585/1 -> VOUTP_LFWheelTemp_C/1  "VOUTP_LFWheelTemp_C"
  VTPM_RFWheelTemp_C/1 -> VTPM_RFWheelTemp_C_Inproc/1  "VTPM_RFWheelTemp_C"
  VTPM_RFWheelTemp_C_Inproc/1 -> UnitConverter586/1
  UnitConverter586/1 -> VOUTP_RFWheelTemp_C/1  "VOUTP_RFWheelTemp_C"
  VTPM_LRWheelTemp_C/1 -> VTPM_LRWheelTemp_C_Inproc/1  "VTPM_LRWheelTemp_C"
  VTPM_LRWheelTemp_C_Inproc/1 -> UnitConverter587/1
  UnitConverter587/1 -> VOUTP_LRWheelTemp_C/1  "VOUTP_LRWheelTemp_C"
  VTPM_RRWheelTemp_C/1 -> VTPM_RRWheelTemp_C_Inproc/1  "VTPM_RRWheelTemp_C"
  VTPM_RRWheelTemp_C_Inproc/1 -> UnitConverter588/1
  UnitConverter588/1 -> VOUTP_RRWheelTemp_C/1  "VOUTP_RRWheelTemp_C"
  VTPM_LFSensorFail_flg/1 -> VTPM_LFSensorFail_flg_Inproc/1  "VTPM_LFSensorFail_flg"
  VTPM_LFSensorFail_flg_Inproc/1 -> UnitConverter589/1
  UnitConverter589/1 -> VOUTP_LFSensorFail_flg/1  "VOUTP_LFSensorFail_flg"
  VTPM_RFSensorFail_flg/1 -> VTPM_RFSensorFail_flg_Inproc/1  "VTPM_RFSensorFail_flg"
  VTPM_RFSensorFail_flg_Inproc/1 -> UnitConverter590/1
  UnitConverter590/1 -> VOUTP_RFSensorFail_flg/1  "VOUTP_RFSensorFail_flg"
  VTPM_LRSensorFail_flg/1 -> VTPM_LRSensorFail_flg_Inproc/1  "VTPM_LRSensorFail_flg"
  VTPM_LRSensorFail_flg_Inproc/1 -> UnitConverter591/1
  UnitConverter591/1 -> VOUTP_LRSensorFail_flg/1  "VOUTP_LRSensorFail_flg"
  VTPM_RRSensorFail_flg/1 -> VTPM_RRSensorFail_flg_Inproc/1  "VTPM_RRSensorFail_flg"
  VTPM_RRSensorFail_flg_Inproc/1 -> UnitConverter592/1
  UnitConverter592/1 -> VOUTP_RRSensorFail_flg/1  "VOUTP_RRSensorFail_flg"
  VTPM_LFWheelDebug_flg/1 -> VTPM_LFWheelDebug_flg_Inproc/1  "VTPM_LFWheelDebug_flg"
  VTPM_LFWheelDebug_flg_Inproc/1 -> UnitConverter593/1
  UnitConverter593/1 -> VOUTP_LFWheelDebug_flg/1  "VOUTP_LFWheelDebug_flg"
  VTPM_LRWheelDebug_flg/1 -> VTPM_LRWheelDebug_flg_Inproc/1  "VTPM_LRWheelDebug_flg"
  VTPM_LRWheelDebug_flg_Inproc/1 -> UnitConverter594/1
  UnitConverter594/1 -> VOUTP_LRWheelDebug_flg/1  "VOUTP_LRWheelDebug_flg"
  VTPM_RFWheelDebug_flg/1 -> VTPM_RFWheelDebug_flg_Inproc/1  "VTPM_RFWheelDebug_flg"
  VTPM_RFWheelDebug_flg_Inproc/1 -> UnitConverter595/1
  UnitConverter595/1 -> VOUTP_RFWheelDebug_flg/1  "VOUTP_RFWheelDebug_flg"
  VTPM_RRWheelDebug_flg/1 -> VTPM_RRWheelDebug_flg_Inproc/1  "VTPM_RRWheelDebug_flg"
  VTPM_RRWheelDebug_flg_Inproc/1 -> UnitConverter596/1
  UnitConverter596/1 -> VOUTP_RRWheelDebug_flg/1  "VOUTP_RRWheelDebug_flg"
  VTPM_TPMSResButtAllow_flg/1 -> VTPM_TPMSResButtAllow_flg_Inproc/1  "VTPM_TPMSResButtAllow_flg"
  VTPM_TPMSResButtAllow_flg_Inproc/1 -> UnitConverter597/1
  UnitConverter597/1 -> VOUTP_TPMSResButtAllow_flg/1  "VOUTP_TPMSResButtAllow_flg"
  VTPM_TPMSCaliButtAllow_flg/1 -> VTPM_TPMSCaliButtAllow_flg_Inproc/1  "VTPM_TPMSCaliButtAllow_flg"
  VTPM_TPMSCaliButtAllow_flg_Inproc/1 -> UnitConverter598/1
  UnitConverter598/1 -> VOUTP_TPMSCaliButtAllow_flg/1  "VOUTP_TPMSCaliButtAllow_flg"
  VTPM_LFPressIndi_enum/1 -> VTPM_LFPressIndi_enum_Inproc/1  "VTPM_LFPressIndi_enum"
  VTPM_LFPressIndi_enum_Inproc/1 -> UnitConverter599/1
  UnitConverter599/1 -> VOUTP_LFPressIndi_enum/1  "VOUTP_LFPressIndi_enum"
  VTPM_RFPressIndi_enum/1 -> VTPM_RFPressIndi_enum_Inproc/1  "VTPM_RFPressIndi_enum"
  VTPM_RFPressIndi_enum_Inproc/1 -> UnitConverter600/1
  UnitConverter600/1 -> VOUTP_RFPressIndi_enum/1  "VOUTP_RFPressIndi_enum"
  VTPM_LRPressIndi_enum/1 -> VTPM_LRPressIndi_enum_Inproc/1  "VTPM_LRPressIndi_enum"
  VTPM_LRPressIndi_enum_Inproc/1 -> UnitConverter601/1
  UnitConverter601/1 -> VOUTP_LRPressIndi_enum/1  "VOUTP_LRPressIndi_enum"
  VTPM_RRPressIndi_enum/1 -> VTPM_RRPressIndi_enum_Inproc/1  "VTPM_RRPressIndi_enum"
  VTPM_RRPressIndi_enum_Inproc/1 -> UnitConverter602/1
  UnitConverter602/1 -> VOUTP_RRPressIndi_enum/1  "VOUTP_RRPressIndi_enum"
  VTPM_TPMSWarnIndi_enum/1 -> VTPM_TPMSWarnIndi_enum_Inproc/1  "VTPM_TPMSWarnIndi_enum"
  VTPM_TPMSWarnIndi_enum_Inproc/1 -> UnitConverter603/1
  UnitConverter603/1 -> VOUTP_TPMSWarnIndi_enum/1  "VOUTP_TPMSWarnIndi_enum"
  VTPM_LFWheelTmpIndi_flg/1 -> VTPM_LFWheelTmpIndi_flg_Inproc/1  "VTPM_LFWheelTmpIndi_flg"
  VTPM_LFWheelTmpIndi_flg_Inproc/1 -> UnitConverter604/1
  UnitConverter604/1 -> VOUTP_LFWheelTmpIndi_flg/1  "VOUTP_LFWheelTmpIndi_flg"
  VTPM_RFWheelTmpIndi_flg/1 -> VTPM_RFWheelTmpIndi_flg_Inproc/1  "VTPM_RFWheelTmpIndi_flg"
  VTPM_RFWheelTmpIndi_flg_Inproc/1 -> UnitConverter605/1
  UnitConverter605/1 -> VOUTP_RFWheelTmpIndi_flg/1  "VOUTP_RFWheelTmpIndi_flg"
  VTPM_LRWheelTmpIndi_flg/1 -> VTPM_LRWheelTmpIndi_flg_Inproc/1  "VTPM_LRWheelTmpIndi_flg"
  VTPM_LRWheelTmpIndi_flg_Inproc/1 -> UnitConverter606/1
  UnitConverter606/1 -> VOUTP_LRWheelTmpIndi_flg/1  "VOUTP_LRWheelTmpIndi_flg"
  VTPM_RRWheelTmpIndi_flg/1 -> VTPM_RRWheelTmpIndi_flg_Inproc/1  "VTPM_RRWheelTmpIndi_flg"
  VTPM_RRWheelTmpIndi_flg_Inproc/1 -> UnitConverter607/1
  UnitConverter607/1 -> VOUTP_RRWheelTmpIndi_flg/1  "VOUTP_RRWheelTmpIndi_flg"
  VTPM_LFWheelPSW_raw8/1 -> VTPM_LFWheelPSW_raw8_Inproc/1  "VTPM_LFWheelPSW_raw8"
  VTPM_LFWheelPSW_raw8_Inproc/1 -> UnitConverter608/1
  UnitConverter608/1 -> VOUTP_LFWheelPSW_raw8/1  "VOUTP_LFWheelPSW_raw8"
  VTPM_LRWheelPSW_raw8/1 -> VTPM_LRWheelPSW_raw8_Inproc/1  "VTPM_LRWheelPSW_raw8"
  VTPM_LRWheelPSW_raw8_Inproc/1 -> UnitConverter609/1
  UnitConverter609/1 -> VOUTP_LRWheelPSW_raw8/1  "VOUTP_LRWheelPSW_raw8"
